simulink model "Adaptive_CT_ur10v"  (R2021b)
(part 15 of 20)

t4990 = ct{1900};
t4992 = ct{1901};
t4993 = ct{1902};
t4997 = ct{1903};
t4d = ct{1904};
t4dd = ct{1905};
t50 = ct{1906};
t5000 = ct{1907};
t5001 = ct{1908};
t5002 = ct{1909};
t5006 = ct{1910};
t501 = ct{1911};
t5010 = ct{1912};
t5011 = ct{1913};
t5012 = ct{1914};
t5013 = ct{1915};
t5014 = ct{1916};
t5018 = ct{1917};
t5019 = ct{1918};
t5020 = ct{1919};
t5022 = ct{1920};
t5025 = ct{1921};
t5026 = ct{1922};
t503 = ct{1923};
t5030 = ct{1924};
t5032 = ct{1925};
t5038 = ct{1926};
t5039 = ct{1927};
t5040 = ct{1928};
t5041 = ct{1929};
t5043 = ct{1930};
t5044 = ct{1931};
t5045 = ct{1932};
t5046 = ct{1933};
t5047 = ct{1934};
t5048 = ct{1935};
t5049 = ct{1936};
t5050 = ct{1937};
t5051 = ct{1938};
t5056 = ct{1939};
t5057 = ct{1940};
t5062 = ct{1941};
t5069 = ct{1942};
t5070 = ct{1943};
t5074 = ct{1944};
t5078 = ct{1945};
t508 = ct{1946};
t5081 = ct{1947};
t5092 = ct{1948};
t5093 = ct{1949};
t5096 = ct{1950};
t5097 = ct{1951};
t5098 = ct{1952};
t51 = ct{1953};
t5102 = ct{1954};
t5104 = ct{1955};
t5111 = ct{1956};
t5112 = ct{1957};
t5117 = ct{1958};
t5119 = ct{1959};
t5120 = ct{1960};
t5123 = ct{1961};
t5124 = ct{1962};
t5126 = ct{1963};
t5130 = ct{1964};
t5131 = ct{1965};
t5132 = ct{1966};
t5137 = ct{1967};
t5138 = ct{1968};
t514 = ct{1969};
t5144 = ct{1970};
t5148 = ct{1971};
t5149 = ct{1972};
t515 = ct{1973};
t5151 = ct{1974};
t5155 = ct{1975};
t5158 = ct{1976};
t516 = ct{1977};
t5163 = ct{1978};
t5165 = ct{1979};
t5167 = ct{1980};
t5170 = ct{1981};
t5171 = ct{1982};
t5175 = ct{1983};
t5176 = ct{1984};
t5180 = ct{1985};
t5181 = ct{1986};
t5182 = ct{1987};
t5185 = ct{1988};
t5186 = ct{1989};
t5188 = ct{1990};
t519 = ct{1991};
t5200 = ct{1992};
t5201 = ct{1993};
t5202 = ct{1994};
t5203 = ct{1995};
t5206 = ct{1996};
t5213 = ct{1997};
t5215 = ct{1998};
t5219 = ct{1999};
t5224 = ct{2000};
t5226 = ct{2001};
t523 = ct{2002};
t524 = ct{2003};
t5255 = ct{2004};
t5256 = ct{2005};
t5257 = ct{2006};
t5259 = ct{2007};
t5260 = ct{2008};
t5267 = ct{2009};
t5269 = ct{2010};
t5279 = ct{2011};
t5280 = ct{2012};
t5283 = ct{2013};
t5286 = ct{2014};
t5287 = ct{2015};
t529 = ct{2016};
t5292 = ct{2017};
t5295 = ct{2018};
t5296 = ct{2019};
t5297 = ct{2020};
t53 = ct{2021};
t530 = ct{2022};
t5305 = ct{2023};
t5306 = ct{2024};
t5315 = ct{2025};
t532 = ct{2026};
t5323 = ct{2027};
t5324 = ct{2028};
t5327 = ct{2029};
t5328 = ct{2030};
t5349 = ct{2031};
t5351 = ct{2032};
t5353 = ct{2033};
t5355 = ct{2034};
t5356 = ct{2035};
t5359 = ct{2036};
t5368 = ct{2037};
t537 = ct{2038};
t5370 = ct{2039};
t5375 = ct{2040};
t5397 = ct{2041};
t5401 = ct{2042};
t5403 = ct{2043};
t5413 = ct{2044};
t543 = ct{2045};
t5438 = ct{2046};
t544 = ct{2047};
t546 = ct{2048};
t5465 = ct{2049};
t547 = ct{2050};
t5478 = ct{2051};
t548 = ct{2052};
t5482 = ct{2053};
t55 = ct{2054};
t5503 = ct{2055};
t5505 = ct{2056};
t5514 = ct{2057};
t5515 = ct{2058};
t5517 = ct{2059};
t552 = ct{2060};
t5523 = ct{2061};
t553 = ct{2062};
t554 = ct{2063};
t56 = ct{2064};
t5619 = ct{2065};
t562 = ct{2066};
t569 = ct{2067};
t57 = ct{2068};
t570 = ct{2069};
t58 = ct{2070};
t582 = ct{2071};
t588 = ct{2072};
t589 = ct{2073};
t591 = ct{2074};
t593 = ct{2075};
t598 = ct{2076};
t5d = ct{2077};
t5dd = ct{2078};
t601 = ct{2079};
t602 = ct{2080};
t604 = ct{2081};
t608 = ct{2082};
t609 = ct{2083};
t61 = ct{2084};
t612 = ct{2085};
t614 = ct{2086};
t615 = ct{2087};
t616 = ct{2088};
t617 = ct{2089};
t623 = ct{2090};
t627 = ct{2091};
t63 = ct{2092};
t632 = ct{2093};
t634 = ct{2094};
t635 = ct{2095};
t637 = ct{2096};
t639 = ct{2097};
t641 = ct{2098};
t645 = ct{2099};
t646 = ct{2100};
t647 = ct{2101};
t648 = ct{2102};
t649 = ct{2103};
t650 = ct{2104};
t652 = ct{2105};
t653 = ct{2106};
t655 = ct{2107};
t659 = ct{2108};
t664 = ct{2109};
t670 = ct{2110};
t675 = ct{2111};
t680 = ct{2112};
t682 = ct{2113};
t687 = ct{2114};
t69 = ct{2115};
t694 = ct{2116};
t695 = ct{2117};
t696 = ct{2118};
t698 = ct{2119};
t699 = ct{2120};
t6d = ct{2121};
t6dd = ct{2122};
t703 = ct{2123};
t705 = ct{2124};
t706 = ct{2125};
t71 = ct{2126};
t711 = ct{2127};
t712 = ct{2128};
t713 = ct{2129};
t720 = ct{2130};
t721 = ct{2131};
t723 = ct{2132};
t726 = ct{2133};
t729 = ct{2134};
t731 = ct{2135};
t732 = ct{2136};
t733 = ct{2137};
t735 = ct{2138};
t736 = ct{2139};
t738 = ct{2140};
t739 = ct{2141};
t745 = ct{2142};
t746 = ct{2143};
t747 = ct{2144};
t748 = ct{2145};
t75 = ct{2146};
t752 = ct{2147};
t755 = ct{2148};
t759 = ct{2149};
t760 = ct{2150};
t761 = ct{2151};
t763 = ct{2152};
t764 = ct{2153};
t775 = ct{2154};
t776 = ct{2155};
t781 = ct{2156};
t785 = ct{2157};
t788 = ct{2158};
t789 = ct{2159};
t793 = ct{2160};
t8 = ct{2161};
t802 = ct{2162};
t806 = ct{2163};
t82 = ct{2164};
t820 = ct{2165};
t824 = ct{2166};
t828 = ct{2167};
t831 = ct{2168};
t832 = ct{2169};
t833 = ct{2170};
t838 = ct{2171};
t842 = ct{2172};
t843 = ct{2173};
t844 = ct{2174};
t846 = ct{2175};
t853 = ct{2176};
t855 = ct{2177};
t859 = ct{2178};
t861 = ct{2179};
t865 = ct{2180};
t870 = ct{2181};
t871 = ct{2182};
t873 = ct{2183};
t879 = ct{2184};
t880 = ct{2185};
t884 = ct{2186};
t885 = ct{2187};
t890 = ct{2188};
t892 = ct{2189};
t896 = ct{2190};
t897 = ct{2191};
t9 = ct{2192};
t900 = ct{2193};
t909 = ct{2194};
t910 = ct{2195};
t919 = ct{2196};
t922 = ct{2197};
t923 = ct{2198};
t927 = ct{2199};
t928 = ct{2200};
t930 = ct{2201};
t932 = ct{2202};
t937 = ct{2203};
t943 = ct{2204};
t944 = ct{2205};
t949 = ct{2206};
t952 = ct{2207};
t959 = ct{2208};
t961 = ct{2209};
t962 = ct{2210};
t963 = ct{2211};
t964 = ct{2212};
t965 = ct{2213};
t966 = ct{2214};
t969 = ct{2215};
t970 = ct{2216};
t972 = ct{2217};
t973 = ct{2218};
t981 = ct{2219};
t982 = ct{2220};
t983 = ct{2221};
t986 = ct{2222};
t989 = ct{2223};
t992 = ct{2224};
t999 = ct{2225};
t2236 = t2186./2.0;
t2237 = t2187./2.0;
t2238 = t2188./2.0;
t2239 = t2191./2.0;
t2285 = -t2269;
t2350 = t2290./2.0;
t2360 = t2310./2.0;
t2362 = -t2328;
t2466 = -t2445;
t2468 = -t2446;
t2561 = -t2545;
t2564 = t14.*t2510;
t2567 = t8.*t2514;
t2597 = -t2563;
t2601 = -t2568;
t2603 = -t2570;
t2612 = t2563./2.0;
t2616 = t2568./2.0;
t2637 = t8.*t37.*t2510;
t2643 = t14.*t37.*t2514;
t2668 = t2640./2.0;
t2669 = t2641./2.0;
t2758 = t2733.*t1dd;
t2786 = t2763.*t2d;
t2787 = t2763.*t3d;
t2788 = t2763.*t4d;
t2805 = t1392+t1748;
t2809 = t37.*t2733;
t2814 = t39.*t2733;
t2874 = -t2832;
t2887 = -t2845;
t2890 = -t2861;
t2904 = t2845./2.0;
t2906 = t2847./2.0;
t2908 = t2851./2.0;
t2909 = t1457+t1787;
t2931 = t37.*t2811;
t2958 = -t2926;
t2962 = t2930.*t1d;
t2963 = t18.*t39.*t2811;
t2973 = t2926./2.0;
t2984 = -t2957;
t2993 = -t2981;
t3084 = t3048./2.0;
t3094 = t3057.*t6d;
t3109 = t3075./2.0;
t3133 = t8.*t3089;
t3144 = -t3113;
t3164 = t3113./2.0;
t3167 = t3115./2.0;
t3184 = -t3157;
t3186 = -t3141;
t3188 = -t3142;
t3199 = t3135./2.0;
t3201 = t3138./2.0;
t3202 = t3141./2.0;
t3203 = t3142./2.0;
t3209 = -t3170;
t3210 = -t3171;
t3211 = -t3172;
t3216 = t3191.*t5d;
t3217 = -t3200;
t3218 = t3155./2.0;
t3225 = -t3206;
t3227 = t3173./2.0;
t3229 = t14.*t39.*t3089;
t3233 = t3180./2.0;
t3248 = -t3226;
t3254 = t3212./2.0;
t3269 = -t3247;
t3270 = t3249.*t1d;
t3273 = -t3252;
t3279 = -t3255;
t3280 = t3264.*(-1.0./2.0);
t3281 = t3243./2.0;
t3284 = t3247./2.0;
t3287 = t3252./2.0;
t3293 = t3255./2.0;
t3294 = -t3263;
t3297 = -t3286;
t3301 = -t3290;
t3304 = t3263./2.0;
t3309 = t3274./2.0;
t3311 = t3277./2.0;
t3314 = -t3300;
t3320 = t255.*t3089;
t3324 = t3300./2.0;
t3334 = -t3325;
t3344 = t3328.*t1dd;
t3362 = -t3350;
t3364 = t3338./2.0;
t3372 = t1978+t2036;
t3373 = -t3352;
t3379 = t39.*t3328;
t3382 = t3352./2.0;
t3385 = t37.*t3328;
t3386 = t37.*t3329;
t3389 = t3371.*t1d;
t3394 = -t3370;
t3397 = -t3374;
t3398 = t3375.*t1d;
t3402 = t3370./2.0;
t3406 = t3374./2.0;
t3410 = t3376./2.0;
t3412 = t18.*t39.*t3329;
t3419 = -t3395;
t3427 = t3392./2.0;
t3430 = t3395./2.0;
t3462 = -t3442;
t3486 = t3450.*t1d;
t3492 = -t3476;
t3497 = -t3482;
t3501 = t3476./2.0;
t3507 = t3482./2.0;
t3514 = t3489./2.0;
t3519 = t3494./2.0;
t3541 = t3512./2.0;
t3542 = -t3529;
t3561 = -t3535;
t3566 = t3533./2.0;
t3570 = t3535./2.0;
t3576 = -t3554;
t3592 = t18.*t3548;
t3594 = t18.*t3552;
t3595 = t664+t1836+t1848;
t3597 = t3552./2.0;
t3599 = t3554./2.0;
t3618 = t3572./2.0;
t3645 = -t3619;
t3646 = t3608./2.0;
t3652 = t3619./2.0;
t3654 = t3621./2.0;
t3656 = -t3633;
t3657 = t3641.*t1d;
t3658 = t3642.*t6d;
t3659 = -t3643;
t3660 = t3631./2.0;
t3663 = t3632./2.0;
t3664 = t3633./2.0;
t3672 = t3643./2.0;
t3689 = t3653./2.0;
t3691 = t3655./2.0;
t3692 = t3666.*t1d;
t3695 = t18.*t3669;
t3696 = -t3671;
t3698 = t3662./2.0;
t3700 = t3665./2.0;
t3703 = -t3679;
t3705 = t1053+t3092;
t3706 = t1054+t3093;
t3707 = t3667./2.0;
t3711 = t3671./2.0;
t3713 = t3673./2.0;
t3717 = t3679./2.0;
t3718 = t3680./2.0;
t3723 = -t3702;
t3735 = t3694./2.0;
t3742 = t3702./2.0;
t3759 = t3719./2.0;
t3773 = -t3749;
t3782 = (t8.*t3709)./2.0;
t3790 = t3749./2.0;
t3793 = -t3772;
t3797 = t14.*t39.*t3709;
t3798 = -t3788;
t3801 = t3772./2.0;
t3816 = -t3795;
t3823 = -t3802;
t3824 = t3795./2.0;
t3834 = t3802./2.0;
t3836 = -t3815;
t3844 = t3815./2.0;
t3847 = t3818./2.0;
t3856 = t3825./2.0;
t3859 = t3829./2.0;
t3862 = t2160+t2575;
t3865 = -t3841;
t3870 = (t14.*t3799)./2.0;
t3873 = t3841./2.0;
t3881 = t8.*t39.*t3799;
t3884 = t2159+t2605;
t3898 = -t3868;
t3909 = t3868./2.0;
t3911 = t255.*t3709;
t3915 = -t3882;
t3916 = -t3899;
t3925 = -t3908;
t3930 = t3882./2.0;
t3945 = -t3912;
t3951 = -t3934;
t3953 = t3904./2.0;
t3955 = -t3938;
t3961 = t3912./2.0;
t3981 = t3942./2.0;
t3985 = -t3971;
t3995 = t3964./2.0;
t3996 = t3966./2.0;
t3998 = t3969./2.0;
t4000 = -t3991;
t4013 = -t4008;
t4015 = t330.*t3799;
t4031 = t4020.*t2d;
t4032 = t4020.*t3d;
t4033 = t4020.*t4d;
t4037 = -t4022;
t4039 = t4022./2.0;
t4043 = -t4036;
t4051 = t4036./2.0;
t4060 = -t4057;
t4062 = t4054.*t1d;
t4079 = -t4070;
t4100 = t4092.*t1d;
t4104 = t18.*t4093;
t4105 = t18.*t4094;
t4106 = -t4094;
t4110 = t4093./2.0;
t4111 = t4094./2.0;
t4181 = t4161./2.0;
t4184 = t4163./2.0;
t4205 = t4197.*t1d;
t4209 = t4190./2.0;
t4210 = t4191./2.0;
t4211 = t4198.*t1d;
t4232 = t8.*t4206;
t4234 = -t4213;
t4239 = t4213./2.0;
t4240 = t4214./2.0;
t4244 = t14.*t4218;
t4247 = t4223./2.0;
t4250 = t4224./2.0;
t4259 = t4235./2.0;
t4261 = -t4242;
t4264 = -t4246;
t4265 = t4238./2.0;
t4269 = t4241./2.0;
t4270 = t4242./2.0;
t4271 = t4243./2.0;
t4272 = t4258.*t5d;
t4275 = t4246./2.0;
t4277 = t4249./2.0;
t4278 = t14.*t39.*t4206;
t4279 = t4254.*t2d;
t4280 = t4254.*t3d;
t4281 = t4254.*t4d;
t4286 = t4253./2.0;
t4291 = t4260./2.0;
t4300 = t8.*t39.*t4218;
t4306 = t4284./2.0;
t4307 = t4285./2.0;
t4308 = -t4292;
t4315 = t4292./2.0;
t4316 = t4293./2.0;
t4318 = t4295./2.0;
t4320 = t4298./2.0;
t4323 = t4303./2.0;
t4338 = t4311./2.0;
t4339 = t4319./2.0;
t4343 = t255.*t4206;
t4345 = -t4336;
t4347 = t4328./2.0;
t4350 = t4336./2.0;
t4352 = t4341.*t1d;
t4369 = t330.*t4218;
t4370 = t4360.*t1d;
t4373 = t18.*t4363;
t4374 = -t4366;
t4375 = t4358./2.0;
t4376 = t4359./2.0;
t4377 = t4363./2.0;
t4378 = t4364./2.0;
t4387 = t18.*t4364.*(-1.0./2.0);
t4390 = t4388.*t2d;
t4391 = t4388.*t3d;
t4392 = t4388.*t4d;
t4400 = -t4396;
t4401 = t2546+t3450;
t4412 = -t4407;
t4415 = t4407./2.0;
t4419 = t4411./2.0;
t4422 = t3048+t3075;
t4435 = t4423.*t2dd;
t4437 = t4423.*t3dd;
t4439 = t4423.*t4dd;
t4441 = t4420./2.0;
t4446 = -t4432;
t4455 = t4432./2.0;
t4456 = t4433./2.0;
t4462 = t14.*t4452;
t4463 = t8.*t4453;
t4465 = t4445./2.0;
t4481 = -t4476;
t4484 = t8.*t39.*t4452;
t4485 = t14.*t39.*t4453;
t4490 = t37.*t4474;
t4492 = t3155+t3158;
t4498 = t18.*t39.*t4474;
t4505 = t1682+t1722+t2002+t2015;
t4511 = t255.*t4453;
t4516 = t330.*t4452;
t4520 = t4514.*t1d;
t4521 = t4515./2.0;
t4522 = -t4517;
t4527 = t4519./2.0;
t4530 = t2187+t2534+t2566;
t4535 = -t4154.*(t745-t747);
t4545 = t4154.*(t745-t747);
t4555 = t4546.*(-1.0./2.0);
t4559 = t4546./2.0;
t4564 = -t4562;
t4567 = -t4565;
t4569 = t4565./2.0;
t4571 = (t1874.*t4154)./2.0;
t4577 = t4568./2.0;
t4586 = -t4576;
t4590 = t14.*t4578;
t4593 = t4576./2.0;
t4594 = t8.*t4575;
t4601 = -t4588;
t4603 = t8.*t4587;
t4605 = t4583./2.0;
t4609 = t4588./2.0;
t4616 = t4611.*t2d;
t4617 = t4611.*t3d;
t4618 = t4611.*t4d;
t4625 = -t4621;
t4630 = t4622.*t1d;
t4637 = -t2d.*(t3350-t3369);
t4638 = -t3d.*(t3350-t3369);
t4639 = -t4d.*(t3350-t3369);
t4644 = -t4636;
t4649 = -t4634;
t4651 = -t4646;
t4653 = t1899+t1900+t1901+t2328;
t4656 = t4634./2.0;
t4657 = t4635./2.0;
t4658 = -t4650;
t4661 = t4654.*t2d;
t4662 = t4654.*t3d;
t4663 = t4654.*t4d;
t4674 = t2270.*t4154;
t4689 = -t4685;
t4690 = -t2d.*(t3442+(t14.*(t1864-t2028))./2.0);
t4691 = -t3d.*(t3442+(t14.*(t1864-t2028))./2.0);
t4692 = -t4d.*(t3442+(t14.*(t1864-t2028))./2.0);
t4709 = -t4702;
t4711 = t4701./2.0;
t4712 = t4702./2.0;
t4726 = t4717./2.0;
t4731 = t4723./2.0;
t4733 = t2934+t4034;
t4734 = t4724./2.0;
t4735 = t37.*t4710;
t4736 = t4725./2.0;
t4740 = t2529.*t4154;
t4745 = t18.*t39.*t4710;
t4748 = t4730./2.0;
t4752 = t4741./2.0;
t4754 = t4744./2.0;
t4755 = t2918+t4056;
t4761 = -t1d.*(t2893-t4056);
t4769 = -t4427.*(t745-t747);
t4772 = t4766.*(-1.0./2.0);
t4773 = t2914+t4083;
t4774 = t201+t332+t1382+t1397+t1654+t1660+t2108;
t4782 = t4427.*(t745-t747).*(-1.0./2.0);
t4788 = -t4784;
t4793 = t14.*t4777;
t4797 = t3572+t3621;
t4816 = t8.*t39.*t4777;
t4824 = (t1874.*t4427)./2.0;
t4826 = t8.*t4810;
t4833 = -t4830;
t4839 = t14.*t39.*t4810;
t4850 = t330.*t4777;
t4857 = t255.*t4810;
t4868 = t2270.*t4427;
t4872 = t3081.*t4154;
t4877 = -t4873;
t4879 = t4154.*(t503.*1.383e-1+t731+t981+t999);
t4892 = -t4890;
t4894 = t3810+t3829;
t4897 = t2529.*t4427;
t4900 = -t4898;
t4902 = t4898./2.0;
t4913 = t2132+t2162+t2591+t2604;
t4914 = t2150+t2196+t2552+t2573;
t4916 = t3868+t3896;
t4933 = (t3404.*t4154)./2.0;
t4936 = -t4934;
t4947 = -t4942;
t4948 = -t4943;
t4962 = t2810+t3112+t3193;
t4968 = t2773+t2871+t3527;
t4969 = t3081.*t4427;
t4971 = t3734.*t4154;
t4977 = t4427.*(t503.*1.383e-1+t731+t981+t999);
t4978 = t2812+t2875+t3565;
t4983 = t3821.*t4154;
t4991 = -t4984;
t4995 = t4984./2.0;
t4996 = t2851+t3275+t3278;
t5005 = t1249+t1458+t1507+t3005+t3006;
t5016 = -t5d.*(-t2972+t3286+(t8.*t39.*(t1743-t1783))./2.0);
t5017 = t5d.*(-t2972+t3286+(t8.*t39.*(t1743-t1783))./2.0);
t5021 = t3404.*t4427;
t5028 = t5022./2.0;
t5031 = t4049.*t4154;
t5034 = -t5032;
t5037 = t1537+t2024+t2678+t3921;
t5042 = t1904+t2419+t2536+t3600;
t5053 = t37.*t5039;
t5054 = t8.*t5045;
t5055 = t14.*t5046;
t5058 = t2329+t2791+t2792+t2793;
t5061 = t18.*t39.*t5039;
t5063 = t14.*t5049;
t5064 = t8.*t5050;
t5066 = t5062.*(-1.0./2.0);
t5068 = (t3686.*t4427)./2.0;
t5071 = -t1d.*(-t1590+t2042+t3934+(t18.*t37.*(t544-t1021+t330.*(t100-t364)))./2.0);
t5076 = t3734.*t4427;
t5077 = (t4130.*t4154)./2.0;
t5079 = t1572+t2072+t2710+t3986;
t5084 = -t5078;
t5100 = t5096./2.0;
t5105 = -t5102;
t5107 = -t5d.*(-t612-t944+t1336+t2229+t2811+(t8.*t494.*(t100-t364))./2.0+(t14.*t39.*(t844-t1156))./2.0);
t5109 = t5102./2.0;
t5113 = t5d.*(-t612-t944+t1336+t2229+t2811+(t8.*t494.*(t100-t364))./2.0+(t14.*t39.*(t844-t1156))./2.0);
t5121 = t14.*t5111;
t5122 = t14.*t5112;
t5125 = t635+t1428+t1833+t1846+t2789+t2927;
t5127 = t5124.*(-1.0./2.0);
t5139 = -t5137;
t5142 = t5130./2.0;
t5143 = t5138.*t5d;
t5145 = t8.*t39.*t5111;
t5146 = t8.*t39.*t5112;
t5153 = -t5149;
t5159 = -t5155;
t5162 = t5158.*(-1.0./2.0);
t5164 = t4154.*t4333;
t5169 = -t5165;
t5173 = t5165./2.0;
t5174 = t5170.*(-1.0./2.0);
t5179 = t4049.*t4427;
t5183 = t330.*t5111;
t5184 = t330.*t5112;
t5190 = -t5188;
t5204 = t713+t1489+t1849+t1959+t2940+t3028;
t5207 = t5203.*t5d;
t5209 = t5206.*t5d;
t5214 = t4154.*t4427;
t5217 = -t5215;
t5221 = t2321+t2385+t4710;
t5222 = t2304+t2368+t4732;
t5225 = t4333.*t4427;
t5228 = t5226./2.0;
t5230 = -t6d.*(t680-t989+t1395-t2455+t3328+(t627.*(t101-t401))./2.0+(t330.*(t952-t1028))./2.0);
t5231 = t6d.*(t680-t989+t1395-t2455+t3328+(t627.*(t101-t401))./2.0+(t330.*(t952-t1028))./2.0);
t5234 = t2491+t2493+t3493+t3494;
t5235 = t2491+t2493+t3489+t3490;
t5243 = t4403+t4411;
t5261 = -t5259;
t5262 = t5259./2.0;
t5263 = -t5260;
t5266 = t5260./2.0;
t5268 = t1789+t1814+t5039;
t5271 = t5269.*t1d;
t5276 = t1478+t1707+t1724+t2898+t3179+t3213;
t5282 = t5279.*t5d;
t5284 = t5280./2.0;
t5288 = -t5286;
t5291 = t5286./2.0;
t5293 = t5287./2.0;
t5299 = t5295./2.0;
t5303 = t5296./2.0;
t5304 = t5297./2.0;
t5307 = t5305./2.0;
t5311 = t501+t2764+t2765+t2766+t4312;
t5314 = -t5306;
t5322 = t5306./2.0;
t5325 = -t6d.*(t682+t1513-t1939+t1985-t2734-t2988+(t330.*(t582+t616-t761+t18.*t37.*(t100-t364)))./2.0);
t5329 = t6d.*(t682+t1513-t1939+t1985-t2734-t2988+(t330.*(t582+t616-t761+t18.*t37.*(t100-t364)))./2.0);
t5330 = t711+t1514+t1936+t2010+t2733+t3037+t3050;
t5335 = t5328.*t2d;
t5336 = t5328.*t3d;
t5337 = t5328.*t4d;
t5345 = t1863+t1868+t5180;
t5346 = t245+t2800+t2801+t2802+t4372;
t5352 = t964+t1903+t2367+t2403+t3540+t3581;
t5357 = t5356.*(-1.0./2.0);
t5358 = t2894+t2950+t4040+t4052;
t5361 = t1004+t2004+t2366+t2475+t3651+t3699;
t5362 = -t1d.*(t2933-t4040-t4052+(t342.*(t544-t1021+t330.*(t100-t364)))./2.0);
t5363 = t1d.*(t2933-t4040-t4052+(t342.*(t544-t1021+t330.*(t100-t364)))./2.0);
t5366 = t3032+t3043+t4970;
t5369 = t14.*t5368;
t5373 = t8.*t5370;
t5374 = t8.*t39.*t5368;
Y = ft_10({t100,t1007,t101,t1015,t1016,t1017,t1021,t1026,t1028,t1031,t1035,t1036,t104,t1044,t1045,t1046,t1047,t1048,t1049,t1055,t106,t1066,t1068,t1069,t107,t1070,t1071,t1079,t108,t1080,t1081,t1082,t1083,t1084,t1085,t1086,t1087,t1093,t1094,t1096,t1097,t1098,t1106,t1108,t1109,t111,t1110,t112,t1121,t1122,t1123,t1126,t1128,t1129,t113,t1133,t1134,t1135,t1137,t1138,t1139,t1140,t1147,t1148,t1155,t1156,t1160,t1162,t1172,t1174,t1183,t1184,t1185,t1186,t1187,t1189,t1193,t1196,t12,t1203,t1208,t1209,t1210,t1211,t1222,t1224,t1225,t1226,t1227,t1230,t1236,t1237,t1238,t124,t1245,t1246,t1247,t1248,t1264,t1265,t1266,t1268,t127,t1271,t1272,t1273,t128,t1281,t1284,t1287,t1288,t1289,t1297,t1298,t13,t1302,t131,t1311,t1312,t1316,t1317,t132,t1321,t1328,t1331,t1332,t1333,t1334,t1335,t134,t1355,t1356,t1357,t1358,t136,t1368,t137,t1375,t1378,t138,t1399,t14,t1400,t1403,t1408,t1410,t1413,t1419,t1420,t1427,t1434,t1440,t1461,t1464,t1465,t1468,t1470,t1472,t1475,t1479,t1485,t1492,t1497,t1499,t15,t150,t1500,t1501,t1503,t1504,t1516,t1517,t1518,t1519,t152,t1520,t1521,t1525,t1526,t1528,t1529,t1532,t1534,t1535,t1536,t1537,t1547,t155,t156,t1569,t1571,t1574,t1578,t1579,t158,t1580,t1585,t1586,t1588,t1589,t159,t1590,t1597,t1599,t1606,t1607,t1609,t1610,t1615,t1617,t1618,t162,t163,t1636,t164,t1645,t1647,t1648,t1649,t165,t1650,t1651,t1652,t1653,t1659,t1663,t1671,t1674,t1677,t1678,t1680,t1683,t1685,t1686,t1687,t1692,t1699,t1701,t1704,t1706,t1709,t171,t1710,t1713,t1714,t1715,t173,t1733,t1736,t1738,t174,t1740,t1741,t1742,t1743,t175,t1751,t1754,t1755,t1758,t1759,t1760,t177,t1776,t1780,t1783,t1784,t1786,t1790,t1792,t1797,t1799,t18,t1800,t1803,t1807,t1813,t1815,t1816,t1818,t1827,t1829,t1832,t1835,t1837,t1838,t1840,t1844,t1848,t1849,t1862,t1864,t1866,t1867,t187,t1872,t1873,t1874,t1875,t1885,t1888,t1889,t1890,t1891,t1892,t19,t1903,t1905,t191,t1916,t1919,t1920,t1921,t1925,t1929,t1930,t1933,t1935,t1938,t1939,t1940,t1944,t1945,t1956,t1957,t1958,t1960,t1961,t1962,t1963,t1964,t1965,t1966,t1967,t1968,t1969,t1970,t1971,t1973,t1976,t1977,t1983,t1984,t1988,t199,t1992,t1993,t1995,t1996,t1999,t1d,t1dd,t200,t2001,t2005,t2009,t2012,t2013,t2018,t2021,t2022,t2026,t2028,t2031,t2033,t2044,t2053,t2054,t2059,t206,t2060,t2061,t2062,t2068,t2070,t2074,t2075,t2079,t2080,t2081,t2085,t2086,t2087,t2088,t2090,t2093,t2098,t2099,t21,t2100,t2101,t2104,t2112,t2113,t2115,t2117,t2119,t2122,t2123,t2124,t2126,t2128,t2129,t2130,t2136,t2140,t2141,t2142,t2143,t2144,t2145,t2147,t215,t2155,t2156,t2167,t2168,t2169,t2170,t2171,t2173,t2174,t2178,t2180,t2184,t2186,t2187,t2188,t2189,t219,t2190,t2193,t2198,t22,t220,t2203,t2204,t2205,t2206,t2210,t2213,t2214,t2215,t2222,t2223,t2224,t2225,t2233,t2235,t2236,t2237,t2238,t2239,t2243,t2246,t2247,t2249,t2259,t226,t2266,t2270,t2279,t2281,t2285,t2286,t2289,t229,t2290,t2292,t2293,t2294,t2295,t2296,t23,t2300,t2304,t2305,t2306,t2308,t2310,t2311,t2317,t232,t2322,t2327,t233,t2330,t2331,t2332,t2339,t2340,t2344,t2346,t2348,t2349,t2350,t2351,t2352,t2353,t2354,t2355,t2356,t2357,t2358,t2359,t2360,t2361,t2362,t2363,t2364,t2368,t2369,t2371,t2372,t2373,t2374,t2375,t2376,t2378,t2379,t2380,t2382,t2384,t2386,t2387,t2393,t2395,t2398,t2399,t24,t2400,t2401,t2402,t2405,t2406,t2407,t2409,t2412,t2414,t2416,t2421,t2427,t2428,t2430,t2431,t2433,t2434,t2438,t244,t2460,t2463,t2466,t2467,t2468,t247,t2471,t2472,t2473,t2475,t2476,t2477,t2478,t2479,t2486,t2488,t2490,t2492,t2497,t2499,t25,t2500,t2501,t2502,t2503,t2504,t2506,t2507,t2508,t2509,t2510,t2511,t2512,t2513,t2514,t2520,t2523,t2526,t2527,t2528,t2532,t2533,t2534,t2544,t2549,t255,t2550,t2557,t256,t2561,t2562,t2563,t2564,t2567,t2568,t2570,t2574,t2576,t2578,t2583,t2585,t2586,t2587,t2588,t2589,t2593,t2596,t2597,t26,t2601,t2602,t2603,t2606,t2608,t2610,t2612,t2614,t2616,t2617,t2619,t2625,t2626,t2627,t2630,t2637,t2640,t2641,t2642,t2643,t2644,t2645,t2647,t2648,t2652,t2654,t2655,t2658,t2659,t2661,t2664,t2665,t2666,t2668,t2669,t2673,t2675,t2679,t2681,t2682,t2689,t2690,t2691,t2696,t2699,t27,t2703,t2705,t2707,t2708,t2709,t2711,t2718,t2719,t2721,t2722,t2724,t2731,t2734,t2737,t2743,t2744,t2745,t2747,t2749,t2755,t2758,t2759,t2772,t2775,t2776,t2777,t2779,t2780,t2781,t2782,t2786,t2787,t2788,t2790,t2795,t2796,t2797,t2798,t2805,t2807,t2808,t2809,t2810,t2813,t2814,t2815,t2816,t2828,t2829,t2830,t2835,t2841,t2842,t2843,t2845,t2847,t2848,t2853,t2857,t2862,t2864,t2865,t2867,t2868,t2870,t2873,t2874,t2876,t2878,t2882,t2883,t2884,t2885,t2887,t2890,t2891,t2895,t2899,t29,t2900,t2901,t2902,t2904,t2906,t2908,t2909,t2915,t2925,t2929,t2931,t2935,t2936,t2937,t2940,t2946,t2947,t2951,t2953,t2954,t2956,t2958,t2959,t2961,t2962,t2963,t2966,t2967,t2968,t2970,t2971,t2972,t2973,t2982,t2983,t2984,t2985,t2988,t2989,t299,t2991,t2992,t2993,t2994,t2995,t2996,t2997,t2998,t2999,t2d,t2dd,t30,t3000,t3003,t3004,t3007,t3009,t301,t3010,t3011,t3012,t3013,t3014,t3017,t3018,t3029,t3035,t3052,t3057,t3058,t3059,t3065,t3066,t3069,t3073,t3076,t3078,t3079,t308,t3080,t3081,t3082,t3083,t3084,t3085,t3086,t3087,t3088,t3090,t3094,t3098,t3099,t31,t3100,t3101,t3104,t3106,t3107,t3108,t3109,t3112,t3115,t3120,t3123,t3124,t3125,t3126,t3129,t3130,t3133,t3135,t3136,t3137,t3138,t3139,t3140,t3143,t3144,t3146,t315,t3151,t3155,t3156,t3159,t3161,t3162,t3163,t3164,t3165,t3166,t3167,t317,t3170,t3171,t3172,t3173,t3174,t3175,t3176,t3177,t318,t3180,t3181,t3182,t3183,t3184,t3185,t3186,t3187,t3188,t319,t3192,t3195,t3196,t3197,t3199,t3201,t3202,t3203,t3204,t3205,t3209,t3210,t3211,t3212,t3214,t3215,t3216,t3217,t3218,t3219,t3220,t3221,t3225,t3227,t3228,t3229,t3230,t3231,t3232,t3233,t3234,t3236,t3237,t3239,t3240,t3241,t3243,t3244,t3246,t3248,t325,t3251,t3254,t3255,t3257,t3258,t3260,t3264,t3265,t3266,t3267,t3268,t3269,t3270,t3271,t3272,t3273,t3274,t3276,t3277,t3279,t3280,t3281,t3282,t3283,t3284,t3285,t3287,t3288,t3289,t329,t3291,t3292,t3293,t3294,t3297,t3298,t330,t3300,t3301,t3304,t3306,t3308,t3309,t3310,t3311,t3312,t3314,t3316,t3318,t3320,t3321,t3322,t3324,t3326,t3327,t3329,t333,t3330,t3331,t3332,t3334,t3335,t3338,t3339,t3340,t3344,t3348,t3349,t3350,t3351,t3354,t3355,t3358,t3359,t3360,t3362,t3364,t3365,t3369,t3370,t3372,t3373,t3374,t3376,t3377,t3378,t3379,t3380,t3381,t3382,t3383,t3384,t3385,t3386,t3387,t3388,t3389,t3390,t3391,t3392,t3394,t3395,t3397,t3398,t3399,t34,t3400,t3401,t3402,t3404,t3405,t3406,t341,t3410,t3412,t3414,t3415,t3416,t3417,t3419,t342,t3421,t3426,t3427,t3429,t343,t3430,t3431,t3432,t3439,t3440,t3442,t3445,t3452,t3456,t3457,t3458,t3459,t346,t3460,t3461,t3462,t3468,t3469,t347,t3472,t3473,t3474,t3475,t3477,t3478,t3483,t3486,t3491,t3492,t3497,t3499,t3501,t3502,t3503,t3506,t3507,t3509,t3510,t3512,t3514,t3515,t3516,t3517,t3518,t3519,t3521,t3524,t3525,t3526,t3532,t3533,t3535,t3536,t3537,t3538,t3539,t3541,t3542,t3543,t3544,t3547,t3548,t3549,t3552,t3557,t3558,t3559,t3561,t3566,t3570,t3571,t3574,t3575,t3576,t3578,t3579,t3580,t3582,t3583,t3586,t3587,t3588,t3590,t3591,t3592,t3594,t3595,t3597,t3598,t3599,t36,t3601,t3602,t3603,t3604,t3605,t3607,t3608,t3609,t3610,t3611,t3613,t3617,t3618,t3620,t3622,t3623,t3624,t3625,t3628,t3630,t3631,t3632,t3633,t3634,t3635,t3636,t3637,t3638,t3639,t364,t3640,t3643,t3645,t3646,t3647,t3648,t365,t3650,t3652,t3653,t3654,t3655,t3656,t3657,t3658,t3659,t3660,t3662,t3663,t3664,t3665,t3667,t3668,t3669,t3670,t3671,t3672,t3673,t368,t3680,t3682,t3683,t3684,t3685,t3686,t3687,t3689,t3691,t3692,t3693,t3694,t3695,t3696,t3698,t37,t3700,t3701,t3702,t3703,t3705,t3706,t3707,t3708,t3710,t3711,t3712,t3713,t3715,t3716,t3717,t3718,t3719,t3723,t3732,t3734,t3735,t3739,t3741,t3742,t3745,t3747,t3750,t3751,t3754,t3755,t3756,t3757,t3759,t3762,t3770,t3771,t3772,t3773,t3780,t3781,t3782,t3785,t3787,t3788,t3789,t3790,t3793,t3795,t3797,t3798,t38,t3800,t3801,t3804,t3805,t3807,t3808,t3809,t3812,t3816,t3817,t3818,t3819,t3821,t3822,t3823,t3824,t3825,t3826,t3832,t3833,t3834,t3836,t3838,t3839,t3840,t3843,t3844,t3847,t3848,t3856,t3858,t3859,t3861,t3862,t3863,t3865,t3866,t3867,t3870,t3872,t3873,t3874,t3875,t3880,t3881,t3882,t3883,t3885,t3886,t3887,t3888,t3889,t3890,t3892,t3894,t3898,t3899,t39,t3900,t3901,t3903,t3904,t3909,t3911,t3912,t3913,t3915,t3916,t3917,t3919,t392,t3923,t3924,t3925,t3927,t3928,t393,t3930,t3931,t3932,t3933,t3935,t3936,t3937,t3942,t3943,t3944,t3945,t3951,t3953,t3955,t3956,t3958,t3960,t3961,t3962,t3964,t3965,t3966,t3967,t3969,t3971,t3972,t3975,t3976,t3977,t3978,t3979,t3981,t3982,t3984,t3985,t3989,t3990,t3991,t3992,t3994,t3995,t3996,t3997,t3998,t3999,t3d,t3dd,t4000,t4001,t4002,t4003,t4005,t4006,t4007,t4009,t401,t4010,t4011,t4012,t4013,t4015,t4016,t4017,t402,t4022,t4023,t4025,t4026,t4027,t403,t4031,t4032,t4033,t4036,t4037,t4038,t4039,t404,t4041,t4042,t4043,t4046,t4047,t4048,t4049,t4050,t4051,t4053,t4059,t4060,t4062,t4065,t4068,t4069,t4071,t4074,t4078,t4079,t4084,t4087,t4093,t4094,t4095,t4096,t41,t4100,t4101,t4102,t4104,t4105,t4106,t4108,t4110,t4111,t4115,t4117,t4118,t4121,t4122,t4125,t4127,t4128,t4130,t4131,t4133,t4136,t4137,t4139,t4143,t4146,t4147,t4149,t4151,t4152,t4154,t4155,t4156,t4157,t4159,t4161,t4163,t4164,t4166,t4167,t4168,t4170,t4171,t4172,t4174,t4176,t4178,t418,t4181,t4182,t4183,t4184,t4185,t4186,t4187,t4188,t4189,t419,t4190,t4191,t4192,t4193,t4195,t4196,t42,t420,t4200,t4201,t4203,t4204,t4205,t4209,t4210,t4211,t4212,t4214,t4221,t4223,t4224,t4226,t4227,t4228,t4229,t4230,t4231,t4232,t4233,t4234,t4235,t4236,t4237,t4238,t4239,t4240,t4241,t4243,t4244,t4247,t4249,t425,t4250,t4251,t4252,t4253,t4255,t4256,t4259,t4260,t4261,t4264,t4265,t4266,t4267,t4269,t4270,t4271,t4272,t4275,t4277,t4278,t4279,t4280,t4281,t4282,t4283,t4284,t4285,t4286,t4290,t4291,t4292,t4293,t4295,t4296,t4298,t4299,t4300,t4301,t4303,t4304,t4306,t4307,t4308,t4309,t431,t4311,t4315,t4316,t4317,t4318,t4319,t4320,t4321,t4323,t4324,t4325,t4327,t4328,t4330,t4331,t4332,t4335,t4337,t4338,t4339,t434,t4343,t4345,t4347,t4348,t4350,t4352,t4353,t4358,t4359,t4361,t4363,t4364,t4367,t4369,t437,t4370,t4371,t4373,t4374,t4375,t4376,t4377,t4378,t4387,t4390,t4391,t4392,t4394,t4395,t4399,t4400,t4401,t4402,t4404,t4406,t4408,t441,t4410,t4411,t4412,t4413,t4415,t4419,t442,t4420,t4421,t4422,t4423,t4424,t4427,t4428,t4429,t443,t4430,t4431,t4433,t4435,t4437,t4439,t4441,t4444,t4445,t4446,t4450,t4451,t4454,t4455,t4456,t4457,t4459,t446,t4460,t4461,t4462,t4463,t4464,t4465,t4467,t4468,t4470,t4473,t4474,t4475,t4476,t4479,t4480,t4481,t4483,t4484,t4485,t4487,t4488,t4490,t4491,t4492,t4493,t4494,t4498,t4500,t4503,t4505,t4506,t4508,t4509,t4511,t4515,t4516,t4519,t4520,t4521,t4522,t4526,t4527,t4528,t453,t4530,t4531,t4532,t4533,t4534,t4537,t4538,t4539,t454,t4540,t4541,t4542,t4543,t4545,t4546,t4547,t4548,t4550,t4551,t4552,t4553,t4556,t4559,t4561,t4564,t4567,t4568,t4569,t4571,t4572,t4575,t4576,t4577,t4578,t4579,t4582,t4583,t4586,t4587,t4588,t459,t4590,t4591,t4593,t4594,t4595,t4596,t4599,t4601,t4603,t4604,t4605,t4606,t4607,t4608,t4609,t4612,t4616,t4617,t4618,t4623,t4625,t4626,t4627,t4630,t4631,t4633,t4634,t4635,t4636,t4637,t4638,t4639,t4640,t4641,t4642,t4644,t4645,t4646,t4647,t4648,t4649,t4650,t4651,t4652,t4653,t4655,t4656,t4657,t4658,t4659,t4661,t4662,t4663,t4664,t4665,t4666,t4668,t4670,t4672,t4673,t4674,t4675,t4677,t4678,t4679,t4681,t4684,t4686,t4689,t4690,t4691,t4692,t4694,t4695,t4699,t470,t4700,t4701,t4703,t4704,t4705,t4707,t4708,t4709,t4711,t4712,t4713,t4714,t4715,t4716,t4717,t4720,t4721,t4722,t4723,t4724,t4725,t4726,t4727,t4730,t4731,t4733,t4734,t4735,t4736,t4737,t4738,t4739,t4740,t4741,t4744,t4745,t4747,t4748,t4752,t4754,t4757,t4758,t4759,t4760,t4761,t4762,t4765,t4766,t4767,t4768,t4769,t4770,t4771,t4772,t4774,t4776,t4778,t478,t4780,t4782,t4783,t4784,t4785,t4786,t4788,t4792,t4793,t4794,t4795,t4796,t4797,t4798,t48,t4807,t4813,t4815,t4816,t4817,t4822,t4824,t4825,t4826,t4828,t4829,t4830,t4831,t4833,t4836,t4837,t4838,t4839,t4840,t4841,t4843,t4845,t4846,t4849,t4850,t4851,t4855,t4856,t4857,t4858,t486,t4860,t4861,t4862,t4865,t4867,t4868,t487,t4870,t4872,t4873,t4874,t4875,t4877,t4878,t4879,t488,t4881,t4883,t4887,t4888,t4889,t4890,t4891,t4892,t4894,t4895,t4896,t4897,t4900,t4902,t4913,t4914,t4915,t4916,t4917,t492,t4920,t4922,t4923,t4925,t4926,t4929,t493,t4930,t4931,t4933,t4934,t4935,t4936,t4938,t494,t4941,t4943,t4946,t4947,t4949,t495,t4950,t4951,t4952,t4953,t4954,t4955,t4956,t4957,t4958,t4959,t496,t4960,t4962,t4967,t4968,t4969,t497,t4971,t4975,t4977,t4978,t4979,t4981,t4983,t4985,t4990,t4991,t4992,t4993,t4995,t4996,t4997,t4d,t4dd,t50,t5000,t5001,t5002,t5005,t5006,t5010,t5011,t5012,t5013,t5014,t5016,t5017,t5018,t5019,t5020,t5021,t5022,t5025,t5026,t5028,t5030,t5031,t5034,t5037,t5038,t5040,t5041,t5043,t5044,t5045,t5046,t5047,t5048,t5049,t5050,t5051,t5053,t5054,t5055,t5056,t5057,t5058,t5061,t5062,t5063,t5064,t5066,t5068,t5069,t5070,t5071,t5074,t5076,t5077,t5079,t508,t5081,t5084,t5092,t5093,t5096,t5097,t5098,t51,t5100,t5102,t5104,t5105,t5109,t5113,t5117,t5119,t5120,t5121,t5122,t5123,t5124,t5125,t5126,t5127,t5130,t5131,t5132,t5139,t514,t5142,t5143,t5144,t5145,t5146,t5148,t5149,t515,t5151,t5153,t5155,t5158,t5159,t516,t5162,t5163,t5164,t5165,t5167,t5169,t5170,t5171,t5173,t5174,t5175,t5176,t5179,t5181,t5182,t5183,t5184,t5185,t5186,t519,t5190,t5200,t5201,t5202,t5207,t5209,t5213,t5214,t5217,t5219,t5222,t5224,t5225,t5226,t5228,t523,t5231,t5234,t5235,t524,t5243,t5255,t5256,t5257,t5261,t5262,t5263,t5266,t5267,t5268,t5271,t5276,t5280,t5282,t5283,t5284,t5287,t5288,t529,t5291,t5292,t5293,t5295,t5296,t5297,t5299,t53,t530,t5303,t5304,t5305,t5307,t5314,t5315,t532,t5322,t5323,t5324,t5327,t5329,t5330,t5335,t5336,t5337,t5345,t5349,t5351,t5353,t5355,t5356,t5357,t5359,t5361,t5363,t5366,t5368,t5369,t537,t5370,t5373,t5374,t5375,t5397,t5401,t5403,t5413,t543,t5438,t544,t546,t5465,t547,t5478,t548,t5482,t55,t5503,t5505,t5514,t5515,t5517,t552,t5523,t553,t554,t56,t5619,t562,t569,t57,t570,t58,t582,t588,t589,t591,t593,t598,t5d,t5dd,t601,t602,t604,t608,t609,t61,t614,t615,t616,t617,t623,t627,t63,t632,t634,t637,t639,t641,t645,t646,t647,t648,t649,t650,t652,t653,t655,t659,t670,t675,t687,t69,t694,t695,t696,t698,t699,t6d,t6dd,t703,t705,t706,t71,t711,t712,t720,t721,t723,t726,t729,t732,t733,t735,t736,t738,t739,t745,t746,t747,t748,t75,t752,t755,t759,t760,t761,t763,t764,t775,t776,t781,t785,t788,t789,t793,t8,t802,t806,t82,t820,t824,t828,t831,t832,t833,t838,t842,t843,t844,t846,t853,t855,t859,t861,t865,t870,t871,t873,t879,t880,t884,t885,t890,t892,t896,t897,t9,t900,t909,t910,t919,t922,t923,t927,t928,t930,t932,t937,t943,t949,t952,t959,t961,t962,t963,t964,t965,t966,t969,t970,t972,t973,t982,t983,t986,t992});
end
function Y = ft_10(ct)
t100 = ct{1};
t1007 = ct{2};
t101 = ct{3};
t1015 = ct{4};
t1016 = ct{5};
t1017 = ct{6};
t1021 = ct{7};
t1026 = ct{8};
t1028 = ct{9};
t1031 = ct{10};
t1035 = ct{11};
t1036 = ct{12};
t104 = ct{13};
t1044 = ct{14};
t1045 = ct{15};
t1046 = ct{16};
t1047 = ct{17};
t1048 = ct{18};
t1049 = ct{19};
t1055 = ct{20};
t106 = ct{21};
t1066 = ct{22};
t1068 = ct{23};
t1069 = ct{24};
t107 = ct{25};
t1070 = ct{26};
t1071 = ct{27};
t1079 = ct{28};
t108 = ct{29};
t1080 = ct{30};
t1081 = ct{31};
t1082 = ct{32};
t1083 = ct{33};
t1084 = ct{34};
t1085 = ct{35};
t1086 = ct{36};
t1087 = ct{37};
t1093 = ct{38};
t1094 = ct{39};
t1096 = ct{40};
t1097 = ct{41};
t1098 = ct{42};
t1106 = ct{43};
t1108 = ct{44};
t1109 = ct{45};
t111 = ct{46};
t1110 = ct{47};
t112 = ct{48};
t1121 = ct{49};
t1122 = ct{50};
t1123 = ct{51};
t1126 = ct{52};
t1128 = ct{53};
t1129 = ct{54};
t113 = ct{55};
t1133 = ct{56};
t1134 = ct{57};
t1135 = ct{58};
t1137 = ct{59};
t1138 = ct{60};
t1139 = ct{61};
t1140 = ct{62};
t1147 = ct{63};
t1148 = ct{64};
t1155 = ct{65};
t1156 = ct{66};
t1160 = ct{67};
t1162 = ct{68};
t1172 = ct{69};
t1174 = ct{70};
t1183 = ct{71};
t1184 = ct{72};
t1185 = ct{73};
t1186 = ct{74};
t1187 = ct{75};
t1189 = ct{76};
t1193 = ct{77};
t1196 = ct{78};
t12 = ct{79};
t1203 = ct{80};
t1208 = ct{81};
t1209 = ct{82};
t1210 = ct{83};
t1211 = ct{84};
t1222 = ct{85};
t1224 = ct{86};
t1225 = ct{87};
t1226 = ct{88};
t1227 = ct{89};
t1230 = ct{90};
t1236 = ct{91};
t1237 = ct{92};
t1238 = ct{93};
t124 = ct{94};
t1245 = ct{95};
t1246 = ct{96};
t1247 = ct{97};
t1248 = ct{98};
t1264 = ct{99};
t1265 = ct{100};
t1266 = ct{101};
t1268 = ct{102};
t127 = ct{103};
t1271 = ct{104};
t1272 = ct{105};
t1273 = ct{106};
t128 = ct{107};
t1281 = ct{108};
t1284 = ct{109};
t1287 = ct{110};
t1288 = ct{111};
t1289 = ct{112};
t1297 = ct{113};
t1298 = ct{114};
t13 = ct{115};
t1302 = ct{116};
t131 = ct{117};
t1311 = ct{118};
t1312 = ct{119};
t1316 = ct{120};
t1317 = ct{121};
t132 = ct{122};
t1321 = ct{123};
t1328 = ct{124};
t1331 = ct{125};
t1332 = ct{126};
t1333 = ct{127};
t1334 = ct{128};
t1335 = ct{129};
t134 = ct{130};
t1355 = ct{131};
t1356 = ct{132};
t1357 = ct{133};
t1358 = ct{134};
t136 = ct{135};
t1368 = ct{136};
t137 = ct{137};
t1375 = ct{138};
t1378 = ct{139};
t138 = ct{140};
t1399 = ct{141};
t14 = ct{142};
t1400 = ct{143};
t1403 = ct{144};
t1408 = ct{145};
t1410 = ct{146};
t1413 = ct{147};
t1419 = ct{148};
t1420 = ct{149};
t1427 = ct{150};
t1434 = ct{151};
t1440 = ct{152};
t1461 = ct{153};
t1464 = ct{154};
t1465 = ct{155};
t1468 = ct{156};
t1470 = ct{157};
t1472 = ct{158};
t1475 = ct{159};
t1479 = ct{160};
t1485 = ct{161};
t1492 = ct{162};
t1497 = ct{163};
t1499 = ct{164};
t15 = ct{165};
t150 = ct{166};
t1500 = ct{167};
t1501 = ct{168};
t1503 = ct{169};
t1504 = ct{170};
t1516 = ct{171};
t1517 = ct{172};
t1518 = ct{173};
t1519 = ct{174};
t152 = ct{175};
t1520 = ct{176};
t1521 = ct{177};
t1525 = ct{178};
t1526 = ct{179};
t1528 = ct{180};
t1529 = ct{181};
t1532 = ct{182};
t1534 = ct{183};
t1535 = ct{184};
t1536 = ct{185};
t1537 = ct{186};
t1547 = ct{187};
t155 = ct{188};
t156 = ct{189};
t1569 = ct{190};
t1571 = ct{191};
t1574 = ct{192};
t1578 = ct{193};
t1579 = ct{194};
t158 = ct{195};
t1580 = ct{196};
t1585 = ct{197};
t1586 = ct{198};
t1588 = ct{199};
t1589 = ct{200};
t159 = ct{201};
t1590 = ct{202};
t1597 = ct{203};
t1599 = ct{204};
t1606 = ct{205};
t1607 = ct{206};
t1609 = ct{207};
t1610 = ct{208};
t1615 = ct{209};
t1617 = ct{210};
t1618 = ct{211};
t162 = ct{212};
t163 = ct{213};
t1636 = ct{214};
t164 = ct{215};
t1645 = ct{216};
t1647 = ct{217};
t1648 = ct{218};
t1649 = ct{219};
t165 = ct{220};
t1650 = ct{221};
t1651 = ct{222};
t1652 = ct{223};
t1653 = ct{224};
t1659 = ct{225};
t1663 = ct{226};
t1671 = ct{227};
t1674 = ct{228};
t1677 = ct{229};
t1678 = ct{230};
t1680 = ct{231};
t1683 = ct{232};
t1685 = ct{233};
t1686 = ct{234};
t1687 = ct{235};
t1692 = ct{236};
t1699 = ct{237};
t1701 = ct{238};
t1704 = ct{239};
t1706 = ct{240};
t1709 = ct{241};
t171 = ct{242};
t1710 = ct{243};
t1713 = ct{244};
t1714 = ct{245};
t1715 = ct{246};
t173 = ct{247};
t1733 = ct{248};
t1736 = ct{249};
t1738 = ct{250};
t174 = ct{251};
t1740 = ct{252};
t1741 = ct{253};
t1742 = ct{254};
t1743 = ct{255};
t175 = ct{256};
t1751 = ct{257};
t1754 = ct{258};
t1755 = ct{259};
t1758 = ct{260};
t1759 = ct{261};
t1760 = ct{262};
t177 = ct{263};
t1776 = ct{264};
t1780 = ct{265};
t1783 = ct{266};
t1784 = ct{267};
t1786 = ct{268};
t1790 = ct{269};
t1792 = ct{270};
t1797 = ct{271};
t1799 = ct{272};
t18 = ct{273};
t1800 = ct{274};
t1803 = ct{275};
t1807 = ct{276};
t1813 = ct{277};
t1815 = ct{278};
t1816 = ct{279};
t1818 = ct{280};
t1827 = ct{281};
t1829 = ct{282};
t1832 = ct{283};
t1835 = ct{284};
t1837 = ct{285};
t1838 = ct{286};
t1840 = ct{287};
t1844 = ct{288};
t1848 = ct{289};
t1849 = ct{290};
t1862 = ct{291};
t1864 = ct{292};
t1866 = ct{293};
t1867 = ct{294};
t187 = ct{295};
t1872 = ct{296};
t1873 = ct{297};
t1874 = ct{298};
t1875 = ct{299};
t1885 = ct{300};
t1888 = ct{301};
t1889 = ct{302};
t1890 = ct{303};
t1891 = ct{304};
t1892 = ct{305};
t19 = ct{306};
t1903 = ct{307};
t1905 = ct{308};
t191 = ct{309};
t1916 = ct{310};
t1919 = ct{311};
t1920 = ct{312};
t1921 = ct{313};
t1925 = ct{314};
t1929 = ct{315};
t1930 = ct{316};
t1933 = ct{317};
t1935 = ct{318};
t1938 = ct{319};
t1939 = ct{320};
t1940 = ct{321};
t1944 = ct{322};
t1945 = ct{323};
t1956 = ct{324};
t1957 = ct{325};
t1958 = ct{326};
t1960 = ct{327};
t1961 = ct{328};
t1962 = ct{329};
t1963 = ct{330};
t1964 = ct{331};
t1965 = ct{332};
t1966 = ct{333};
t1967 = ct{334};
t1968 = ct{335};
t1969 = ct{336};
t1970 = ct{337};
t1971 = ct{338};
t1973 = ct{339};
t1976 = ct{340};
t1977 = ct{341};
t1983 = ct{342};
t1984 = ct{343};
t1988 = ct{344};
t199 = ct{345};
t1992 = ct{346};
t1993 = ct{347};
t1995 = ct{348};
t1996 = ct{349};
t1999 = ct{350};
t1d = ct{351};
t1dd = ct{352};
t200 = ct{353};
t2001 = ct{354};
t2005 = ct{355};
t2009 = ct{356};
t2012 = ct{357};
t2013 = ct{358};
t2018 = ct{359};
t2021 = ct{360};
t2022 = ct{361};
t2026 = ct{362};
t2028 = ct{363};
t2031 = ct{364};
t2033 = ct{365};
t2044 = ct{366};
t2053 = ct{367};
t2054 = ct{368};
t2059 = ct{369};
t206 = ct{370};
t2060 = ct{371};
t2061 = ct{372};
t2062 = ct{373};
t2068 = ct{374};
t2070 = ct{375};
t2074 = ct{376};
t2075 = ct{377};
t2079 = ct{378};
t2080 = ct{379};
t2081 = ct{380};
t2085 = ct{381};
t2086 = ct{382};
t2087 = ct{383};
t2088 = ct{384};
t2090 = ct{385};
t2093 = ct{386};
t2098 = ct{387};
t2099 = ct{388};
t21 = ct{389};
t2100 = ct{390};
t2101 = ct{391};
t2104 = ct{392};
t2112 = ct{393};
t2113 = ct{394};
t2115 = ct{395};
t2117 = ct{396};
t2119 = ct{397};
t2122 = ct{398};
t2123 = ct{399};
t2124 = ct{400};
t2126 = ct{401};
t2128 = ct{402};
t2129 = ct{403};
t2130 = ct{404};
t2136 = ct{405};
t2140 = ct{406};
t2141 = ct{407};
t2142 = ct{408};
t2143 = ct{409};
t2144 = ct{410};
t2145 = ct{411};
t2147 = ct{412};
t215 = ct{413};
t2155 = ct{414};
t2156 = ct{415};
t2167 = ct{416};
t2168 = ct{417};
t2169 = ct{418};
t2170 = ct{419};
t2171 = ct{420};
t2173 = ct{421};
t2174 = ct{422};
t2178 = ct{423};
t2180 = ct{424};
t2184 = ct{425};
t2186 = ct{426};
t2187 = ct{427};
t2188 = ct{428};
t2189 = ct{429};
t219 = ct{430};
t2190 = ct{431};
t2193 = ct{432};
t2198 = ct{433};
t22 = ct{434};
t220 = ct{435};
t2203 = ct{436};
t2204 = ct{437};
t2205 = ct{438};
t2206 = ct{439};
t2210 = ct{440};
t2213 = ct{441};
t2214 = ct{442};
t2215 = ct{443};
t2222 = ct{444};
t2223 = ct{445};
t2224 = ct{446};
t2225 = ct{447};
t2233 = ct{448};
t2235 = ct{449};
t2236 = ct{450};
t2237 = ct{451};
t2238 = ct{452};
t2239 = ct{453};
t2243 = ct{454};
t2246 = ct{455};
t2247 = ct{456};
t2249 = ct{457};
t2259 = ct{458};
t226 = ct{459};
t2266 = ct{460};
t2270 = ct{461};
t2279 = ct{462};
t2281 = ct{463};
t2285 = ct{464};
t2286 = ct{465};
t2289 = ct{466};
t229 = ct{467};
t2290 = ct{468};
t2292 = ct{469};
t2293 = ct{470};
t2294 = ct{471};
t2295 = ct{472};
t2296 = ct{473};
t23 = ct{474};
t2300 = ct{475};
t2304 = ct{476};
t2305 = ct{477};
t2306 = ct{478};
t2308 = ct{479};
t2310 = ct{480};
t2311 = ct{481};
t2317 = ct{482};
t232 = ct{483};
t2322 = ct{484};
t2327 = ct{485};
t233 = ct{486};
t2330 = ct{487};
t2331 = ct{488};
t2332 = ct{489};
t2339 = ct{490};
t2340 = ct{491};
t2344 = ct{492};
t2346 = ct{493};
t2348 = ct{494};
t2349 = ct{495};
t2350 = ct{496};
t2351 = ct{497};
t2352 = ct{498};
t2353 = ct{499};
t2354 = ct{500};
t2355 = ct{501};
t2356 = ct{502};
t2357 = ct{503};
t2358 = ct{504};
t2359 = ct{505};
t2360 = ct{506};
t2361 = ct{507};
t2362 = ct{508};
t2363 = ct{509};
t2364 = ct{510};
t2368 = ct{511};
t2369 = ct{512};
t2371 = ct{513};
t2372 = ct{514};
t2373 = ct{515};
t2374 = ct{516};
t2375 = ct{517};
t2376 = ct{518};
t2378 = ct{519};
t2379 = ct{520};
t2380 = ct{521};
t2382 = ct{522};
t2384 = ct{523};
t2386 = ct{524};
t2387 = ct{525};
t2393 = ct{526};
t2395 = ct{527};
t2398 = ct{528};
t2399 = ct{529};
t24 = ct{530};
t2400 = ct{531};
t2401 = ct{532};
t2402 = ct{533};
t2405 = ct{534};
t2406 = ct{535};
t2407 = ct{536};
t2409 = ct{537};
t2412 = ct{538};
t2414 = ct{539};
t2416 = ct{540};
t2421 = ct{541};
t2427 = ct{542};
t2428 = ct{543};
t2430 = ct{544};
t2431 = ct{545};
t2433 = ct{546};
t2434 = ct{547};
t2438 = ct{548};
t244 = ct{549};
t2460 = ct{550};
t2463 = ct{551};
t2466 = ct{552};
t2467 = ct{553};
t2468 = ct{554};
t247 = ct{555};
t2471 = ct{556};
t2472 = ct{557};
t2473 = ct{558};
t2475 = ct{559};
t2476 = ct{560};
t2477 = ct{561};
t2478 = ct{562};
t2479 = ct{563};
t2486 = ct{564};
t2488 = ct{565};
t2490 = ct{566};
t2492 = ct{567};
t2497 = ct{568};
t2499 = ct{569};
t25 = ct{570};
t2500 = ct{571};
t2501 = ct{572};
t2502 = ct{573};
t2503 = ct{574};
t2504 = ct{575};
t2506 = ct{576};
t2507 = ct{577};
t2508 = ct{578};
t2509 = ct{579};
t2510 = ct{580};
t2511 = ct{581};
t2512 = ct{582};
t2513 = ct{583};
t2514 = ct{584};
t2520 = ct{585};
t2523 = ct{586};
t2526 = ct{587};
t2527 = ct{588};
t2528 = ct{589};
t2532 = ct{590};
t2533 = ct{591};
t2534 = ct{592};
t2544 = ct{593};
t2549 = ct{594};
t255 = ct{595};
t2550 = ct{596};
t2557 = ct{597};
t256 = ct{598};
t2561 = ct{599};
t2562 = ct{600};
t2563 = ct{601};
t2564 = ct{602};
t2567 = ct{603};
t2568 = ct{604};
t2570 = ct{605};
t2574 = ct{606};
t2576 = ct{607};
t2578 = ct{608};
t2583 = ct{609};
t2585 = ct{610};
t2586 = ct{611};
t2587 = ct{612};
t2588 = ct{613};
t2589 = ct{614};
t2593 = ct{615};
t2596 = ct{616};
t2597 = ct{617};
t26 = ct{618};
t2601 = ct{619};
t2602 = ct{620};
t2603 = ct{621};
t2606 = ct{622};
t2608 = ct{623};
t2610 = ct{624};
t2612 = ct{625};
t2614 = ct{626};
t2616 = ct{627};
t2617 = ct{628};
t2619 = ct{629};
t2625 = ct{630};
t2626 = ct{631};
t2627 = ct{632};
t2630 = ct{633};
t2637 = ct{634};
t2640 = ct{635};
t2641 = ct{636};
t2642 = ct{637};
t2643 = ct{638};
t2644 = ct{639};
t2645 = ct{640};
t2647 = ct{641};
t2648 = ct{642};
t2652 = ct{643};
t2654 = ct{644};
t2655 = ct{645};
t2658 = ct{646};
t2659 = ct{647};
t2661 = ct{648};
t2664 = ct{649};
t2665 = ct{650};
t2666 = ct{651};
t2668 = ct{652};
t2669 = ct{653};
t2673 = ct{654};
t2675 = ct{655};
t2679 = ct{656};
t2681 = ct{657};
t2682 = ct{658};
t2689 = ct{659};
t2690 = ct{660};
t2691 = ct{661};
t2696 = ct{662};
t2699 = ct{663};
t27 = ct{664};
t2703 = ct{665};
t2705 = ct{666};
t2707 = ct{667};
t2708 = ct{668};
t2709 = ct{669};
t2711 = ct{670};
t2718 = ct{671};
t2719 = ct{672};
t2721 = ct{673};
t2722 = ct{674};
t2724 = ct{675};
t2731 = ct{676};
t2734 = ct{677};
t2737 = ct{678};
t2743 = ct{679};
t2744 = ct{680};
t2745 = ct{681};
t2747 = ct{682};
t2749 = ct{683};
t2755 = ct{684};
t2758 = ct{685};
t2759 = ct{686};
t2772 = ct{687};
t2775 = ct{688};
t2776 = ct{689};
t2777 = ct{690};
t2779 = ct{691};
t2780 = ct{692};
t2781 = ct{693};
t2782 = ct{694};
t2786 = ct{695};
t2787 = ct{696};
t2788 = ct{697};
t2790 = ct{698};
t2795 = ct{699};
t2796 = ct{700};
t2797 = ct{701};
t2798 = ct{702};
t2805 = ct{703};
t2807 = ct{704};
t2808 = ct{705};
t2809 = ct{706};
t2810 = ct{707};
t2813 = ct{708};
t2814 = ct{709};
t2815 = ct{710};
t2816 = ct{711};
t2828 = ct{712};
t2829 = ct{713};
t2830 = ct{714};
t2835 = ct{715};
t2841 = ct{716};
t2842 = ct{717};
t2843 = ct{718};
t2845 = ct{719};
t2847 = ct{720};
t2848 = ct{721};
t2853 = ct{722};
t2857 = ct{723};
t2862 = ct{724};
t2864 = ct{725};
t2865 = ct{726};
t2867 = ct{727};
t2868 = ct{728};
t2870 = ct{729};
t2873 = ct{730};
t2874 = ct{731};
t2876 = ct{732};
t2878 = ct{733};
t2882 = ct{734};
t2883 = ct{735};
t2884 = ct{736};
t2885 = ct{737};
t2887 = ct{738};
t2890 = ct{739};
t2891 = ct{740};
t2895 = ct{741};
t2899 = ct{742};
t29 = ct{743};
t2900 = ct{744};
t2901 = ct{745};
t2902 = ct{746};
t2904 = ct{747};
t2906 = ct{748};
t2908 = ct{749};
t2909 = ct{750};
t2915 = ct{751};
t2925 = ct{752};
t2929 = ct{753};
t2931 = ct{754};
t2935 = ct{755};
t2936 = ct{756};
t2937 = ct{757};
t2940 = ct{758};
t2946 = ct{759};
t2947 = ct{760};
t2951 = ct{761};
t2953 = ct{762};
t2954 = ct{763};
t2956 = ct{764};
t2958 = ct{765};
t2959 = ct{766};
t2961 = ct{767};
t2962 = ct{768};
t2963 = ct{769};
t2966 = ct{770};
t2967 = ct{771};
t2968 = ct{772};
t2970 = ct{773};
t2971 = ct{774};
t2972 = ct{775};
t2973 = ct{776};
t2982 = ct{777};
t2983 = ct{778};
t2984 = ct{779};
t2985 = ct{780};
t2988 = ct{781};
t2989 = ct{782};
t299 = ct{783};
t2991 = ct{784};
t2992 = ct{785};
t2993 = ct{786};
t2994 = ct{787};
t2995 = ct{788};
t2996 = ct{789};
t2997 = ct{790};
t2998 = ct{791};
t2999 = ct{792};
t2d = ct{793};
t2dd = ct{794};
t30 = ct{795};
t3000 = ct{796};
t3003 = ct{797};
t3004 = ct{798};
t3007 = ct{799};
t3009 = ct{800};
t301 = ct{801};
t3010 = ct{802};
t3011 = ct{803};
t3012 = ct{804};
t3013 = ct{805};
t3014 = ct{806};
t3017 = ct{807};
t3018 = ct{808};
t3029 = ct{809};
t3035 = ct{810};
t3052 = ct{811};
t3057 = ct{812};
t3058 = ct{813};
t3059 = ct{814};
t3065 = ct{815};
t3066 = ct{816};
t3069 = ct{817};
t3073 = ct{818};
t3076 = ct{819};
t3078 = ct{820};
t3079 = ct{821};
t308 = ct{822};
t3080 = ct{823};
t3081 = ct{824};
t3082 = ct{825};
t3083 = ct{826};
t3084 = ct{827};
t3085 = ct{828};
t3086 = ct{829};
t3087 = ct{830};
t3088 = ct{831};
t3090 = ct{832};
t3094 = ct{833};
t3098 = ct{834};
t3099 = ct{835};
t31 = ct{836};
t3100 = ct{837};
t3101 = ct{838};
t3104 = ct{839};
t3106 = ct{840};
t3107 = ct{841};
t3108 = ct{842};
t3109 = ct{843};
t3112 = ct{844};
t3115 = ct{845};
t3120 = ct{846};
t3123 = ct{847};
t3124 = ct{848};
t3125 = ct{849};
t3126 = ct{850};
t3129 = ct{851};
t3130 = ct{852};
t3133 = ct{853};
t3135 = ct{854};
t3136 = ct{855};
t3137 = ct{856};
t3138 = ct{857};
t3139 = ct{858};
t3140 = ct{859};
t3143 = ct{860};
t3144 = ct{861};
t3146 = ct{862};
t315 = ct{863};
t3151 = ct{864};
t3155 = ct{865};
t3156 = ct{866};
t3159 = ct{867};
t3161 = ct{868};
t3162 = ct{869};
t3163 = ct{870};
t3164 = ct{871};
t3165 = ct{872};
t3166 = ct{873};
t3167 = ct{874};
t317 = ct{875};
t3170 = ct{876};
t3171 = ct{877};
t3172 = ct{878};
t3173 = ct{879};
t3174 = ct{880};
t3175 = ct{881};
t3176 = ct{882};
t3177 = ct{883};
t318 = ct{884};
t3180 = ct{885};
t3181 = ct{886};
t3182 = ct{887};
t3183 = ct{888};
t3184 = ct{889};
t3185 = ct{890};
t3186 = ct{891};
t3187 = ct{892};
t3188 = ct{893};
t319 = ct{894};
t3192 = ct{895};
t3195 = ct{896};
t3196 = ct{897};
t3197 = ct{898};
t3199 = ct{899};
t3201 = ct{900};
t3202 = ct{901};
t3203 = ct{902};
t3204 = ct{903};
t3205 = ct{904};
t3209 = ct{905};
t3210 = ct{906};
t3211 = ct{907};
t3212 = ct{908};
t3214 = ct{909};
t3215 = ct{910};
t3216 = ct{911};
t3217 = ct{912};
t3218 = ct{913};
t3219 = ct{914};
t3220 = ct{915};
t3221 = ct{916};
t3225 = ct{917};
t3227 = ct{918};
t3228 = ct{919};
t3229 = ct{920};
t3230 = ct{921};
t3231 = ct{922};
t3232 = ct{923};
t3233 = ct{924};
t3234 = ct{925};
t3236 = ct{926};
t3237 = ct{927};
t3239 = ct{928};
t3240 = ct{929};
t3241 = ct{930};
t3243 = ct{931};
t3244 = ct{932};
t3246 = ct{933};
t3248 = ct{934};
t325 = ct{935};
t3251 = ct{936};
t3254 = ct{937};
t3255 = ct{938};
t3257 = ct{939};
t3258 = ct{940};
t3260 = ct{941};
t3264 = ct{942};
t3265 = ct{943};
t3266 = ct{944};
t3267 = ct{945};
t3268 = ct{946};
t3269 = ct{947};
t3270 = ct{948};
t3271 = ct{949};
t3272 = ct{950};
t3273 = ct{951};
t3274 = ct{952};
t3276 = ct{953};
t3277 = ct{954};
t3279 = ct{955};
t3280 = ct{956};
t3281 = ct{957};
t3282 = ct{958};
t3283 = ct{959};
t3284 = ct{960};
t3285 = ct{961};
t3287 = ct{962};
t3288 = ct{963};
t3289 = ct{964};
t329 = ct{965};
t3291 = ct{966};
t3292 = ct{967};
t3293 = ct{968};
t3294 = ct{969};
t3297 = ct{970};
t3298 = ct{971};
t330 = ct{972};
t3300 = ct{973};
t3301 = ct{974};
t3304 = ct{975};
t3306 = ct{976};
t3308 = ct{977};
t3309 = ct{978};
t3310 = ct{979};
t3311 = ct{980};
t3312 = ct{981};
t3314 = ct{982};
t3316 = ct{983};
t3318 = ct{984};
t3320 = ct{985};
t3321 = ct{986};
t3322 = ct{987};
t3324 = ct{988};
t3326 = ct{989};
t3327 = ct{990};
t3329 = ct{991};
t333 = ct{992};
t3330 = ct{993};
t3331 = ct{994};
t3332 = ct{995};
t3334 = ct{996};
t3335 = ct{997};
t3338 = ct{998};
t3339 = ct{999};
t3340 = ct{1000};
t3344 = ct{1001};
t3348 = ct{1002};
t3349 = ct{1003};
t3350 = ct{1004};
t3351 = ct{1005};
t3354 = ct{1006};
t3355 = ct{1007};
t3358 = ct{1008};
t3359 = ct{1009};
t3360 = ct{1010};
t3362 = ct{1011};
t3364 = ct{1012};
t3365 = ct{1013};
t3369 = ct{1014};
t3370 = ct{1015};
t3372 = ct{1016};
t3373 = ct{1017};
t3374 = ct{1018};
t3376 = ct{1019};
t3377 = ct{1020};
t3378 = ct{1021};
t3379 = ct{1022};
t3380 = ct{1023};
t3381 = ct{1024};
t3382 = ct{1025};
t3383 = ct{1026};
t3384 = ct{1027};
t3385 = ct{1028};
t3386 = ct{1029};
t3387 = ct{1030};
t3388 = ct{1031};
t3389 = ct{1032};
t3390 = ct{1033};
t3391 = ct{1034};
t3392 = ct{1035};
t3394 = ct{1036};
t3395 = ct{1037};
t3397 = ct{1038};
t3398 = ct{1039};
t3399 = ct{1040};
t34 = ct{1041};
t3400 = ct{1042};
t3401 = ct{1043};
t3402 = ct{1044};
t3404 = ct{1045};
t3405 = ct{1046};
t3406 = ct{1047};
t341 = ct{1048};
t3410 = ct{1049};
t3412 = ct{1050};
t3414 = ct{1051};
t3415 = ct{1052};
t3416 = ct{1053};
t3417 = ct{1054};
t3419 = ct{1055};
t342 = ct{1056};
t3421 = ct{1057};
t3426 = ct{1058};
t3427 = ct{1059};
t3429 = ct{1060};
t343 = ct{1061};
t3430 = ct{1062};
t3431 = ct{1063};
t3432 = ct{1064};
t3439 = ct{1065};
t3440 = ct{1066};
t3442 = ct{1067};
t3445 = ct{1068};
t3452 = ct{1069};
t3456 = ct{1070};
t3457 = ct{1071};
t3458 = ct{1072};
t3459 = ct{1073};
t346 = ct{1074};
t3460 = ct{1075};
t3461 = ct{1076};
t3462 = ct{1077};
t3468 = ct{1078};
t3469 = ct{1079};
t347 = ct{1080};
t3472 = ct{1081};
t3473 = ct{1082};
t3474 = ct{1083};
t3475 = ct{1084};
t3477 = ct{1085};
t3478 = ct{1086};
t3483 = ct{1087};
t3486 = ct{1088};
t3491 = ct{1089};
t3492 = ct{1090};
t3497 = ct{1091};
t3499 = ct{1092};
t3501 = ct{1093};
t3502 = ct{1094};
t3503 = ct{1095};
t3506 = ct{1096};
t3507 = ct{1097};
t3509 = ct{1098};
t3510 = ct{1099};
t3512 = ct{1100};
t3514 = ct{1101};
t3515 = ct{1102};
t3516 = ct{1103};
t3517 = ct{1104};
t3518 = ct{1105};
t3519 = ct{1106};
t3521 = ct{1107};
t3524 = ct{1108};
t3525 = ct{1109};
t3526 = ct{1110};
t3532 = ct{1111};
t3533 = ct{1112};
t3535 = ct{1113};
t3536 = ct{1114};
t3537 = ct{1115};
t3538 = ct{1116};
t3539 = ct{1117};
t3541 = ct{1118};
t3542 = ct{1119};
t3543 = ct{1120};
t3544 = ct{1121};
t3547 = ct{1122};
t3548 = ct{1123};
t3549 = ct{1124};
t3552 = ct{1125};
t3557 = ct{1126};
t3558 = ct{1127};
t3559 = ct{1128};
t3561 = ct{1129};
t3566 = ct{1130};
t3570 = ct{1131};
t3571 = ct{1132};
t3574 = ct{1133};
t3575 = ct{1134};
t3576 = ct{1135};
t3578 = ct{1136};
t3579 = ct{1137};
t3580 = ct{1138};
t3582 = ct{1139};
t3583 = ct{1140};
t3586 = ct{1141};
t3587 = ct{1142};
t3588 = ct{1143};
t3590 = ct{1144};
t3591 = ct{1145};
t3592 = ct{1146};
t3594 = ct{1147};
t3595 = ct{1148};
t3597 = ct{1149};
t3598 = ct{1150};
t3599 = ct{1151};
t36 = ct{1152};
t3601 = ct{1153};
t3602 = ct{1154};
t3603 = ct{1155};
t3604 = ct{1156};
t3605 = ct{1157};
t3607 = ct{1158};
t3608 = ct{1159};
t3609 = ct{1160};
t3610 = ct{1161};
t3611 = ct{1162};
t3613 = ct{1163};
t3617 = ct{1164};
t3618 = ct{1165};
t3620 = ct{1166};
t3622 = ct{1167};
t3623 = ct{1168};
t3624 = ct{1169};
t3625 = ct{1170};
t3628 = ct{1171};
t3630 = ct{1172};
t3631 = ct{1173};
t3632 = ct{1174};
t3633 = ct{1175};
t3634 = ct{1176};
t3635 = ct{1177};
t3636 = ct{1178};
t3637 = ct{1179};
t3638 = ct{1180};
t3639 = ct{1181};
t364 = ct{1182};
t3640 = ct{1183};
t3643 = ct{1184};
t3645 = ct{1185};
t3646 = ct{1186};
t3647 = ct{1187};
t3648 = ct{1188};
t365 = ct{1189};
t3650 = ct{1190};
t3652 = ct{1191};
t3653 = ct{1192};
t3654 = ct{1193};
t3655 = ct{1194};
t3656 = ct{1195};
t3657 = ct{1196};
t3658 = ct{1197};
t3659 = ct{1198};
t3660 = ct{1199};
t3662 = ct{1200};
t3663 = ct{1201};
t3664 = ct{1202};
t3665 = ct{1203};
t3667 = ct{1204};
t3668 = ct{1205};
t3669 = ct{1206};
t3670 = ct{1207};
t3671 = ct{1208};
t3672 = ct{1209};
t3673 = ct{1210};
t368 = ct{1211};
t3680 = ct{1212};
t3682 = ct{1213};
t3683 = ct{1214};
t3684 = ct{1215};
t3685 = ct{1216};
t3686 = ct{1217};
t3687 = ct{1218};
t3689 = ct{1219};
t3691 = ct{1220};
t3692 = ct{1221};
t3693 = ct{1222};
t3694 = ct{1223};
t3695 = ct{1224};
t3696 = ct{1225};
t3698 = ct{1226};
t37 = ct{1227};
t3700 = ct{1228};
t3701 = ct{1229};
t3702 = ct{1230};
t3703 = ct{1231};
t3705 = ct{1232};
t3706 = ct{1233};
t3707 = ct{1234};
t3708 = ct{1235};
t3710 = ct{1236};
t3711 = ct{1237};
t3712 = ct{1238};
t3713 = ct{1239};
t3715 = ct{1240};
t3716 = ct{1241};
t3717 = ct{1242};
t3718 = ct{1243};
t3719 = ct{1244};
t3723 = ct{1245};
t3732 = ct{1246};
t3734 = ct{1247};
t3735 = ct{1248};
t3739 = ct{1249};
t3741 = ct{1250};
t3742 = ct{1251};
t3745 = ct{1252};
t3747 = ct{1253};
t3750 = ct{1254};
t3751 = ct{1255};
t3754 = ct{1256};
t3755 = ct{1257};
t3756 = ct{1258};
t3757 = ct{1259};
t3759 = ct{1260};
t3762 = ct{1261};
t3770 = ct{1262};
t3771 = ct{1263};
t3772 = ct{1264};
t3773 = ct{1265};
t3780 = ct{1266};
t3781 = ct{1267};
t3782 = ct{1268};
t3785 = ct{1269};
t3787 = ct{1270};
t3788 = ct{1271};
t3789 = ct{1272};
t3790 = ct{1273};
t3793 = ct{1274};
t3795 = ct{1275};
t3797 = ct{1276};
t3798 = ct{1277};
t38 = ct{1278};
t3800 = ct{1279};
t3801 = ct{1280};
t3804 = ct{1281};
t3805 = ct{1282};
t3807 = ct{1283};
t3808 = ct{1284};
t3809 = ct{1285};
t3812 = ct{1286};
t3816 = ct{1287};
t3817 = ct{1288};
t3818 = ct{1289};
t3819 = ct{1290};
t3821 = ct{1291};
t3822 = ct{1292};
t3823 = ct{1293};
t3824 = ct{1294};
t3825 = ct{1295};
t3826 = ct{1296};
t3832 = ct{1297};
t3833 = ct{1298};
t3834 = ct{1299};
t3836 = ct{1300};
t3838 = ct{1301};
t3839 = ct{1302};
t3840 = ct{1303};
t3843 = ct{1304};
t3844 = ct{1305};
t3847 = ct{1306};
t3848 = ct{1307};
t3856 = ct{1308};
t3858 = ct{1309};
t3859 = ct{1310};
t3861 = ct{1311};
t3862 = ct{1312};
t3863 = ct{1313};
t3865 = ct{1314};
t3866 = ct{1315};
t3867 = ct{1316};
t3870 = ct{1317};
t3872 = ct{1318};
t3873 = ct{1319};
t3874 = ct{1320};
t3875 = ct{1321};
t3880 = ct{1322};
t3881 = ct{1323};
t3882 = ct{1324};
t3883 = ct{1325};
t3885 = ct{1326};
t3886 = ct{1327};
t3887 = ct{1328};
t3888 = ct{1329};
t3889 = ct{1330};
t3890 = ct{1331};
t3892 = ct{1332};
t3894 = ct{1333};
t3898 = ct{1334};
t3899 = ct{1335};
t39 = ct{1336};
t3900 = ct{1337};
t3901 = ct{1338};
t3903 = ct{1339};
t3904 = ct{1340};
t3909 = ct{1341};
t3911 = ct{1342};
t3912 = ct{1343};
t3913 = ct{1344};
t3915 = ct{1345};
t3916 = ct{1346};
t3917 = ct{1347};
t3919 = ct{1348};
t392 = ct{1349};
t3923 = ct{1350};
t3924 = ct{1351};
t3925 = ct{1352};
t3927 = ct{1353};
t3928 = ct{1354};
t393 = ct{1355};
t3930 = ct{1356};
t3931 = ct{1357};
t3932 = ct{1358};
t3933 = ct{1359};
t3935 = ct{1360};
t3936 = ct{1361};
t3937 = ct{1362};
t3942 = ct{1363};
t3943 = ct{1364};
t3944 = ct{1365};
t3945 = ct{1366};
t3951 = ct{1367};
t3953 = ct{1368};
t3955 = ct{1369};
t3956 = ct{1370};
t3958 = ct{1371};
t3960 = ct{1372};
t3961 = ct{1373};
t3962 = ct{1374};
t3964 = ct{1375};
t3965 = ct{1376};
t3966 = ct{1377};
t3967 = ct{1378};
t3969 = ct{1379};
t3971 = ct{1380};
t3972 = ct{1381};
t3975 = ct{1382};
t3976 = ct{1383};
t3977 = ct{1384};
t3978 = ct{1385};
t3979 = ct{1386};
t3981 = ct{1387};
t3982 = ct{1388};
t3984 = ct{1389};
t3985 = ct{1390};
t3989 = ct{1391};
t3990 = ct{1392};
t3991 = ct{1393};
t3992 = ct{1394};
t3994 = ct{1395};
t3995 = ct{1396};
t3996 = ct{1397};
t3997 = ct{1398};
t3998 = ct{1399};
t3999 = ct{1400};
t3d = ct{1401};
t3dd = ct{1402};
t4000 = ct{1403};
t4001 = ct{1404};
t4002 = ct{1405};
t4003 = ct{1406};
t4005 = ct{1407};
t4006 = ct{1408};
t4007 = ct{1409};
t4009 = ct{1410};
t401 = ct{1411};
t4010 = ct{1412};
t4011 = ct{1413};
t4012 = ct{1414};
t4013 = ct{1415};
t4015 = ct{1416};
t4016 = ct{1417};
t4017 = ct{1418};
t402 = ct{1419};
t4022 = ct{1420};
t4023 = ct{1421};
t4025 = ct{1422};
t4026 = ct{1423};
t4027 = ct{1424};
t403 = ct{1425};
t4031 = ct{1426};
t4032 = ct{1427};
t4033 = ct{1428};
t4036 = ct{1429};
t4037 = ct{1430};
t4038 = ct{1431};
t4039 = ct{1432};
t404 = ct{1433};
t4041 = ct{1434};
t4042 = ct{1435};
t4043 = ct{1436};
t4046 = ct{1437};
t4047 = ct{1438};
t4048 = ct{1439};
t4049 = ct{1440};
t4050 = ct{1441};
t4051 = ct{1442};
t4053 = ct{1443};
t4059 = ct{1444};
t4060 = ct{1445};
t4062 = ct{1446};
t4065 = ct{1447};
t4068 = ct{1448};
t4069 = ct{1449};
t4071 = ct{1450};
t4074 = ct{1451};
t4078 = ct{1452};
t4079 = ct{1453};
t4084 = ct{1454};
t4087 = ct{1455};
t4093 = ct{1456};
t4094 = ct{1457};
t4095 = ct{1458};
t4096 = ct{1459};
t41 = ct{1460};
t4100 = ct{1461};
t4101 = ct{1462};
t4102 = ct{1463};
t4104 = ct{1464};
t4105 = ct{1465};
t4106 = ct{1466};
t4108 = ct{1467};
t4110 = ct{1468};
t4111 = ct{1469};
t4115 = ct{1470};
t4117 = ct{1471};
t4118 = ct{1472};
t4121 = ct{1473};
t4122 = ct{1474};
t4125 = ct{1475};
t4127 = ct{1476};
t4128 = ct{1477};
t4130 = ct{1478};
t4131 = ct{1479};
t4133 = ct{1480};
t4136 = ct{1481};
t4137 = ct{1482};
t4139 = ct{1483};
t4143 = ct{1484};
t4146 = ct{1485};
t4147 = ct{1486};
t4149 = ct{1487};
t4151 = ct{1488};
t4152 = ct{1489};
t4154 = ct{1490};
t4155 = ct{1491};
t4156 = ct{1492};
t4157 = ct{1493};
t4159 = ct{1494};
t4161 = ct{1495};
t4163 = ct{1496};
t4164 = ct{1497};
t4166 = ct{1498};
t4167 = ct{1499};
t4168 = ct{1500};
t4170 = ct{1501};
t4171 = ct{1502};
t4172 = ct{1503};
t4174 = ct{1504};
t4176 = ct{1505};
t4178 = ct{1506};
t418 = ct{1507};
t4181 = ct{1508};
t4182 = ct{1509};
t4183 = ct{1510};
t4184 = ct{1511};
t4185 = ct{1512};
t4186 = ct{1513};
t4187 = ct{1514};
t4188 = ct{1515};
t4189 = ct{1516};
t419 = ct{1517};
t4190 = ct{1518};
t4191 = ct{1519};
t4192 = ct{1520};
t4193 = ct{1521};
t4195 = ct{1522};
t4196 = ct{1523};
t42 = ct{1524};
t420 = ct{1525};
t4200 = ct{1526};
t4201 = ct{1527};
t4203 = ct{1528};
t4204 = ct{1529};
t4205 = ct{1530};
t4209 = ct{1531};
t4210 = ct{1532};
t4211 = ct{1533};
t4212 = ct{1534};
t4214 = ct{1535};
t4221 = ct{1536};
t4223 = ct{1537};
t4224 = ct{1538};
t4226 = ct{1539};
t4227 = ct{1540};
t4228 = ct{1541};
t4229 = ct{1542};
t4230 = ct{1543};
t4231 = ct{1544};
t4232 = ct{1545};
t4233 = ct{1546};
t4234 = ct{1547};
t4235 = ct{1548};
t4236 = ct{1549};
t4237 = ct{1550};
t4238 = ct{1551};
t4239 = ct{1552};
t4240 = ct{1553};
t4241 = ct{1554};
t4243 = ct{1555};
t4244 = ct{1556};
t4247 = ct{1557};
t4249 = ct{1558};
t425 = ct{1559};
t4250 = ct{1560};
t4251 = ct{1561};
t4252 = ct{1562};
t4253 = ct{1563};
t4255 = ct{1564};
t4256 = ct{1565};
t4259 = ct{1566};
t4260 = ct{1567};
t4261 = ct{1568};
t4264 = ct{1569};
t4265 = ct{1570};
t4266 = ct{1571};
t4267 = ct{1572};
t4269 = ct{1573};
t4270 = ct{1574};
t4271 = ct{1575};
t4272 = ct{1576};
t4275 = ct{1577};
t4277 = ct{1578};
t4278 = ct{1579};
t4279 = ct{1580};
t4280 = ct{1581};
t4281 = ct{1582};
t4282 = ct{1583};
t4283 = ct{1584};
t4284 = ct{1585};
t4285 = ct{1586};
t4286 = ct{1587};
t4290 = ct{1588};
t4291 = ct{1589};
t4292 = ct{1590};
t4293 = ct{1591};
t4295 = ct{1592};
t4296 = ct{1593};
t4298 = ct{1594};
t4299 = ct{1595};
t4300 = ct{1596};
t4301 = ct{1597};
t4303 = ct{1598};
t4304 = ct{1599};
t4306 = ct{1600};
t4307 = ct{1601};
t4308 = ct{1602};
t4309 = ct{1603};
t431 = ct{1604};
t4311 = ct{1605};
t4315 = ct{1606};
t4316 = ct{1607};
t4317 = ct{1608};
t4318 = ct{1609};
t4319 = ct{1610};
t4320 = ct{1611};
t4321 = ct{1612};
t4323 = ct{1613};
t4324 = ct{1614};
t4325 = ct{1615};
t4327 = ct{1616};
t4328 = ct{1617};
t4330 = ct{1618};
t4331 = ct{1619};
t4332 = ct{1620};
t4335 = ct{1621};
t4337 = ct{1622};
t4338 = ct{1623};
t4339 = ct{1624};
t434 = ct{1625};
t4343 = ct{1626};
t4345 = ct{1627};
t4347 = ct{1628};
t4348 = ct{1629};
t4350 = ct{1630};
t4352 = ct{1631};
t4353 = ct{1632};
t4358 = ct{1633};
t4359 = ct{1634};
t4361 = ct{1635};
t4363 = ct{1636};
t4364 = ct{1637};
t4367 = ct{1638};
t4369 = ct{1639};
t437 = ct{1640};
t4370 = ct{1641};
t4371 = ct{1642};
t4373 = ct{1643};
t4374 = ct{1644};
t4375 = ct{1645};
t4376 = ct{1646};
t4377 = ct{1647};
t4378 = ct{1648};
t4387 = ct{1649};
t4390 = ct{1650};
t4391 = ct{1651};
t4392 = ct{1652};
t4394 = ct{1653};
t4395 = ct{1654};
t4399 = ct{1655};
t4400 = ct{1656};
t4401 = ct{1657};
t4402 = ct{1658};
t4404 = ct{1659};
t4406 = ct{1660};
t4408 = ct{1661};
t441 = ct{1662};
t4410 = ct{1663};
t4411 = ct{1664};
t4412 = ct{1665};
t4413 = ct{1666};
t4415 = ct{1667};
t4419 = ct{1668};
t442 = ct{1669};
t4420 = ct{1670};
t4421 = ct{1671};
t4422 = ct{1672};
t4423 = ct{1673};
t4424 = ct{1674};
t4427 = ct{1675};
t4428 = ct{1676};
t4429 = ct{1677};
t443 = ct{1678};
t4430 = ct{1679};
t4431 = ct{1680};
t4433 = ct{1681};
t4435 = ct{1682};
t4437 = ct{1683};
t4439 = ct{1684};
t4441 = ct{1685};
t4444 = ct{1686};
t4445 = ct{1687};
t4446 = ct{1688};
t4450 = ct{1689};
t4451 = ct{1690};
t4454 = ct{1691};
t4455 = ct{1692};
t4456 = ct{1693};
t4457 = ct{1694};
t4459 = ct{1695};
t446 = ct{1696};
t4460 = ct{1697};
t4461 = ct{1698};
t4462 = ct{1699};
t4463 = ct{1700};
t4464 = ct{1701};
t4465 = ct{1702};
t4467 = ct{1703};
t4468 = ct{1704};
t4470 = ct{1705};
t4473 = ct{1706};
t4474 = ct{1707};
t4475 = ct{1708};
t4476 = ct{1709};
t4479 = ct{1710};
t4480 = ct{1711};
t4481 = ct{1712};
t4483 = ct{1713};
t4484 = ct{1714};
t4485 = ct{1715};
t4487 = ct{1716};
t4488 = ct{1717};
t4490 = ct{1718};
t4491 = ct{1719};
t4492 = ct{1720};
t4493 = ct{1721};
t4494 = ct{1722};
t4498 = ct{1723};
t4500 = ct{1724};
t4503 = ct{1725};
t4505 = ct{1726};
t4506 = ct{1727};
t4508 = ct{1728};
t4509 = ct{1729};
t4511 = ct{1730};
t4515 = ct{1731};
t4516 = ct{1732};
t4519 = ct{1733};
t4520 = ct{1734};
t4521 = ct{1735};
t4522 = ct{1736};
t4526 = ct{1737};
t4527 = ct{1738};
t4528 = ct{1739};
t453 = ct{1740};
t4530 = ct{1741};
t4531 = ct{1742};
t4532 = ct{1743};
t4533 = ct{1744};
t4534 = ct{1745};
t4537 = ct{1746};
t4538 = ct{1747};
t4539 = ct{1748};
t454 = ct{1749};
t4540 = ct{1750};
t4541 = ct{1751};
t4542 = ct{1752};
t4543 = ct{1753};
t4545 = ct{1754};
t4546 = ct{1755};
t4547 = ct{1756};
t4548 = ct{1757};
t4550 = ct{1758};
t4551 = ct{1759};
t4552 = ct{1760};
t4553 = ct{1761};
t4556 = ct{1762};
t4559 = ct{1763};
t4561 = ct{1764};
t4564 = ct{1765};
t4567 = ct{1766};
t4568 = ct{1767};
t4569 = ct{1768};
t4571 = ct{1769};
t4572 = ct{1770};
t4575 = ct{1771};
t4576 = ct{1772};
t4577 = ct{1773};
t4578 = ct{1774};
t4579 = ct{1775};
t4582 = ct{1776};
t4583 = ct{1777};
t4586 = ct{1778};
t4587 = ct{1779};
t4588 = ct{1780};
t459 = ct{1781};
t4590 = ct{1782};
t4591 = ct{1783};
t4593 = ct{1784};
t4594 = ct{1785};
t4595 = ct{1786};
t4596 = ct{1787};
t4599 = ct{1788};
t4601 = ct{1789};
t4603 = ct{1790};
t4604 = ct{1791};
t4605 = ct{1792};
t4606 = ct{1793};
t4607 = ct{1794};
t4608 = ct{1795};
t4609 = ct{1796};
t4612 = ct{1797};
t4616 = ct{1798};
t4617 = ct{1799};
t4618 = ct{1800};
t4623 = ct{1801};
t4625 = ct{1802};
t4626 = ct{1803};
t4627 = ct{1804};
t4630 = ct{1805};
t4631 = ct{1806};
t4633 = ct{1807};
t4634 = ct{1808};
t4635 = ct{1809};
t4636 = ct{1810};
t4637 = ct{1811};
t4638 = ct{1812};
t4639 = ct{1813};
t4640 = ct{1814};
t4641 = ct{1815};
t4642 = ct{1816};
t4644 = ct{1817};
t4645 = ct{1818};
t4646 = ct{1819};
t4647 = ct{1820};
t4648 = ct{1821};
t4649 = ct{1822};
t4650 = ct{1823};
t4651 = ct{1824};
t4652 = ct{1825};
t4653 = ct{1826};
t4655 = ct{1827};
t4656 = ct{1828};
t4657 = ct{1829};
t4658 = ct{1830};
t4659 = ct{1831};
t4661 = ct{1832};
t4662 = ct{1833};
t4663 = ct{1834};
t4664 = ct{1835};
t4665 = ct{1836};
t4666 = ct{1837};
t4668 = ct{1838};
t4670 = ct{1839};
t4672 = ct{1840};
t4673 = ct{1841};
t4674 = ct{1842};
t4675 = ct{1843};
t4677 = ct{1844};
t4678 = ct{1845};
t4679 = ct{1846};
t4681 = ct{1847};
t4684 = ct{1848};
t4686 = ct{1849};
t4689 = ct{1850};
t4690 = ct{1851};
t4691 = ct{1852};
t4692 = ct{1853};
t4694 = ct{1854};
t4695 = ct{1855};
t4699 = ct{1856};
t470 = ct{1857};
t4700 = ct{1858};
t4701 = ct{1859};
t4703 = ct{1860};
t4704 = ct{1861};
t4705 = ct{1862};
t4707 = ct{1863};
t4708 = ct{1864};
t4709 = ct{1865};
t4711 = ct{1866};
t4712 = ct{1867};
t4713 = ct{1868};
t4714 = ct{1869};
t4715 = ct{1870};
t4716 = ct{1871};
t4717 = ct{1872};
t4720 = ct{1873};
t4721 = ct{1874};
t4722 = ct{1875};
t4723 = ct{1876};
t4724 = ct{1877};
t4725 = ct{1878};
t4726 = ct{1879};
t4727 = ct{1880};
t4730 = ct{1881};
t4731 = ct{1882};
t4733 = ct{1883};
t4734 = ct{1884};
t4735 = ct{1885};
t4736 = ct{1886};
t4737 = ct{1887};
t4738 = ct{1888};
t4739 = ct{1889};
t4740 = ct{1890};
t4741 = ct{1891};
t4744 = ct{1892};
t4745 = ct{1893};
t4747 = ct{1894};
t4748 = ct{1895};
t4752 = ct{1896};
t4754 = ct{1897};
t4757 = ct{1898};
t4758 = ct{1899};
t4759 = ct{1900};
t4760 = ct{1901};
t4761 = ct{1902};
t4762 = ct{1903};
t4765 = ct{1904};
t4766 = ct{1905};
t4767 = ct{1906};
t4768 = ct{1907};
t4769 = ct{1908};
t4770 = ct{1909};
t4771 = ct{1910};
t4772 = ct{1911};
t4774 = ct{1912};
t4776 = ct{1913};
t4778 = ct{1914};
t478 = ct{1915};
t4780 = ct{1916};
t4782 = ct{1917};
t4783 = ct{1918};
t4784 = ct{1919};
t4785 = ct{1920};
t4786 = ct{1921};
t4788 = ct{1922};
t4792 = ct{1923};
t4793 = ct{1924};
t4794 = ct{1925};
t4795 = ct{1926};
t4796 = ct{1927};
t4797 = ct{1928};
t4798 = ct{1929};
t48 = ct{1930};
t4807 = ct{1931};
t4813 = ct{1932};
t4815 = ct{1933};
t4816 = ct{1934};
t4817 = ct{1935};
t4822 = ct{1936};
t4824 = ct{1937};
t4825 = ct{1938};
t4826 = ct{1939};
t4828 = ct{1940};
t4829 = ct{1941};
t4830 = ct{1942};
t4831 = ct{1943};
t4833 = ct{1944};
t4836 = ct{1945};
t4837 = ct{1946};
t4838 = ct{1947};
t4839 = ct{1948};
t4840 = ct{1949};
t4841 = ct{1950};
t4843 = ct{1951};
t4845 = ct{1952};
t4846 = ct{1953};
t4849 = ct{1954};
t4850 = ct{1955};
t4851 = ct{1956};
t4855 = ct{1957};
t4856 = ct{1958};
t4857 = ct{1959};
t4858 = ct{1960};
t486 = ct{1961};
t4860 = ct{1962};
t4861 = ct{1963};
t4862 = ct{1964};
t4865 = ct{1965};
t4867 = ct{1966};
t4868 = ct{1967};
t487 = ct{1968};
t4870 = ct{1969};
t4872 = ct{1970};
t4873 = ct{1971};
t4874 = ct{1972};
t4875 = ct{1973};
t4877 = ct{1974};
t4878 = ct{1975};
t4879 = ct{1976};
t488 = ct{1977};
t4881 = ct{1978};
t4883 = ct{1979};
t4887 = ct{1980};
t4888 = ct{1981};
t4889 = ct{1982};
t4890 = ct{1983};
t4891 = ct{1984};
t4892 = ct{1985};
t4894 = ct{1986};
t4895 = ct{1987};
t4896 = ct{1988};
t4897 = ct{1989};
t4900 = ct{1990};
t4902 = ct{1991};
t4913 = ct{1992};
t4914 = ct{1993};
t4915 = ct{1994};
t4916 = ct{1995};
t4917 = ct{1996};
t492 = ct{1997};
t4920 = ct{1998};
t4922 = ct{1999};
t4923 = ct{2000};
t4925 = ct{2001};
t4926 = ct{2002};
t4929 = ct{2003};
t493 = ct{2004};
t4930 = ct{2005};
t4931 = ct{2006};
t4933 = ct{2007};
t4934 = ct{2008};
t4935 = ct{2009};
t4936 = ct{2010};
t4938 = ct{2011};
t494 = ct{2012};
t4941 = ct{2013};
t4943 = ct{2014};
t4946 = ct{2015};
t4947 = ct{2016};
t4949 = ct{2017};
t495 = ct{2018};
t4950 = ct{2019};
t4951 = ct{2020};
t4952 = ct{2021};
t4953 = ct{2022};
t4954 = ct{2023};
t4955 = ct{2024};
t4956 = ct{2025};
t4957 = ct{2026};
t4958 = ct{2027};
t4959 = ct{2028};
t496 = ct{2029};
t4960 = ct{2030};
t4962 = ct{2031};
t4967 = ct{2032};
t4968 = ct{2033};
t4969 = ct{2034};
t497 = ct{2035};
t4971 = ct{2036};
t4975 = ct{2037};
t4977 = ct{2038};
t4978 = ct{2039};
t4979 = ct{2040};
t4981 = ct{2041};
t4983 = ct{2042};
t4985 = ct{2043};
t4990 = ct{2044};
t4991 = ct{2045};
t4992 = ct{2046};
t4993 = ct{2047};
t4995 = ct{2048};
t4996 = ct{2049};
t4997 = ct{2050};
t4d = ct{2051};
t4dd = ct{2052};
t50 = ct{2053};
t5000 = ct{2054};
t5001 = ct{2055};
t5002 = ct{2056};
t5005 = ct{2057};
t5006 = ct{2058};
t5010 = ct{2059};
t5011 = ct{2060};
t5012 = ct{2061};
t5013 = ct{2062};
t5014 = ct{2063};
t5016 = ct{2064};
t5017 = ct{2065};
t5018 = ct{2066};
t5019 = ct{2067};
t5020 = ct{2068};
t5021 = ct{2069};
t5022 = ct{2070};
t5025 = ct{2071};
t5026 = ct{2072};
t5028 = ct{2073};
t5030 = ct{2074};
t5031 = ct{2075};
t5034 = ct{2076};
t5037 = ct{2077};
t5038 = ct{2078};
t5040 = ct{2079};
t5041 = ct{2080};
t5043 = ct{2081};
t5044 = ct{2082};
t5045 = ct{2083};
t5046 = ct{2084};
t5047 = ct{2085};
t5048 = ct{2086};
t5049 = ct{2087};
t5050 = ct{2088};
t5051 = ct{2089};
t5053 = ct{2090};
t5054 = ct{2091};
t5055 = ct{2092};
t5056 = ct{2093};
t5057 = ct{2094};
t5058 = ct{2095};
t5061 = ct{2096};
t5062 = ct{2097};
t5063 = ct{2098};
t5064 = ct{2099};
t5066 = ct{2100};
t5068 = ct{2101};
t5069 = ct{2102};
t5070 = ct{2103};
t5071 = ct{2104};
t5074 = ct{2105};
t5076 = ct{2106};
t5077 = ct{2107};
t5079 = ct{2108};
t508 = ct{2109};
t5081 = ct{2110};
t5084 = ct{2111};
t5092 = ct{2112};
t5093 = ct{2113};
t5096 = ct{2114};
t5097 = ct{2115};
t5098 = ct{2116};
t51 = ct{2117};
t5100 = ct{2118};
t5102 = ct{2119};
t5104 = ct{2120};
t5105 = ct{2121};
t5109 = ct{2122};
t5113 = ct{2123};
t5117 = ct{2124};
t5119 = ct{2125};
t5120 = ct{2126};
t5121 = ct{2127};
t5122 = ct{2128};
t5123 = ct{2129};
t5124 = ct{2130};
t5125 = ct{2131};
t5126 = ct{2132};
t5127 = ct{2133};
t5130 = ct{2134};
t5131 = ct{2135};
t5132 = ct{2136};
t5139 = ct{2137};
t514 = ct{2138};
t5142 = ct{2139};
t5143 = ct{2140};
t5144 = ct{2141};
t5145 = ct{2142};
t5146 = ct{2143};
t5148 = ct{2144};
t5149 = ct{2145};
t515 = ct{2146};
t5151 = ct{2147};
t5153 = ct{2148};
t5155 = ct{2149};
t5158 = ct{2150};
t5159 = ct{2151};
t516 = ct{2152};
t5162 = ct{2153};
t5163 = ct{2154};
t5164 = ct{2155};
t5165 = ct{2156};
t5167 = ct{2157};
t5169 = ct{2158};
t5170 = ct{2159};
t5171 = ct{2160};
t5173 = ct{2161};
t5174 = ct{2162};
t5175 = ct{2163};
t5176 = ct{2164};
t5179 = ct{2165};
t5181 = ct{2166};
t5182 = ct{2167};
t5183 = ct{2168};
t5184 = ct{2169};
t5185 = ct{2170};
t5186 = ct{2171};
t519 = ct{2172};
t5190 = ct{2173};
t5200 = ct{2174};
t5201 = ct{2175};
t5202 = ct{2176};
t5207 = ct{2177};
t5209 = ct{2178};
t5213 = ct{2179};
t5214 = ct{2180};
t5217 = ct{2181};
t5219 = ct{2182};
t5222 = ct{2183};
t5224 = ct{2184};
t5225 = ct{2185};
t5226 = ct{2186};
t5228 = ct{2187};
t523 = ct{2188};
t5231 = ct{2189};
t5234 = ct{2190};
t5235 = ct{2191};
t524 = ct{2192};
t5243 = ct{2193};
t5255 = ct{2194};
t5256 = ct{2195};
t5257 = ct{2196};
t5261 = ct{2197};
t5262 = ct{2198};
t5263 = ct{2199};
t5266 = ct{2200};
t5267 = ct{2201};
t5268 = ct{2202};
t5271 = ct{2203};
t5276 = ct{2204};
t5280 = ct{2205};
t5282 = ct{2206};
t5283 = ct{2207};
t5284 = ct{2208};
t5287 = ct{2209};
t5288 = ct{2210};
t529 = ct{2211};
t5291 = ct{2212};
t5292 = ct{2213};
t5293 = ct{2214};
t5295 = ct{2215};
t5296 = ct{2216};
t5297 = ct{2217};
t5299 = ct{2218};
t53 = ct{2219};
t530 = ct{2220};
t5303 = ct{2221};
t5304 = ct{2222};
t5305 = ct{2223};
t5307 = ct{2224};
t5314 = ct{2225};
t5315 = ct{2226};
t532 = ct{2227};
t5322 = ct{2228};
t5323 = ct{2229};
t5324 = ct{2230};
t5327 = ct{2231};
t5329 = ct{2232};
t5330 = ct{2233};
t5335 = ct{2234};
t5336 = ct{2235};
t5337 = ct{2236};
t5345 = ct{2237};
t5349 = ct{2238};
t5351 = ct{2239};
t5353 = ct{2240};
t5355 = ct{2241};
t5356 = ct{2242};
t5357 = ct{2243};
t5359 = ct{2244};
t5361 = ct{2245};
t5363 = ct{2246};
t5366 = ct{2247};
t5368 = ct{2248};
t5369 = ct{2249};
t537 = ct{2250};
t5370 = ct{2251};
t5373 = ct{2252};
t5374 = ct{2253};
t5375 = ct{2254};
t5397 = ct{2255};
t5401 = ct{2256};
t5403 = ct{2257};
t5413 = ct{2258};
t543 = ct{2259};
t5438 = ct{2260};
t544 = ct{2261};
t546 = ct{2262};
t5465 = ct{2263};
t547 = ct{2264};
t5478 = ct{2265};
t548 = ct{2266};
t5482 = ct{2267};
t55 = ct{2268};
t5503 = ct{2269};
t5505 = ct{2270};
t5514 = ct{2271};
t5515 = ct{2272};
t5517 = ct{2273};
t552 = ct{2274};
t5523 = ct{2275};
t553 = ct{2276};
t554 = ct{2277};
t56 = ct{2278};
t5619 = ct{2279};
t562 = ct{2280};
t569 = ct{2281};
t57 = ct{2282};
t570 = ct{2283};
t58 = ct{2284};
t582 = ct{2285};
t588 = ct{2286};
t589 = ct{2287};
t591 = ct{2288};
t593 = ct{2289};
t598 = ct{2290};
t5d = ct{2291};
t5dd = ct{2292};
t601 = ct{2293};
t602 = ct{2294};
t604 = ct{2295};
t608 = ct{2296};
t609 = ct{2297};
t61 = ct{2298};
t614 = ct{2299};
t615 = ct{2300};
t616 = ct{2301};
t617 = ct{2302};
t623 = ct{2303};
t627 = ct{2304};
t63 = ct{2305};
t632 = ct{2306};
t634 = ct{2307};
t637 = ct{2308};
t639 = ct{2309};
t641 = ct{2310};
t645 = ct{2311};
t646 = ct{2312};
t647 = ct{2313};
t648 = ct{2314};
t649 = ct{2315};
t650 = ct{2316};
t652 = ct{2317};
t653 = ct{2318};
t655 = ct{2319};
t659 = ct{2320};
t670 = ct{2321};
t675 = ct{2322};
t687 = ct{2323};
t69 = ct{2324};
t694 = ct{2325};
t695 = ct{2326};
t696 = ct{2327};
t698 = ct{2328};
t699 = ct{2329};
t6d = ct{2330};
t6dd = ct{2331};
t703 = ct{2332};
t705 = ct{2333};
t706 = ct{2334};
t71 = ct{2335};
t711 = ct{2336};
t712 = ct{2337};
t720 = ct{2338};
t721 = ct{2339};
t723 = ct{2340};
t726 = ct{2341};
t729 = ct{2342};
t732 = ct{2343};
t733 = ct{2344};
t735 = ct{2345};
t736 = ct{2346};
t738 = ct{2347};
t739 = ct{2348};
t745 = ct{2349};
t746 = ct{2350};
t747 = ct{2351};
t748 = ct{2352};
t75 = ct{2353};
t752 = ct{2354};
t755 = ct{2355};
t759 = ct{2356};
t760 = ct{2357};
t761 = ct{2358};
t763 = ct{2359};
t764 = ct{2360};
t775 = ct{2361};
t776 = ct{2362};
t781 = ct{2363};
t785 = ct{2364};
t788 = ct{2365};
t789 = ct{2366};
t793 = ct{2367};
t8 = ct{2368};
t802 = ct{2369};
t806 = ct{2370};
t82 = ct{2371};
t820 = ct{2372};
t824 = ct{2373};
t828 = ct{2374};
t831 = ct{2375};
t832 = ct{2376};
t833 = ct{2377};
t838 = ct{2378};
t842 = ct{2379};
t843 = ct{2380};
t844 = ct{2381};
t846 = ct{2382};
t853 = ct{2383};
t855 = ct{2384};
t859 = ct{2385};
t861 = ct{2386};
t865 = ct{2387};
t870 = ct{2388};
t871 = ct{2389};
t873 = ct{2390};
t879 = ct{2391};
t880 = ct{2392};
t884 = ct{2393};
t885 = ct{2394};
t890 = ct{2395};
t892 = ct{2396};
t896 = ct{2397};
t897 = ct{2398};
t9 = ct{2399};
t900 = ct{2400};
t909 = ct{2401};
t910 = ct{2402};
t919 = ct{2403};
t922 = ct{2404};
t923 = ct{2405};
t927 = ct{2406};
t928 = ct{2407};
t930 = ct{2408};
t932 = ct{2409};
t937 = ct{2410};
t943 = ct{2411};
t949 = ct{2412};
t952 = ct{2413};
t959 = ct{2414};
t961 = ct{2415};
t962 = ct{2416};
t963 = ct{2417};
t964 = ct{2418};
t965 = ct{2419};
t966 = ct{2420};
t969 = ct{2421};
t970 = ct{2422};
t972 = ct{2423};
t973 = ct{2424};
t982 = ct{2425};
t983 = ct{2426};
t986 = ct{2427};
t992 = ct{2428};
t5381 = t14.*t39.*t5370;
t5384 = t330.*t5368;
t5385 = t255.*t5370;
t5429 = t1035+t2018+t2433+t2486+t3329+t3693+t3715;
t5430 = -t6d.*(t986-t2018+t2421+t2475./2.0-t3329+t3684-t3715);
t5431 = t6d.*(t986-t2018+t2421+t2475./2.0-t3329+t3684-t3715);
t5436 = t2322+t2386+t5353;
t5447 = t992+t2005+t2384+t2477+t3547+t3605+t4255;
t5453 = t2112+t3524+t3525+t3526+t4896;
t5475 = t1686+t1966+t1970+t3267+t3268+t3392+t3650+t3667;
t5480 = -t5478;
t5481 = t3120+t3708+t4227+t4228+t4229;
t5621 = -t5d.*(-t2696+t2865-t2935-t3212+t3244-t4550+t4636+t4650+(t14.*t37.*t2233.*(t101-t401))./2.0);
t5622 = t5d.*(-t2696+t2865-t2935-t3212+t3244-t4550+t4636+t4650+(t14.*t37.*t2233.*(t101-t401))./2.0);
t5623 = t4133+t4147+t4361+t4747+t4759+t4828;
t5629 = -t6d.*(t4367+t4760+t4768+t4830+(t8.*t2140.*(t873-t2434))./2.0+(t14.*t2140.*(t910-t2473))./2.0);
t5685 = t4473+t4778+t4949+t4955+t4979+t4997;
t5687 = -t6d.*(t4476+t4784+t4954+t4960+t4992+t5000);
t5720 = -t5d.*(-t3648+t3899-t3933-t4046-t4285+t4292+t5149+t5155+(t37.*(-t1800+t2379+t2497+t18.*t39.*(-t495-t548+t650+t659+t739+t14.*t37.*(t101-t401))))./2.0);
t5721 = t5d.*(-t3648+t3899-t3933-t4046-t4285+t4292+t5149+t5155+(t37.*(-t1800+t2379+t2497+t18.*t39.*(-t495-t548+t650+t659+t739+t14.*t37.*(t101-t401))))./2.0);
t2251 = -t2214;
t2252 = -t2237;
t2253 = -t2238;
t2255 = -t2239;
t2275 = t2214./2.0;
t2598 = -t2564;
t2600 = -t2567;
t2613 = t2564./2.0;
t2615 = t2567./2.0;
t2657 = -t2637;
t2660 = -t2643;
t2667 = t2637./2.0;
t2670 = t2643./2.0;
t2834 = t2805.*t1d;
t2844 = t18.*t2809;
t2846 = t12.*t2814;
t2850 = t18.*t2814;
t2869 = t2809./2.0;
t2872 = t2814./2.0;
t2923 = -t2904;
t2939 = t2909.*t1d;
t2980 = t2931./2.0;
t2986 = -t2973;
t2990 = -t2962;
t3001 = t2963./2.0;
t3119 = -t3094;
t3190 = -t3164;
t3198 = t3133./2.0;
t3222 = -t3202;
t3223 = -t3203;
t3245 = -t3216;
t3261 = t3229./2.0;
t3262 = -t3254;
t3295 = -t3284;
t3296 = -t3270;
t3299 = -t3287;
t3303 = -t3293;
t3315 = -t3309;
t3317 = -t3311;
t3333 = -t3324;
t3337 = -t3320;
t3346 = t3320./2.0;
t3361 = -t3344;
t3393 = t3372.*t1d;
t3396 = -t3382;
t3408 = t18.*t3385;
t3409 = t12.*t3379;
t3411 = t18.*t3379;
t3413 = t3379./2.0;
t3418 = -t3402;
t3420 = -t3398;
t3423 = t3385./2.0;
t3424 = t3386./2.0;
t3437 = -t3412;
t3449 = t3412./2.0;
t3505 = -t3486;
t3511 = -t3501;
t3550 = -t3541;
t3585 = -t3570;
t3616 = -t3592;
t3629 = t3592./2.0;
t3661 = -t3652;
t3676 = -t3663;
t3677 = -t3664;
t3681 = -t3658;
t3714 = -t3698;
t3725 = t3705.*t2d;
t3726 = t3706.*t2d;
t3727 = t3705.*t3d;
t3728 = t3706.*t3d;
t3729 = t3705.*t4d;
t3730 = t3706.*t4d;
t3731 = -t3718;
t3736 = t3695./2.0;
t3740 = t2266+t2285;
t3748 = -t3735;
t3794 = -t3790;
t3814 = -t3801;
t3820 = -t3797;
t3831 = t3797./2.0;
t3837 = -t3824;
t3855 = -t3844;
t3869 = -t3856;
t3879 = -t3870;
t3891 = -t3873;
t3902 = t8.*t3862;
t3914 = -t3881;
t3926 = -t3909;
t3929 = t3881./2.0;
t3947 = -t3930;
t3957 = t3911./2.0;
t3973 = -t3961;
t3988 = -t3981;
t4021 = -t4015;
t4029 = t4015./2.0;
t4044 = -t4039;
t4061 = t2563+t2564;
t4063 = t2567+t2568;
t4114 = -t4100;
t4116 = -t4111;
t4119 = t4104./2.0;
t4120 = t4105./2.0;
t4219 = -t4205;
t4245 = -t4232;
t4248 = -t4239;
t4257 = t4232./2.0;
t4262 = -t4244;
t4274 = t4244./2.0;
t4276 = -t4265;
t4287 = -t4270;
t4288 = -t4271;
t4297 = -t4272;
t4305 = t4278./2.0;
t4310 = -t4300;
t4313 = -t4306;
t4314 = -t4307;
t4322 = t4300./2.0;
t4340 = -t4338;
t4344 = -t4339;
t4354 = -t4343;
t4365 = t4343./2.0;
t4368 = -t4352;
t4380 = -t4369;
t4382 = -t4378;
t4383 = t4369./2.0;
t4384 = t4373./2.0;
t4385 = t18.*t4378;
t4405 = t4401.*t1d;
t4417 = -t4415;
t4434 = t4422.*t2dd;
t4436 = t4422.*t3dd;
t4438 = t4422.*t4dd;
t4447 = -t4435;
t4448 = -t4437;
t4449 = -t4439;
t4477 = t4462./2.0;
t4478 = t4463./2.0;
t4489 = -t4485;
t4495 = t4484./2.0;
t4496 = t4485./2.0;
t4501 = t4490./2.0;
t4504 = t4498./2.0;
t4510 = t4505.*t1d;
t4518 = t4511./2.0;
t4523 = t4516./2.0;
t4524 = -t4521;
t4525 = -t4520;
t4544 = t4530.*t5dd;
t4554 = t4545.*(-1.0./2.0);
t4558 = t4545./2.0;
t4570 = -t4569;
t4610 = t4590./2.0;
t4614 = t4594./2.0;
t4619 = t4603./2.0;
t4628 = t3362+t3369;
t4660 = -t4656;
t4680 = -t4674;
t4682 = t3417+t3462;
t4687 = t1956+t1957+t1958+t2362;
t4718 = -t4711;
t4729 = -t4726;
t4742 = -t4736;
t4743 = t4733.*t1d;
t4746 = -t4735;
t4750 = t4735./2.0;
t4751 = t4740./2.0;
t4756 = t4745./2.0;
t4781 = t4774.*t5d;
t4803 = -t4793;
t4804 = t4797.*t2dd;
t4805 = t4797.*t3dd;
t4806 = t4797.*t4dd;
t4811 = t4793./2.0;
t4832 = t4816./2.0;
t4835 = t4826./2.0;
t4844 = t4839./2.0;
t4852 = -t4850;
t4854 = t4850./2.0;
t4864 = t4857./2.0;
t4876 = -t4872;
t4880 = t4879./2.0;
t4882 = t3782+t3807;
t4899 = -t4897;
t4901 = t4897./2.0;
t4906 = -t4902;
t4918 = t14.*t4913;
t4919 = t8.*t4914;
t4961 = t2809+t3115+t3186;
t4964 = t4962.*t5dd;
t4972 = t4968.*t2d;
t4973 = t4968.*t3d;
t4974 = t4968.*t4d;
t4976 = t4971./2.0;
t4980 = -t4977;
t4982 = t4977./2.0;
t4987 = t4978.*t2d;
t4988 = t4978.*t3d;
t4989 = t4978.*t4d;
t4994 = t4983./2.0;
t4998 = t4996.*t6dd;
t5007 = t5005.*t2d;
t5008 = t5005.*t3d;
t5009 = t5005.*t4d;
t5015 = t2972+t3285+t3297;
t5023 = t1872+t1933+t4500;
t5024 = -t5021;
t5027 = t5021./2.0;
t5033 = -t5031;
t5060 = t1590+t2062+t2711+t3951;
t5067 = t5053./2.0;
t5072 = t5054./2.0;
t5073 = t5055./2.0;
t5082 = t5061./2.0;
t5083 = -t5077;
t5085 = t5063./2.0;
t5086 = t5064./2.0;
t5087 = -t5076;
t5088 = t5079.*t1d;
t5090 = t5076./2.0;
t5101 = -t5100;
t5110 = -t5109;
t5128 = -t5121;
t5129 = -t5122;
t5134 = t5121./2.0;
t5135 = t5122./2.0;
t5147 = t4190+t4234;
t5152 = -t5143;
t5154 = -t5145;
t5156 = t5145./2.0;
t5157 = t5146./2.0;
t5168 = -t5164;
t5172 = t5164./2.0;
t5178 = -t5173;
t5187 = t4243+t4264;
t5189 = t4241+t4261;
t5194 = t5183./2.0;
t5195 = t5184./2.0;
t5216 = -t5214;
t5218 = t3385+t3656+t3680;
t5227 = t5225./2.0;
t5237 = t5234.*t2d;
t5238 = t5234.*t3d;
t5239 = t5234.*t4d;
t5240 = t5235.*t2d;
t5241 = t5235.*t3d;
t5242 = t5235.*t4d;
t5244 = t1160+t5209;
t5245 = t1162+t5207;
t5246 = -t2d.*(t1109-t5209);
t5247 = -t3d.*(t1109-t5209);
t5248 = -t4d.*(t1109-t5209);
t5249 = -t2d.*(t1110-t5207);
t5250 = -t3d.*(t1110-t5207);
t5251 = -t4d.*(t1110-t5207);
t5252 = t2d.*(t1110-t5207);
t5253 = t3d.*(t1110-t5207);
t5254 = t4d.*(t1110-t5207);
t5264 = -t5262;
t5265 = t1790+t1813+t5037;
t5272 = -t5d.*(t2237-t2586+t2588-t3155+t14.*(t1743-t1783));
t5277 = t5276.*t6d;
t5285 = -t5282;
t5294 = -t5291;
t5298 = t3503+t3542+t4474;
t5308 = t1048+t1108+t1237+t1238+t1403+t1472+t3518+t3519;
t5309 = t1047+t1106+t1230+t1236+t1400+t1475+t3514+t3515;
t5310 = -t5307;
t5313 = t712+t1526+t1939+t2009+t2734+t2988+t3059;
t5316 = -t2d.*(t1046+t1185+t1189+t1434-t3519+t158.*t789+t515.*t789+(t8.*(t1609-t2416))./2.0);
t5317 = -t3d.*(t1046+t1185+t1189+t1434-t3519+t158.*t789+t515.*t789+(t8.*(t1609-t2416))./2.0);
t5318 = -t4d.*(t1046+t1185+t1189+t1434-t3519+t158.*t789+t515.*t789+(t8.*(t1609-t2416))./2.0);
t5319 = -t2d.*(t1045+t1183+t1184+t1440-t3514+t155.*t788+t508.*t788+(t14.*(t1597-t2409))./2.0);
t5320 = -t3d.*(t1045+t1183+t1184+t1440-t3514+t155.*t788+t508.*t788+(t14.*(t1597-t2409))./2.0);
t5321 = -t4d.*(t1045+t1183+t1184+t1440-t3514+t155.*t788+t508.*t788+(t14.*(t1597-t2409))./2.0);
t5338 = t5330.*t6d;
t5342 = t247+t2786+t2787+t2788+t4374;
t5343 = t2340+t2344+t5034;
t5360 = t2081+t2087+t5217;
t5364 = t3348+t3354+t4877;
t5365 = t634+t1479+t1885+t1938+t2835+t2959+t3994;
t5371 = t5369./2.0;
t5376 = -t5373;
t5377 = -t5374;
t5378 = t5373./2.0;
t5379 = t5374./2.0;
t5382 = -t5381;
t5383 = t5381./2.0;
t5386 = t5384./2.0;
t5388 = -t5385;
t5389 = t5385./2.0;
t5398 = t1760+t2013+t2031+t3427+t3682+t3707;
t5406 = t4059+t4069+t4868;
t5410 = t3388+t3391+t5179;
t5418 = t2908+t3310+t3312+t3898+t3924;
t5426 = t4387+t4483+t4488;
t5435 = t3248+t3586+t3587+t3588+t3787;
t5437 = t4096+t4102+t4969;
t5439 = t2544+t2561+t4701+t4709;
t5448 = t5447.*t5d;
t5449 = t3199+t3228+t4606+t4607;
t5454 = t5453.*t5d;
t5458 = t1645+t1919+t1921+t3218+t3220+t3376+t3533+t3559;
t5459 = t1586+t1867+t1967+t3218+t3220+t3394+t3539+t3561;
t5460 = -t2d.*(-t1586-t1867+t1920-t3218+t3370+t3535+(t14.*(t1743-t1783))./2.0+t14.*t39.*(t1609-t2416));
t5461 = -t3d.*(-t1586-t1867+t1920-t3218+t3370+t3535+(t14.*(t1743-t1783))./2.0+t14.*t39.*(t1609-t2416));
t5462 = -t4d.*(-t1586-t1867+t1920-t3218+t3370+t3535+(t14.*(t1743-t1783))./2.0+t14.*t39.*(t1609-t2416));
t5466 = t2088+t2317+t2332+t3133+t3173+t3265+t3406+t3430;
t5467 = t1685+t1964+t1993+t3410+t3566+t3583+t4530;
t5470 = -t5d.*(-t1647-t1945+t1992-t2187+t2533-t2534+t3402+t3570+(t14.*t39.*(t1609-t2416))./2.0);
t5473 = t5d.*(-t1647-t1945+t1992-t2187+t2533-t2534+t3402+t3570+(t14.*t39.*(t1609-t2416))./2.0);
t5483 = t3618+t3654+t4780+t4786;
t5494 = t4390+t4391+t4392+t4522;
t5504 = -t6d.*(t2098+t2330./2.0+t2351+t3264./2.0-t3507+t3541-t4797);
t5506 = t2143+t2331+t2373+t3304+t3599+t3610+t4797;
t5551 = t2870+t3161+t3225+t5054+t5063;
t5556 = -t2d.*(-t2021+t2249+t3374+t3395+t4569-t4577+t37.*(t1580+t2001)+t8.*t37.*t1503.*(t100-t364));
t5557 = -t3d.*(-t2021+t2249+t3374+t3395+t4569-t4577+t37.*(t1580+t2001)+t8.*t37.*t1503.*(t100-t364));
t5558 = -t4d.*(-t2021+t2249+t3374+t3395+t4569-t4577+t37.*(t1580+t2001)+t8.*t37.*t1503.*(t100-t364));
t5559 = t2060+t2247+t2294+t3243+t3474+t3492+t4612+t4625;
t5572 = t4259+t4277+t5120+t5123;
t5583 = t2053+t2293+t2330+t3264+t3497+t3512+t4794+t4796;
t5597 = t3798+t4470+t4737+t4738+t4739;
t5601 = t2906+t3301+t3334+t4065+t4375+t4376+t4894;
t5610 = t2958+t3219+t3221+t3246+t3269+t4583+t4723+t4724;
t5611 = t2664+t2843+t2868+t3953+t3979+t4531+t4631+t4645;
t5617 = -t5d.*(-t2188+t2587+t2589+t2973+t3284-t4605-t4731-t4734+(t8.*t37.*(t1743-t1783))./2.0);
t5618 = t5d.*(-t2188+t2587+t2589+t2973+t3284-t4605-t4731-t4734+(t8.*t37.*(t1743-t1783))./2.0);
t5620 = t2696+t2883+t2925+t2935+t3212+t3266+t4550+t4644+t4658;
t5625 = -t2d.*(t3652-t3691-t5369+t5373);
t5626 = -t3d.*(t3652-t3691-t5369+t5373);
t5627 = -t4d.*(t3652-t3691-t5369+t5373);
t5628 = t4146+t4157+t4371+t4757+t4765+t4833;
t5638 = -t6d.*(t2675+t2885-t3385+t3633-t3680-t4527+t4656-t4657+(t892.*t2198)./2.0);
t5668 = t832+t4616+t4617+t4618+t5113+t5224;
t5675 = t2992+t3123+t3163+t4406+t4419+t4745+t4843+t4845;
t5686 = t4481+t4788+t4952+t4959+t4990+t5002;
t5691 = t3696+t3838+t3859+t3942+t3984+t5053+t5146+t5170;
t5696 = t3695+t3925+t3956+t3966+t3999+t5061+t5184+t5200;
t5711 = t3611+t3883+t3887+t4748+t4754+t5047+t5144+t5151;
t5714 = -t5d.*(-t3597+t3930+t4022-t4278+t4300+t5109+(t37.*(t1873+t2355+t2471+t3579))./2.0+(t8.*t39.*(t1862+t2375+t330.*(-t496-t547+t615+t623+t755+t8.*t37.*(t100-t364))+t2124.*(t100-t364)))./2.0+(t14.*t37.*(t2068-t2488))./2.0);
t5718 = t5d.*(-t3597+t3930+t4022-t4278+t4300+t5109+(t37.*(t1873+t2355+t2471+t3579))./2.0+(t8.*t39.*(t1862+t2375+t330.*(-t496-t547+t615+t623+t755+t8.*t37.*(t100-t364))+t2124.*(t100-t364)))./2.0+(t14.*t37.*(t2068-t2488))./2.0);
t5719 = t3648+t3916+t3933+t4046+t4285+t4308+t5056+t5153+t5159;
t5773 = t4104+t4238+t4284+t5263+t5303+t5304+t5305+t5314;
t5787 = t5480+t5503+t5514+t5517;
t2301 = -t2275;
t2676 = -t2667;
t2683 = -t2670;
t2886 = -t2844;
t2888 = -t2850;
t2903 = t2844./2.0;
t2905 = t2846./2.0;
t2907 = t2850./2.0;
t3353 = -t3346;
t3425 = -t3413;
t3434 = -t3408;
t3435 = -t3409;
t3436 = -t3411;
t3438 = -t3423;
t3446 = t3408./2.0;
t3447 = t3409./2.0;
t3448 = t3411./2.0;
t3644 = -t3629;
t3775 = t3740.*t2d;
t3776 = t3740.*t3d;
t3777 = t3740.*t4d;
t3842 = -t3831;
t3946 = -t3929;
t3952 = t3902./2.0;
t4035 = -t4029;
t4123 = -t4119;
t4124 = -t4120;
t4263 = -t4257;
t4289 = -t4274;
t4329 = -t4322;
t4497 = -t4495;
t4502 = -t4501;
t4507 = -t4504;
t4557 = -t4544;
t4696 = t4687.*t2d;
t4697 = t4687.*t3d;
t4698 = t4687.*t4d;
t4753 = -t4743;
t4791 = -t4781;
t4808 = t1079+t1208+t1210+t2597+t2598;
t4809 = t1080+t1209+t1211+t2600+t2601;
t4814 = -t4811;
t4818 = -t4804;
t4819 = -t4805;
t4820 = -t4806;
t4834 = -t4832;
t4847 = -t4844;
t4866 = -t4864;
t4884 = t4882.*t2d;
t4885 = t4882.*t3d;
t4886 = t4882.*t4d;
t4904 = t3819+t3879;
t4905 = -t4901;
t4927 = t4918./2.0;
t4928 = t4919./2.0;
t4963 = t4961.*t5dd;
t4966 = -t4964;
t4986 = -t4982;
t5004 = -t4998;
t5029 = -t5027;
t5075 = -t5067;
t5080 = -t5072;
t5089 = -t5085;
t5094 = -t5090;
t5095 = -t5088;
t5160 = -t5156;
t5161 = -t5157;
t5177 = -t5172;
t5191 = t5187.*t2d;
t5192 = t5187.*t3d;
t5193 = t5187.*t4d;
t5196 = t5189.*t2d;
t5197 = t5189.*t3d;
t5198 = t5189.*t4d;
t5199 = -t5194;
t5220 = t5218.*t5dd;
t5270 = t2252+t2586+t2602+t4492;
t5273 = t2253+t2626+t2627+t3156+t3159;
t5300 = t5298.*t2d;
t5301 = t5298.*t3d;
t5302 = t5298.*t4d;
t5326 = t1147+t1224+t1226+t4269+t4287;
t5331 = t1148+t1225+t1227+t4275+t4288;
t5344 = t5342.*t1d;
t5367 = t5365.*t5d;
t5380 = -t5378;
t5387 = t3426+t5245;
t5393 = -t5389;
t5399 = t5398.*t6d;
t5402 = t4159+t4172+t4680;
t5404 = t2236+t2255+t2350+t2360+t2492+t2528+t2585+t2596;
t5408 = t3683+t3685+t5033;
t5411 = t3681+t5342;
t5416 = t2980+t3261+t3299+t3902+t3935;
t5419 = t2993+t3262+t3282+t3904+t3937;
t5422 = t5418.*t6d;
t5427 = -t6d.*(t4385-t4488+(t330.*(t2578.*(t100-t364)+t609.*(t544-t1021+t330.*(t100-t364))))./2.0);
t5428 = t6d.*(t4385-t4488+(t330.*(t2578.*(t100-t364)+t609.*(t544-t1021+t330.*(t100-t364))))./2.0);
t5432 = t3245+t3536+t3537+t3538+t3787;
t5433 = t3509+t3510+t5216;
t5434 = t4226+t4233+t4876;
t5440 = t5439.*t2d;
t5441 = t5439.*t3d;
t5442 = t5439.*t4d;
t5443 = t3198+t3227+t4567+t4568;
t5450 = t5449.*t2d;
t5451 = t5449.*t3d;
t5452 = t5449.*t4d;
t5455 = -t5454;
t5468 = t1647+t1945+t2012+t3418+t3571+t3585+t4530;
t5469 = t5467.*t5d;
t5471 = t5466.*t5d;
t5477 = t2104+t2289+t2352+t3135+t3174+t3281+t3491+t3511;
t5484 = t5483.*t2d;
t5485 = t5483.*t3d;
t5486 = t5483.*t4d;
t5487 = t3618+t3654+t4803+t4826;
t5491 = t3119+t3805+t4279+t4280+t4281;
t5492 = t1196+t1408+t1588+t1589+t1671+t1683+t2251+t2652+t2673+t2864+t3052+t3065;
t5498 = t3449+t3834+t3869+t4412+t4420;
t5502 = t2115+t2349+t2364+t3280+t3507+t3550+t4797;
t5507 = t5506.*t6d;
t5508 = t3423+t3677+t3718+t4590+t4603;
t5511 = -t5d.*(t3423+t3677+t3718-t4594+t14.*(t3377.*(t100-t364)+t13.*t330.*(t544-t1021+t330.*(t100-t364))));
t5525 = t2126+t2460+t2549+t3003+t3364+t3365+t5147;
t5529 = t3085+t3108+t5124+t5128;
t5533 = t2186+t2215+t2290+t2310+t2532+t2562+t4712+t4718;
t5534 = t3084+t3109+t5129+t5158;
t5542 = t2430+t2615+t2616+t2641+t2657+t4161+t4293+t4295;
t5543 = t2431+t2612+t2613+t2640+t2660+t4163+t4298+t4303;
t5550 = t2869+t3167+t3222+t5055+t5064;
t5552 = t5551.*t5d;
t5555 = t2021+t2246+t2295+t3215+t3397+t3419+t4570+t4577;
t5560 = t5559.*t2d;
t5561 = t5559.*t3d;
t5562 = t5559.*t4d;
Y = ft_11({t100,t1007,t101,t1015,t1016,t1017,t1021,t1026,t1028,t1031,t1036,t104,t1044,t1045,t1046,t1049,t1055,t106,t1066,t1068,t1069,t107,t1070,t1071,t108,t1081,t1082,t1083,t1084,t1085,t1086,t1087,t1093,t1094,t1096,t1097,t1098,t111,t112,t1121,t1122,t1123,t1126,t1128,t1129,t113,t1133,t1134,t1135,t1137,t1138,t1139,t1140,t1155,t1156,t1172,t1174,t1183,t1184,t1185,t1186,t1187,t1189,t1193,t12,t1203,t1222,t124,t1245,t1246,t1247,t1248,t1264,t1265,t1266,t1268,t127,t1271,t1272,t1273,t128,t1281,t1284,t1287,t1288,t1289,t1297,t1298,t13,t1302,t131,t1311,t1312,t1316,t1317,t132,t1321,t1328,t1331,t1332,t1333,t1334,t1335,t134,t1355,t1356,t1357,t1358,t136,t1368,t137,t1375,t1378,t138,t1399,t14,t1410,t1413,t1419,t1420,t1427,t1434,t1440,t1461,t1464,t1465,t1468,t1470,t1485,t1492,t1497,t1499,t15,t150,t1500,t1501,t1503,t1504,t1516,t1517,t1518,t1519,t152,t1520,t1521,t1525,t1528,t1529,t1532,t1534,t1535,t1536,t1537,t1547,t155,t156,t1569,t1571,t1574,t1578,t1579,t158,t1580,t1585,t1586,t159,t1597,t1599,t1606,t1607,t1609,t1610,t1615,t1617,t1618,t162,t163,t1636,t164,t1648,t1649,t165,t1650,t1651,t1652,t1653,t1659,t1663,t1674,t1677,t1678,t1680,t1687,t1692,t1699,t1701,t1704,t1706,t1709,t171,t1710,t1713,t1714,t1715,t173,t1733,t1736,t1738,t174,t1740,t1741,t1742,t1743,t175,t1751,t1754,t1755,t1758,t1759,t177,t1776,t1780,t1783,t1784,t1786,t1792,t1797,t1799,t18,t1800,t1803,t1807,t1815,t1816,t1818,t1827,t1829,t1832,t1835,t1837,t1838,t1840,t1844,t1848,t1849,t1862,t1864,t1866,t1867,t187,t1873,t1874,t1875,t1888,t1889,t1890,t1891,t1892,t19,t1903,t1905,t191,t1916,t1919,t1920,t1921,t1925,t1929,t1930,t1935,t1940,t1944,t1960,t1961,t1962,t1963,t1965,t1968,t1969,t1971,t1973,t1976,t1977,t1983,t1984,t1988,t199,t1995,t1996,t1999,t1d,t1dd,t200,t2001,t2021,t2022,t2026,t2028,t2033,t2044,t2054,t2059,t206,t2061,t2068,t2070,t2074,t2075,t2079,t2080,t2085,t2086,t2090,t2093,t2098,t2099,t21,t2100,t2101,t2113,t2117,t2119,t2122,t2123,t2124,t2128,t2129,t2130,t2136,t2140,t2141,t2142,t2144,t2145,t2147,t215,t2155,t2156,t2167,t2168,t2169,t2170,t2171,t2173,t2174,t2178,t2180,t2184,t2188,t2189,t219,t2190,t2193,t2198,t22,t220,t2203,t2204,t2205,t2206,t2210,t2213,t2222,t2223,t2224,t2225,t2233,t2235,t2243,t2249,t2259,t226,t2270,t2279,t2281,t2286,t229,t2292,t2296,t23,t2300,t2301,t2304,t2305,t2306,t2308,t2311,t232,t2327,t233,t2330,t2339,t2346,t2348,t2351,t2353,t2354,t2355,t2356,t2357,t2358,t2359,t2361,t2363,t2368,t2369,t2371,t2372,t2374,t2375,t2376,t2378,t2379,t2380,t2382,t2387,t2393,t2395,t2398,t2399,t24,t2400,t2401,t2402,t2405,t2406,t2407,t2409,t2412,t2414,t2416,t2427,t2428,t2434,t2438,t244,t2463,t2466,t2467,t2468,t2471,t2472,t2473,t2476,t2478,t2479,t2488,t2490,t2497,t2499,t25,t2500,t2501,t2502,t2503,t2504,t2506,t2507,t2508,t2509,t2510,t2511,t2512,t2513,t2514,t2520,t2523,t2526,t2527,t255,t2550,t2557,t256,t2570,t2574,t2576,t2578,t2583,t2593,t26,t2603,t2606,t2608,t2610,t2614,t2617,t2619,t2625,t2630,t2642,t2644,t2645,t2647,t2648,t2654,t2655,t2658,t2659,t2661,t2664,t2665,t2666,t2668,t2669,t2675,t2676,t2679,t2681,t2682,t2683,t2689,t2690,t2691,t2699,t27,t2703,t2705,t2707,t2708,t2709,t2718,t2719,t2721,t2722,t2724,t2731,t2737,t2743,t2744,t2745,t2747,t2749,t2755,t2758,t2759,t2772,t2775,t2776,t2777,t2779,t2780,t2781,t2782,t2790,t2795,t2796,t2797,t2798,t2807,t2808,t2810,t2813,t2814,t2815,t2816,t2828,t2829,t2830,t2834,t2841,t2842,t2845,t2846,t2847,t2848,t2850,t2853,t2857,t2862,t2867,t2872,t2873,t2874,t2876,t2878,t2882,t2884,t2885,t2886,t2887,t2888,t2890,t2891,t2895,t2899,t29,t2900,t2901,t2902,t2903,t2905,t2907,t2915,t2923,t2929,t2931,t2936,t2937,t2939,t2940,t2946,t2947,t2951,t2953,t2954,t2956,t2958,t2961,t2962,t2963,t2966,t2967,t2968,t2970,t2971,t2973,t2982,t2983,t2984,t2985,t2986,t2989,t299,t2990,t2991,t2994,t2995,t2996,t2997,t2998,t2999,t2d,t2dd,t30,t3000,t3001,t3004,t3007,t3009,t301,t3010,t3011,t3012,t3013,t3014,t3017,t3018,t3029,t3035,t3057,t3058,t3066,t3069,t3073,t3076,t3078,t3079,t308,t3080,t3081,t3082,t3083,t3086,t3087,t3088,t3090,t3098,t3099,t31,t3100,t3101,t3104,t3106,t3107,t3112,t3124,t3125,t3126,t3129,t3130,t3136,t3137,t3138,t3139,t3140,t3143,t3144,t3146,t315,t3151,t3162,t3165,t3166,t317,t3170,t3171,t3172,t3175,t3176,t3177,t318,t3180,t3181,t3182,t3183,t3184,t3185,t3187,t3188,t319,t3190,t3192,t3195,t3196,t3197,t3201,t3204,t3205,t3209,t3210,t3211,t3214,t3217,t3218,t3220,t3223,t3229,t3230,t3231,t3232,t3233,t3234,t3236,t3237,t3239,t3240,t3241,t325,t3251,t3255,t3257,t3258,t3260,t3264,t3270,t3271,t3272,t3273,t3274,t3276,t3277,t3279,t3283,t3288,t3289,t329,t3291,t3292,t3293,t3294,t3295,t3296,t3298,t330,t3300,t3303,t3306,t3308,t3314,t3315,t3316,t3317,t3318,t3321,t3322,t3324,t3326,t3327,t333,t3330,t3331,t3332,t3333,t3335,t3337,t3338,t3339,t3340,t3348,t3349,t3350,t3351,t3353,t3355,t3358,t3359,t3360,t3361,t3369,t3370,t3373,t3374,t3376,t3377,t3378,t3379,t3380,t3381,t3383,t3384,t3385,t3386,t3387,t3389,t3390,t3393,t3395,t3396,t3398,t3399,t34,t3400,t3401,t3404,t3405,t3408,t341,t3411,t3413,t3414,t3415,t3416,t342,t3420,t3421,t3424,t3425,t3429,t343,t3431,t3432,t3434,t3435,t3436,t3437,t3438,t3439,t3440,t3442,t3445,t3446,t3447,t3448,t3452,t3456,t3457,t3458,t3459,t346,t3460,t3461,t3468,t3469,t347,t3472,t3473,t3475,t3477,t3478,t3483,t3486,t3499,t3502,t3505,t3506,t3507,t3514,t3516,t3517,t3519,t3521,t3532,t3533,t3535,t3541,t3543,t3544,t3548,t3549,t3552,t3557,t3558,t3559,t3574,t3575,t3576,t3578,t3579,t3580,t3582,t3590,t3591,t3592,t3594,t3595,t3597,t3598,t36,t3601,t3602,t3603,t3604,t3607,t3608,t3609,t3611,t3613,t3616,t3617,t3620,t3622,t3623,t3624,t3625,t3628,t3629,t3630,t3631,t3632,t3633,t3634,t3635,t3636,t3637,t3638,t3639,t364,t3640,t3643,t3644,t3645,t3646,t3647,t3648,t365,t3652,t3653,t3655,t3657,t3659,t3660,t3661,t3662,t3663,t3664,t3665,t3668,t3669,t3670,t3671,t3672,t3673,t3676,t368,t3680,t3686,t3687,t3689,t3691,t3692,t3694,t37,t3700,t3701,t3702,t3703,t3710,t3711,t3712,t3713,t3714,t3716,t3717,t3719,t3723,t3725,t3726,t3727,t3728,t3729,t3730,t3731,t3732,t3734,t3735,t3736,t3739,t3741,t3742,t3745,t3747,t3748,t3750,t3751,t3754,t3755,t3756,t3757,t3759,t3762,t3770,t3771,t3772,t3773,t3775,t3776,t3777,t3780,t3781,t3785,t3788,t3789,t3793,t3794,t3795,t38,t3800,t3801,t3804,t3808,t3809,t3812,t3814,t3816,t3817,t3818,t3820,t3821,t3822,t3823,t3824,t3825,t3826,t3832,t3833,t3836,t3837,t3839,t3840,t3842,t3843,t3847,t3848,t3855,t3858,t3861,t3862,t3863,t3865,t3866,t3867,t3872,t3874,t3875,t3880,t3882,t3885,t3886,t3888,t3889,t3890,t3891,t3892,t3894,t39,t3900,t3901,t3903,t3911,t3912,t3913,t3914,t3915,t3917,t3919,t392,t3923,t3926,t3927,t3928,t393,t3931,t3932,t3936,t3943,t3944,t3945,t3946,t3947,t3952,t3953,t3955,t3957,t3958,t3960,t3961,t3962,t3964,t3965,t3967,t3969,t3971,t3972,t3973,t3975,t3976,t3977,t3978,t3979,t3982,t3985,t3988,t3989,t3990,t3991,t3992,t3995,t3996,t3997,t3998,t3d,t3dd,t4000,t4001,t4002,t4003,t4005,t4006,t4007,t4009,t401,t4010,t4011,t4012,t4013,t4015,t4016,t4017,t402,t4021,t4023,t4025,t4026,t4027,t403,t4031,t4032,t4033,t4035,t4036,t4037,t4038,t404,t4041,t4042,t4043,t4044,t4047,t4048,t4049,t4050,t4051,t4053,t4060,t4061,t4062,t4063,t4068,t4071,t4074,t4078,t4079,t4084,t4087,t4093,t4094,t4095,t41,t4100,t4101,t4105,t4106,t4108,t4110,t4111,t4114,t4115,t4116,t4117,t4118,t4121,t4122,t4123,t4124,t4125,t4127,t4128,t4130,t4131,t4133,t4136,t4137,t4139,t4143,t4146,t4147,t4149,t4151,t4152,t4154,t4155,t4156,t4157,t4164,t4166,t4167,t4168,t4170,t4171,t4174,t4176,t4178,t418,t4181,t4182,t4183,t4184,t4185,t4186,t4187,t4188,t4189,t419,t4191,t4192,t4193,t4195,t4196,t42,t420,t4200,t4201,t4203,t4204,t4209,t4210,t4211,t4212,t4214,t4219,t4221,t4223,t4224,t4230,t4231,t4235,t4236,t4237,t4239,t4240,t4245,t4247,t4248,t4249,t425,t4250,t4251,t4252,t4253,t4256,t4257,t4260,t4262,t4263,t4266,t4267,t4272,t4274,t4276,t4278,t4282,t4283,t4286,t4289,t4290,t4291,t4296,t4297,t4299,t4301,t4304,t4305,t4309,t431,t4310,t4311,t4313,t4314,t4315,t4316,t4317,t4318,t4319,t4320,t4321,t4323,t4324,t4325,t4327,t4328,t4329,t4330,t4331,t4332,t4335,t4337,t434,t4340,t4343,t4344,t4345,t4347,t4348,t4350,t4353,t4354,t4358,t4359,t4361,t4363,t4364,t4365,t4367,t4368,t4369,t437,t4370,t4371,t4373,t4377,t4380,t4382,t4383,t4384,t4394,t4395,t4399,t4400,t4402,t4404,t4405,t4406,t4408,t441,t4410,t4411,t4413,t4417,t4419,t442,t4421,t4422,t4423,t4424,t4427,t4428,t4429,t443,t4430,t4431,t4433,t4434,t4436,t4438,t4441,t4444,t4445,t4446,t4447,t4448,t4449,t4450,t4451,t4454,t4455,t4456,t4457,t4459,t446,t4460,t4461,t4462,t4463,t4464,t4465,t4467,t4468,t4475,t4476,t4477,t4478,t4479,t4480,t4484,t4487,t4489,t4490,t4491,t4492,t4493,t4494,t4496,t4497,t4498,t4501,t4502,t4503,t4506,t4507,t4508,t4509,t4510,t4511,t4515,t4516,t4518,t4519,t4520,t4523,t4524,t4525,t4526,t4527,t4528,t453,t4531,t4532,t4533,t4534,t4537,t4538,t4539,t454,t4540,t4541,t4542,t4543,t4545,t4546,t4547,t4548,t4551,t4552,t4553,t4556,t4557,t4558,t4559,t4561,t4564,t4569,t4571,t4572,t4575,t4576,t4577,t4578,t4579,t4582,t4586,t4587,t4588,t459,t4591,t4593,t4594,t4595,t4596,t4599,t4601,t4604,t4605,t4608,t4609,t4610,t4614,t4619,t4623,t4626,t4627,t4630,t4631,t4633,t4634,t4635,t4637,t4638,t4639,t4640,t4641,t4642,t4645,t4646,t4647,t4648,t4649,t4651,t4652,t4653,t4655,t4656,t4657,t4659,t4660,t4661,t4662,t4663,t4664,t4665,t4666,t4668,t4670,t4672,t4673,t4674,t4675,t4677,t4678,t4679,t4681,t4684,t4686,t4689,t4690,t4691,t4692,t4694,t4695,t4696,t4697,t4698,t4699,t470,t4700,t4703,t4704,t4705,t4707,t4708,t4713,t4714,t4715,t4716,t4717,t4720,t4721,t4722,t4725,t4726,t4727,t4729,t4730,t4731,t4734,t4735,t4736,t4740,t4741,t4742,t4744,t4746,t4747,t4750,t4751,t4752,t4753,t4756,t4757,t4758,t4759,t4760,t4761,t4762,t4765,t4766,t4767,t4768,t4769,t4770,t4771,t4772,t4776,t478,t4782,t4783,t4784,t4785,t4791,t4792,t4795,t4797,t4798,t48,t4807,t4808,t4809,t4813,t4814,t4815,t4816,t4817,t4818,t4819,t4820,t4822,t4824,t4825,t4829,t4830,t4831,t4833,t4834,t4835,t4836,t4837,t4838,t4839,t4840,t4841,t4846,t4847,t4849,t4850,t4851,t4852,t4854,t4855,t4856,t4857,t4858,t486,t4860,t4861,t4862,t4865,t4866,t4867,t4868,t487,t4870,t4873,t4874,t4875,t4878,t4879,t488,t4880,t4881,t4883,t4884,t4885,t4886,t4887,t4888,t4889,t4890,t4891,t4892,t4894,t4895,t4899,t4900,t4901,t4902,t4904,t4905,t4906,t4913,t4914,t4915,t4916,t4917,t4918,t4919,t492,t4920,t4922,t4923,t4925,t4926,t4927,t4928,t4929,t493,t4930,t4931,t4933,t4934,t4935,t4936,t4938,t494,t4941,t4943,t4946,t4947,t495,t4950,t4951,t4953,t4954,t4956,t4957,t4958,t496,t4960,t4961,t4962,t4963,t4966,t4967,t497,t4971,t4972,t4973,t4974,t4975,t4976,t4977,t4981,t4982,t4983,t4985,t4986,t4987,t4988,t4989,t4991,t4992,t4993,t4994,t4995,t4996,t4d,t4dd,t50,t5000,t5001,t5004,t5006,t5007,t5008,t5009,t5010,t5011,t5012,t5013,t5014,t5016,t5017,t5018,t5019,t5020,t5022,t5024,t5025,t5026,t5027,t5028,t5029,t5030,t5038,t5040,t5041,t5043,t5044,t5045,t5046,t5048,t5049,t5050,t5051,t5057,t5058,t5062,t5066,t5068,t5069,t5070,t5071,t5072,t5073,t5074,t5075,t5076,t5077,t508,t5080,t5081,t5082,t5083,t5084,t5085,t5086,t5088,t5089,t5090,t5092,t5093,t5095,t5096,t5097,t5098,t51,t5101,t5102,t5104,t5105,t5110,t5117,t5119,t5125,t5126,t5127,t5130,t5131,t5132,t5134,t5135,t5139,t514,t5142,t5145,t5147,t5148,t515,t5152,t5154,t5156,t5158,t516,t5160,t5161,t5162,t5163,t5164,t5165,t5167,t5168,t5169,t5171,t5172,t5173,t5174,t5175,t5176,t5177,t5178,t5181,t5182,t5183,t5185,t5186,t519,t5190,t5191,t5192,t5193,t5194,t5195,t5196,t5197,t5198,t5199,t5201,t5202,t5213,t5218,t5219,t5220,t5222,t5225,t5226,t5227,t5228,t523,t5231,t5237,t5238,t5239,t524,t5240,t5241,t5242,t5243,t5246,t5247,t5248,t5252,t5253,t5254,t5255,t5256,t5257,t5261,t5264,t5265,t5266,t5267,t5268,t5271,t5272,t5273,t5277,t5280,t5283,t5284,t5285,t5287,t5288,t529,t5292,t5293,t5294,t5295,t5296,t5297,t5299,t53,t530,t5300,t5301,t5302,t5310,t5315,t5316,t5317,t5318,t5319,t532,t5320,t5321,t5322,t5323,t5324,t5326,t5327,t5329,t5331,t5335,t5336,t5337,t5338,t5343,t5344,t5345,t5349,t5351,t5355,t5356,t5357,t5359,t5360,t5361,t5363,t5366,t5367,t5369,t537,t5371,t5373,t5375,t5376,t5377,t5378,t5379,t5380,t5382,t5383,t5384,t5386,t5387,t5388,t5393,t5397,t5399,t5401,t5403,t5404,t5408,t5410,t5411,t5413,t5416,t5419,t5422,t5427,t5428,t543,t5431,t5432,t5433,t5434,t5435,t5437,t5438,t544,t5440,t5441,t5442,t5443,t5448,t5450,t5451,t5452,t5455,t546,t5465,t5469,t547,t5470,t5471,t5473,t5475,t5477,t548,t5481,t5482,t5484,t5485,t5486,t5487,t5491,t5492,t5494,t5498,t55,t5504,t5505,t5507,t5508,t5511,t5515,t552,t5523,t5525,t5529,t553,t5533,t5534,t554,t5542,t5543,t5550,t5552,t5556,t5557,t5558,t5560,t5561,t5562,t5572,t5583,t56,t5601,t5610,t5618,t5619,t562,t5622,t5625,t5626,t5627,t5629,t5638,t5668,t5675,t5685,t5686,t5687,t569,t5691,t5696,t57,t570,t5711,t5718,t5721,t5773,t5787,t58,t582,t588,t589,t591,t593,t598,t5d,t5dd,t601,t602,t604,t608,t609,t61,t614,t615,t616,t617,t623,t627,t63,t632,t637,t639,t641,t645,t646,t647,t648,t649,t650,t652,t653,t655,t659,t670,t675,t687,t69,t694,t695,t696,t698,t699,t6d,t6dd,t703,t705,t706,t71,t711,t720,t721,t723,t726,t729,t732,t733,t735,t736,t738,t739,t745,t746,t747,t748,t75,t752,t755,t759,t760,t761,t763,t764,t775,t776,t781,t785,t788,t789,t793,t8,t802,t806,t82,t820,t824,t828,t831,t833,t838,t842,t843,t844,t846,t853,t855,t859,t861,t865,t870,t871,t873,t879,t880,t884,t885,t890,t892,t896,t897,t9,t900,t909,t910,t919,t922,t923,t927,t928,t930,t932,t937,t943,t949,t952,t959,t961,t962,t963,t964,t965,t966,t969,t970,t972,t973,t982,t983});
end
function Y = ft_11(ct)
t100 = ct{1};
t1007 = ct{2};
t101 = ct{3};
t1015 = ct{4};
t1016 = ct{5};
t1017 = ct{6};
t1021 = ct{7};
t1026 = ct{8};
t1028 = ct{9};
t1031 = ct{10};
t1036 = ct{11};
t104 = ct{12};
t1044 = ct{13};
t1045 = ct{14};
t1046 = ct{15};
t1049 = ct{16};
t1055 = ct{17};
t106 = ct{18};
t1066 = ct{19};
t1068 = ct{20};
t1069 = ct{21};
t107 = ct{22};
t1070 = ct{23};
t1071 = ct{24};
t108 = ct{25};
t1081 = ct{26};
t1082 = ct{27};
t1083 = ct{28};
t1084 = ct{29};
t1085 = ct{30};
t1086 = ct{31};
t1087 = ct{32};
t1093 = ct{33};
t1094 = ct{34};
t1096 = ct{35};
t1097 = ct{36};
t1098 = ct{37};
t111 = ct{38};
t112 = ct{39};
t1121 = ct{40};
t1122 = ct{41};
t1123 = ct{42};
t1126 = ct{43};
t1128 = ct{44};
t1129 = ct{45};
t113 = ct{46};
t1133 = ct{47};
t1134 = ct{48};
t1135 = ct{49};
t1137 = ct{50};
t1138 = ct{51};
t1139 = ct{52};
t1140 = ct{53};
t1155 = ct{54};
t1156 = ct{55};
t1172 = ct{56};
t1174 = ct{57};
t1183 = ct{58};
t1184 = ct{59};
t1185 = ct{60};
t1186 = ct{61};
t1187 = ct{62};
t1189 = ct{63};
t1193 = ct{64};
t12 = ct{65};
t1203 = ct{66};
t1222 = ct{67};
t124 = ct{68};
t1245 = ct{69};
t1246 = ct{70};
t1247 = ct{71};
t1248 = ct{72};
t1264 = ct{73};
t1265 = ct{74};
t1266 = ct{75};
t1268 = ct{76};
t127 = ct{77};
t1271 = ct{78};
t1272 = ct{79};
t1273 = ct{80};
t128 = ct{81};
t1281 = ct{82};
t1284 = ct{83};
t1287 = ct{84};
t1288 = ct{85};
t1289 = ct{86};
t1297 = ct{87};
t1298 = ct{88};
t13 = ct{89};
t1302 = ct{90};
t131 = ct{91};
t1311 = ct{92};
t1312 = ct{93};
t1316 = ct{94};
t1317 = ct{95};
t132 = ct{96};
t1321 = ct{97};
t1328 = ct{98};
t1331 = ct{99};
t1332 = ct{100};
t1333 = ct{101};
t1334 = ct{102};
t1335 = ct{103};
t134 = ct{104};
t1355 = ct{105};
t1356 = ct{106};
t1357 = ct{107};
t1358 = ct{108};
t136 = ct{109};
t1368 = ct{110};
t137 = ct{111};
t1375 = ct{112};
t1378 = ct{113};
t138 = ct{114};
t1399 = ct{115};
t14 = ct{116};
t1410 = ct{117};
t1413 = ct{118};
t1419 = ct{119};
t1420 = ct{120};
t1427 = ct{121};
t1434 = ct{122};
t1440 = ct{123};
t1461 = ct{124};
t1464 = ct{125};
t1465 = ct{126};
t1468 = ct{127};
t1470 = ct{128};
t1485 = ct{129};
t1492 = ct{130};
t1497 = ct{131};
t1499 = ct{132};
t15 = ct{133};
t150 = ct{134};
t1500 = ct{135};
t1501 = ct{136};
t1503 = ct{137};
t1504 = ct{138};
t1516 = ct{139};
t1517 = ct{140};
t1518 = ct{141};
t1519 = ct{142};
t152 = ct{143};
t1520 = ct{144};
t1521 = ct{145};
t1525 = ct{146};
t1528 = ct{147};
t1529 = ct{148};
t1532 = ct{149};
t1534 = ct{150};
t1535 = ct{151};
t1536 = ct{152};
t1537 = ct{153};
t1547 = ct{154};
t155 = ct{155};
t156 = ct{156};
t1569 = ct{157};
t1571 = ct{158};
t1574 = ct{159};
t1578 = ct{160};
t1579 = ct{161};
t158 = ct{162};
t1580 = ct{163};
t1585 = ct{164};
t1586 = ct{165};
t159 = ct{166};
t1597 = ct{167};
t1599 = ct{168};
t1606 = ct{169};
t1607 = ct{170};
t1609 = ct{171};
t1610 = ct{172};
t1615 = ct{173};
t1617 = ct{174};
t1618 = ct{175};
t162 = ct{176};
t163 = ct{177};
t1636 = ct{178};
t164 = ct{179};
t1648 = ct{180};
t1649 = ct{181};
t165 = ct{182};
t1650 = ct{183};
t1651 = ct{184};
t1652 = ct{185};
t1653 = ct{186};
t1659 = ct{187};
t1663 = ct{188};
t1674 = ct{189};
t1677 = ct{190};
t1678 = ct{191};
t1680 = ct{192};
t1687 = ct{193};
t1692 = ct{194};
t1699 = ct{195};
t1701 = ct{196};
t1704 = ct{197};
t1706 = ct{198};
t1709 = ct{199};
t171 = ct{200};
t1710 = ct{201};
t1713 = ct{202};
t1714 = ct{203};
t1715 = ct{204};
t173 = ct{205};
t1733 = ct{206};
t1736 = ct{207};
t1738 = ct{208};
t174 = ct{209};
t1740 = ct{210};
t1741 = ct{211};
t1742 = ct{212};
t1743 = ct{213};
t175 = ct{214};
t1751 = ct{215};
t1754 = ct{216};
t1755 = ct{217};
t1758 = ct{218};
t1759 = ct{219};
t177 = ct{220};
t1776 = ct{221};
t1780 = ct{222};
t1783 = ct{223};
t1784 = ct{224};
t1786 = ct{225};
t1792 = ct{226};
t1797 = ct{227};
t1799 = ct{228};
t18 = ct{229};
t1800 = ct{230};
t1803 = ct{231};
t1807 = ct{232};
t1815 = ct{233};
t1816 = ct{234};
t1818 = ct{235};
t1827 = ct{236};
t1829 = ct{237};
t1832 = ct{238};
t1835 = ct{239};
t1837 = ct{240};
t1838 = ct{241};
t1840 = ct{242};
t1844 = ct{243};
t1848 = ct{244};
t1849 = ct{245};
t1862 = ct{246};
t1864 = ct{247};
t1866 = ct{248};
t1867 = ct{249};
t187 = ct{250};
t1873 = ct{251};
t1874 = ct{252};
t1875 = ct{253};
t1888 = ct{254};
t1889 = ct{255};
t1890 = ct{256};
t1891 = ct{257};
t1892 = ct{258};
t19 = ct{259};
t1903 = ct{260};
t1905 = ct{261};
t191 = ct{262};
t1916 = ct{263};
t1919 = ct{264};
t1920 = ct{265};
t1921 = ct{266};
t1925 = ct{267};
t1929 = ct{268};
t1930 = ct{269};
t1935 = ct{270};
t1940 = ct{271};
t1944 = ct{272};
t1960 = ct{273};
t1961 = ct{274};
t1962 = ct{275};
t1963 = ct{276};
t1965 = ct{277};
t1968 = ct{278};
t1969 = ct{279};
t1971 = ct{280};
t1973 = ct{281};
t1976 = ct{282};
t1977 = ct{283};
t1983 = ct{284};
t1984 = ct{285};
t1988 = ct{286};
t199 = ct{287};
t1995 = ct{288};
t1996 = ct{289};
t1999 = ct{290};
t1d = ct{291};
t1dd = ct{292};
t200 = ct{293};
t2001 = ct{294};
t2021 = ct{295};
t2022 = ct{296};
t2026 = ct{297};
t2028 = ct{298};
t2033 = ct{299};
t2044 = ct{300};
t2054 = ct{301};
t2059 = ct{302};
t206 = ct{303};
t2061 = ct{304};
t2068 = ct{305};
t2070 = ct{306};
t2074 = ct{307};
t2075 = ct{308};
t2079 = ct{309};
t2080 = ct{310};
t2085 = ct{311};
t2086 = ct{312};
t2090 = ct{313};
t2093 = ct{314};
t2098 = ct{315};
t2099 = ct{316};
t21 = ct{317};
t2100 = ct{318};
t2101 = ct{319};
t2113 = ct{320};
t2117 = ct{321};
t2119 = ct{322};
t2122 = ct{323};
t2123 = ct{324};
t2124 = ct{325};
t2128 = ct{326};
t2129 = ct{327};
t2130 = ct{328};
t2136 = ct{329};
t2140 = ct{330};
t2141 = ct{331};
t2142 = ct{332};
t2144 = ct{333};
t2145 = ct{334};
t2147 = ct{335};
t215 = ct{336};
t2155 = ct{337};
t2156 = ct{338};
t2167 = ct{339};
t2168 = ct{340};
t2169 = ct{341};
t2170 = ct{342};
t2171 = ct{343};
t2173 = ct{344};
t2174 = ct{345};
t2178 = ct{346};
t2180 = ct{347};
t2184 = ct{348};
t2188 = ct{349};
t2189 = ct{350};
t219 = ct{351};
t2190 = ct{352};
t2193 = ct{353};
t2198 = ct{354};
t22 = ct{355};
t220 = ct{356};
t2203 = ct{357};
t2204 = ct{358};
t2205 = ct{359};
t2206 = ct{360};
t2210 = ct{361};
t2213 = ct{362};
t2222 = ct{363};
t2223 = ct{364};
t2224 = ct{365};
t2225 = ct{366};
t2233 = ct{367};
t2235 = ct{368};
t2243 = ct{369};
t2249 = ct{370};
t2259 = ct{371};
t226 = ct{372};
t2270 = ct{373};
t2279 = ct{374};
t2281 = ct{375};
t2286 = ct{376};
t229 = ct{377};
t2292 = ct{378};
t2296 = ct{379};
t23 = ct{380};
t2300 = ct{381};
t2301 = ct{382};
t2304 = ct{383};
t2305 = ct{384};
t2306 = ct{385};
t2308 = ct{386};
t2311 = ct{387};
t232 = ct{388};
t2327 = ct{389};
t233 = ct{390};
t2330 = ct{391};
t2339 = ct{392};
t2346 = ct{393};
t2348 = ct{394};
t2351 = ct{395};
t2353 = ct{396};
t2354 = ct{397};
t2355 = ct{398};
t2356 = ct{399};
t2357 = ct{400};
t2358 = ct{401};
t2359 = ct{402};
t2361 = ct{403};
t2363 = ct{404};
t2368 = ct{405};
t2369 = ct{406};
t2371 = ct{407};
t2372 = ct{408};
t2374 = ct{409};
t2375 = ct{410};
t2376 = ct{411};
t2378 = ct{412};
t2379 = ct{413};
t2380 = ct{414};
t2382 = ct{415};
t2387 = ct{416};
t2393 = ct{417};
t2395 = ct{418};
t2398 = ct{419};
t2399 = ct{420};
t24 = ct{421};
t2400 = ct{422};
t2401 = ct{423};
t2402 = ct{424};
t2405 = ct{425};
t2406 = ct{426};
t2407 = ct{427};
t2409 = ct{428};
t2412 = ct{429};
t2414 = ct{430};
t2416 = ct{431};
t2427 = ct{432};
t2428 = ct{433};
t2434 = ct{434};
t2438 = ct{435};
t244 = ct{436};
t2463 = ct{437};
t2466 = ct{438};
t2467 = ct{439};
t2468 = ct{440};
t2471 = ct{441};
t2472 = ct{442};
t2473 = ct{443};
t2476 = ct{444};
t2478 = ct{445};
t2479 = ct{446};
t2488 = ct{447};
t2490 = ct{448};
t2497 = ct{449};
t2499 = ct{450};
t25 = ct{451};
t2500 = ct{452};
t2501 = ct{453};
t2502 = ct{454};
t2503 = ct{455};
t2504 = ct{456};
t2506 = ct{457};
t2507 = ct{458};
t2508 = ct{459};
t2509 = ct{460};
t2510 = ct{461};
t2511 = ct{462};
t2512 = ct{463};
t2513 = ct{464};
t2514 = ct{465};
t2520 = ct{466};
t2523 = ct{467};
t2526 = ct{468};
t2527 = ct{469};
t255 = ct{470};
t2550 = ct{471};
t2557 = ct{472};
t256 = ct{473};
t2570 = ct{474};
t2574 = ct{475};
t2576 = ct{476};
t2578 = ct{477};
t2583 = ct{478};
t2593 = ct{479};
t26 = ct{480};
t2603 = ct{481};
t2606 = ct{482};
t2608 = ct{483};
t2610 = ct{484};
t2614 = ct{485};
t2617 = ct{486};
t2619 = ct{487};
t2625 = ct{488};
t2630 = ct{489};
t2642 = ct{490};
t2644 = ct{491};
t2645 = ct{492};
t2647 = ct{493};
t2648 = ct{494};
t2654 = ct{495};
t2655 = ct{496};
t2658 = ct{497};
t2659 = ct{498};
t2661 = ct{499};
t2664 = ct{500};
t2665 = ct{501};
t2666 = ct{502};
t2668 = ct{503};
t2669 = ct{504};
t2675 = ct{505};
t2676 = ct{506};
t2679 = ct{507};
t2681 = ct{508};
t2682 = ct{509};
t2683 = ct{510};
t2689 = ct{511};
t2690 = ct{512};
t2691 = ct{513};
t2699 = ct{514};
t27 = ct{515};
t2703 = ct{516};
t2705 = ct{517};
t2707 = ct{518};
t2708 = ct{519};
t2709 = ct{520};
t2718 = ct{521};
t2719 = ct{522};
t2721 = ct{523};
t2722 = ct{524};
t2724 = ct{525};
t2731 = ct{526};
t2737 = ct{527};
t2743 = ct{528};
t2744 = ct{529};
t2745 = ct{530};
t2747 = ct{531};
t2749 = ct{532};
t2755 = ct{533};
t2758 = ct{534};
t2759 = ct{535};
t2772 = ct{536};
t2775 = ct{537};
t2776 = ct{538};
t2777 = ct{539};
t2779 = ct{540};
t2780 = ct{541};
t2781 = ct{542};
t2782 = ct{543};
t2790 = ct{544};
t2795 = ct{545};
t2796 = ct{546};
t2797 = ct{547};
t2798 = ct{548};
t2807 = ct{549};
t2808 = ct{550};
t2810 = ct{551};
t2813 = ct{552};
t2814 = ct{553};
t2815 = ct{554};
t2816 = ct{555};
t2828 = ct{556};
t2829 = ct{557};
t2830 = ct{558};
t2834 = ct{559};
t2841 = ct{560};
t2842 = ct{561};
t2845 = ct{562};
t2846 = ct{563};
t2847 = ct{564};
t2848 = ct{565};
t2850 = ct{566};
t2853 = ct{567};
t2857 = ct{568};
t2862 = ct{569};
t2867 = ct{570};
t2872 = ct{571};
t2873 = ct{572};
t2874 = ct{573};
t2876 = ct{574};
t2878 = ct{575};
t2882 = ct{576};
t2884 = ct{577};
t2885 = ct{578};
t2886 = ct{579};
t2887 = ct{580};
t2888 = ct{581};
t2890 = ct{582};
t2891 = ct{583};
t2895 = ct{584};
t2899 = ct{585};
t29 = ct{586};
t2900 = ct{587};
t2901 = ct{588};
t2902 = ct{589};
t2903 = ct{590};
t2905 = ct{591};
t2907 = ct{592};
t2915 = ct{593};
t2923 = ct{594};
t2929 = ct{595};
t2931 = ct{596};
t2936 = ct{597};
t2937 = ct{598};
t2939 = ct{599};
t2940 = ct{600};
t2946 = ct{601};
t2947 = ct{602};
t2951 = ct{603};
t2953 = ct{604};
t2954 = ct{605};
t2956 = ct{606};
t2958 = ct{607};
t2961 = ct{608};
t2962 = ct{609};
t2963 = ct{610};
t2966 = ct{611};
t2967 = ct{612};
t2968 = ct{613};
t2970 = ct{614};
t2971 = ct{615};
t2973 = ct{616};
t2982 = ct{617};
t2983 = ct{618};
t2984 = ct{619};
t2985 = ct{620};
t2986 = ct{621};
t2989 = ct{622};
t299 = ct{623};
t2990 = ct{624};
t2991 = ct{625};
t2994 = ct{626};
t2995 = ct{627};
t2996 = ct{628};
t2997 = ct{629};
t2998 = ct{630};
t2999 = ct{631};
t2d = ct{632};
t2dd = ct{633};
t30 = ct{634};
t3000 = ct{635};
t3001 = ct{636};
t3004 = ct{637};
t3007 = ct{638};
t3009 = ct{639};
t301 = ct{640};
t3010 = ct{641};
t3011 = ct{642};
t3012 = ct{643};
t3013 = ct{644};
t3014 = ct{645};
t3017 = ct{646};
t3018 = ct{647};
t3029 = ct{648};
t3035 = ct{649};
t3057 = ct{650};
t3058 = ct{651};
t3066 = ct{652};
t3069 = ct{653};
t3073 = ct{654};
t3076 = ct{655};
t3078 = ct{656};
t3079 = ct{657};
t308 = ct{658};
t3080 = ct{659};
t3081 = ct{660};
t3082 = ct{661};
t3083 = ct{662};
t3086 = ct{663};
t3087 = ct{664};
t3088 = ct{665};
t3090 = ct{666};
t3098 = ct{667};
t3099 = ct{668};
t31 = ct{669};
t3100 = ct{670};
t3101 = ct{671};
t3104 = ct{672};
t3106 = ct{673};
t3107 = ct{674};
t3112 = ct{675};
t3124 = ct{676};
t3125 = ct{677};
t3126 = ct{678};
t3129 = ct{679};
t3130 = ct{680};
t3136 = ct{681};
t3137 = ct{682};
t3138 = ct{683};
t3139 = ct{684};
t3140 = ct{685};
t3143 = ct{686};
t3144 = ct{687};
t3146 = ct{688};
t315 = ct{689};
t3151 = ct{690};
t3162 = ct{691};
t3165 = ct{692};
t3166 = ct{693};
t317 = ct{694};
t3170 = ct{695};
t3171 = ct{696};
t3172 = ct{697};
t3175 = ct{698};
t3176 = ct{699};
t3177 = ct{700};
t318 = ct{701};
t3180 = ct{702};
t3181 = ct{703};
t3182 = ct{704};
t3183 = ct{705};
t3184 = ct{706};
t3185 = ct{707};
t3187 = ct{708};
t3188 = ct{709};
t319 = ct{710};
t3190 = ct{711};
t3192 = ct{712};
t3195 = ct{713};
t3196 = ct{714};
t3197 = ct{715};
t3201 = ct{716};
t3204 = ct{717};
t3205 = ct{718};
t3209 = ct{719};
t3210 = ct{720};
t3211 = ct{721};
t3214 = ct{722};
t3217 = ct{723};
t3218 = ct{724};
t3220 = ct{725};
t3223 = ct{726};
t3229 = ct{727};
t3230 = ct{728};
t3231 = ct{729};
t3232 = ct{730};
t3233 = ct{731};
t3234 = ct{732};
t3236 = ct{733};
t3237 = ct{734};
t3239 = ct{735};
t3240 = ct{736};
t3241 = ct{737};
t325 = ct{738};
t3251 = ct{739};
t3255 = ct{740};
t3257 = ct{741};
t3258 = ct{742};
t3260 = ct{743};
t3264 = ct{744};
t3270 = ct{745};
t3271 = ct{746};
t3272 = ct{747};
t3273 = ct{748};
t3274 = ct{749};
t3276 = ct{750};
t3277 = ct{751};
t3279 = ct{752};
t3283 = ct{753};
t3288 = ct{754};
t3289 = ct{755};
t329 = ct{756};
t3291 = ct{757};
t3292 = ct{758};
t3293 = ct{759};
t3294 = ct{760};
t3295 = ct{761};
t3296 = ct{762};
t3298 = ct{763};
t330 = ct{764};
t3300 = ct{765};
t3303 = ct{766};
t3306 = ct{767};
t3308 = ct{768};
t3314 = ct{769};
t3315 = ct{770};
t3316 = ct{771};
t3317 = ct{772};
t3318 = ct{773};
t3321 = ct{774};
t3322 = ct{775};
t3324 = ct{776};
t3326 = ct{777};
t3327 = ct{778};
t333 = ct{779};
t3330 = ct{780};
t3331 = ct{781};
t3332 = ct{782};
t3333 = ct{783};
t3335 = ct{784};
t3337 = ct{785};
t3338 = ct{786};
t3339 = ct{787};
t3340 = ct{788};
t3348 = ct{789};
t3349 = ct{790};
t3350 = ct{791};
t3351 = ct{792};
t3353 = ct{793};
t3355 = ct{794};
t3358 = ct{795};
t3359 = ct{796};
t3360 = ct{797};
t3361 = ct{798};
t3369 = ct{799};
t3370 = ct{800};
t3373 = ct{801};
t3374 = ct{802};
t3376 = ct{803};
t3377 = ct{804};
t3378 = ct{805};
t3379 = ct{806};
t3380 = ct{807};
t3381 = ct{808};
t3383 = ct{809};
t3384 = ct{810};
t3385 = ct{811};
t3386 = ct{812};
t3387 = ct{813};
t3389 = ct{814};
t3390 = ct{815};
t3393 = ct{816};
t3395 = ct{817};
t3396 = ct{818};
t3398 = ct{819};
t3399 = ct{820};
t34 = ct{821};
t3400 = ct{822};
t3401 = ct{823};
t3404 = ct{824};
t3405 = ct{825};
t3408 = ct{826};
t341 = ct{827};
t3411 = ct{828};
t3413 = ct{829};
t3414 = ct{830};
t3415 = ct{831};
t3416 = ct{832};
t342 = ct{833};
t3420 = ct{834};
t3421 = ct{835};
t3424 = ct{836};
t3425 = ct{837};
t3429 = ct{838};
t343 = ct{839};
t3431 = ct{840};
t3432 = ct{841};
t3434 = ct{842};
t3435 = ct{843};
t3436 = ct{844};
t3437 = ct{845};
t3438 = ct{846};
t3439 = ct{847};
t3440 = ct{848};
t3442 = ct{849};
t3445 = ct{850};
t3446 = ct{851};
t3447 = ct{852};
t3448 = ct{853};
t3452 = ct{854};
t3456 = ct{855};
t3457 = ct{856};
t3458 = ct{857};
t3459 = ct{858};
t346 = ct{859};
t3460 = ct{860};
t3461 = ct{861};
t3468 = ct{862};
t3469 = ct{863};
t347 = ct{864};
t3472 = ct{865};
t3473 = ct{866};
t3475 = ct{867};
t3477 = ct{868};
t3478 = ct{869};
t3483 = ct{870};
t3486 = ct{871};
t3499 = ct{872};
t3502 = ct{873};
t3505 = ct{874};
t3506 = ct{875};
t3507 = ct{876};
t3514 = ct{877};
t3516 = ct{878};
t3517 = ct{879};
t3519 = ct{880};
t3521 = ct{881};
t3532 = ct{882};
t3533 = ct{883};
t3535 = ct{884};
t3541 = ct{885};
t3543 = ct{886};
t3544 = ct{887};
t3548 = ct{888};
t3549 = ct{889};
t3552 = ct{890};
t3557 = ct{891};
t3558 = ct{892};
t3559 = ct{893};
t3574 = ct{894};
t3575 = ct{895};
t3576 = ct{896};
t3578 = ct{897};
t3579 = ct{898};
t3580 = ct{899};
t3582 = ct{900};
t3590 = ct{901};
t3591 = ct{902};
t3592 = ct{903};
t3594 = ct{904};
t3595 = ct{905};
t3597 = ct{906};
t3598 = ct{907};
t36 = ct{908};
t3601 = ct{909};
t3602 = ct{910};
t3603 = ct{911};
t3604 = ct{912};
t3607 = ct{913};
t3608 = ct{914};
t3609 = ct{915};
t3611 = ct{916};
t3613 = ct{917};
t3616 = ct{918};
t3617 = ct{919};
t3620 = ct{920};
t3622 = ct{921};
t3623 = ct{922};
t3624 = ct{923};
t3625 = ct{924};
t3628 = ct{925};
t3629 = ct{926};
t3630 = ct{927};
t3631 = ct{928};
t3632 = ct{929};
t3633 = ct{930};
t3634 = ct{931};
t3635 = ct{932};
t3636 = ct{933};
t3637 = ct{934};
t3638 = ct{935};
t3639 = ct{936};
t364 = ct{937};
t3640 = ct{938};
t3643 = ct{939};
t3644 = ct{940};
t3645 = ct{941};
t3646 = ct{942};
t3647 = ct{943};
t3648 = ct{944};
t365 = ct{945};
t3652 = ct{946};
t3653 = ct{947};
t3655 = ct{948};
t3657 = ct{949};
t3659 = ct{950};
t3660 = ct{951};
t3661 = ct{952};
t3662 = ct{953};
t3663 = ct{954};
t3664 = ct{955};
t3665 = ct{956};
t3668 = ct{957};
t3669 = ct{958};
t3670 = ct{959};
t3671 = ct{960};
t3672 = ct{961};
t3673 = ct{962};
t3676 = ct{963};
t368 = ct{964};
t3680 = ct{965};
t3686 = ct{966};
t3687 = ct{967};
t3689 = ct{968};
t3691 = ct{969};
t3692 = ct{970};
t3694 = ct{971};
t37 = ct{972};
t3700 = ct{973};
t3701 = ct{974};
t3702 = ct{975};
t3703 = ct{976};
t3710 = ct{977};
t3711 = ct{978};
t3712 = ct{979};
t3713 = ct{980};
t3714 = ct{981};
t3716 = ct{982};
t3717 = ct{983};
t3719 = ct{984};
t3723 = ct{985};
t3725 = ct{986};
t3726 = ct{987};
t3727 = ct{988};
t3728 = ct{989};
t3729 = ct{990};
t3730 = ct{991};
t3731 = ct{992};
t3732 = ct{993};
t3734 = ct{994};
t3735 = ct{995};
t3736 = ct{996};
t3739 = ct{997};
t3741 = ct{998};
t3742 = ct{999};
t3745 = ct{1000};
t3747 = ct{1001};
t3748 = ct{1002};
t3750 = ct{1003};
t3751 = ct{1004};
t3754 = ct{1005};
t3755 = ct{1006};
t3756 = ct{1007};
t3757 = ct{1008};
t3759 = ct{1009};
t3762 = ct{1010};
t3770 = ct{1011};
t3771 = ct{1012};
t3772 = ct{1013};
t3773 = ct{1014};
t3775 = ct{1015};
t3776 = ct{1016};
t3777 = ct{1017};
t3780 = ct{1018};
t3781 = ct{1019};
t3785 = ct{1020};
t3788 = ct{1021};
t3789 = ct{1022};
t3793 = ct{1023};
t3794 = ct{1024};
t3795 = ct{1025};
t38 = ct{1026};
t3800 = ct{1027};
t3801 = ct{1028};
t3804 = ct{1029};
t3808 = ct{1030};
t3809 = ct{1031};
t3812 = ct{1032};
t3814 = ct{1033};
t3816 = ct{1034};
t3817 = ct{1035};
t3818 = ct{1036};
t3820 = ct{1037};
t3821 = ct{1038};
t3822 = ct{1039};
t3823 = ct{1040};
t3824 = ct{1041};
t3825 = ct{1042};
t3826 = ct{1043};
t3832 = ct{1044};
t3833 = ct{1045};
t3836 = ct{1046};
t3837 = ct{1047};
t3839 = ct{1048};
t3840 = ct{1049};
t3842 = ct{1050};
t3843 = ct{1051};
t3847 = ct{1052};
t3848 = ct{1053};
t3855 = ct{1054};
t3858 = ct{1055};
t3861 = ct{1056};
t3862 = ct{1057};
t3863 = ct{1058};
t3865 = ct{1059};
t3866 = ct{1060};
t3867 = ct{1061};
t3872 = ct{1062};
t3874 = ct{1063};
t3875 = ct{1064};
t3880 = ct{1065};
t3882 = ct{1066};
t3885 = ct{1067};
t3886 = ct{1068};
t3888 = ct{1069};
t3889 = ct{1070};
t3890 = ct{1071};
t3891 = ct{1072};
t3892 = ct{1073};
t3894 = ct{1074};
t39 = ct{1075};
t3900 = ct{1076};
t3901 = ct{1077};
t3903 = ct{1078};
t3911 = ct{1079};
t3912 = ct{1080};
t3913 = ct{1081};
t3914 = ct{1082};
t3915 = ct{1083};
t3917 = ct{1084};
t3919 = ct{1085};
t392 = ct{1086};
t3923 = ct{1087};
t3926 = ct{1088};
t3927 = ct{1089};
t3928 = ct{1090};
t393 = ct{1091};
t3931 = ct{1092};
t3932 = ct{1093};
t3936 = ct{1094};
t3943 = ct{1095};
t3944 = ct{1096};
t3945 = ct{1097};
t3946 = ct{1098};
t3947 = ct{1099};
t3952 = ct{1100};
t3953 = ct{1101};
t3955 = ct{1102};
t3957 = ct{1103};
t3958 = ct{1104};
t3960 = ct{1105};
t3961 = ct{1106};
t3962 = ct{1107};
t3964 = ct{1108};
t3965 = ct{1109};
t3967 = ct{1110};
t3969 = ct{1111};
t3971 = ct{1112};
t3972 = ct{1113};
t3973 = ct{1114};
t3975 = ct{1115};
t3976 = ct{1116};
t3977 = ct{1117};
t3978 = ct{1118};
t3979 = ct{1119};
t3982 = ct{1120};
t3985 = ct{1121};
t3988 = ct{1122};
t3989 = ct{1123};
t3990 = ct{1124};
t3991 = ct{1125};
t3992 = ct{1126};
t3995 = ct{1127};
t3996 = ct{1128};
t3997 = ct{1129};
t3998 = ct{1130};
t3d = ct{1131};
t3dd = ct{1132};
t4000 = ct{1133};
t4001 = ct{1134};
t4002 = ct{1135};
t4003 = ct{1136};
t4005 = ct{1137};
t4006 = ct{1138};
t4007 = ct{1139};
t4009 = ct{1140};
t401 = ct{1141};
t4010 = ct{1142};
t4011 = ct{1143};
t4012 = ct{1144};
t4013 = ct{1145};
t4015 = ct{1146};
t4016 = ct{1147};
t4017 = ct{1148};
t402 = ct{1149};
t4021 = ct{1150};
t4023 = ct{1151};
t4025 = ct{1152};
t4026 = ct{1153};
t4027 = ct{1154};
t403 = ct{1155};
t4031 = ct{1156};
t4032 = ct{1157};
t4033 = ct{1158};
t4035 = ct{1159};
t4036 = ct{1160};
t4037 = ct{1161};
t4038 = ct{1162};
t404 = ct{1163};
t4041 = ct{1164};
t4042 = ct{1165};
t4043 = ct{1166};
t4044 = ct{1167};
t4047 = ct{1168};
t4048 = ct{1169};
t4049 = ct{1170};
t4050 = ct{1171};
t4051 = ct{1172};
t4053 = ct{1173};
t4060 = ct{1174};
t4061 = ct{1175};
t4062 = ct{1176};
t4063 = ct{1177};
t4068 = ct{1178};
t4071 = ct{1179};
t4074 = ct{1180};
t4078 = ct{1181};
t4079 = ct{1182};
t4084 = ct{1183};
t4087 = ct{1184};
t4093 = ct{1185};
t4094 = ct{1186};
t4095 = ct{1187};
t41 = ct{1188};
t4100 = ct{1189};
t4101 = ct{1190};
t4105 = ct{1191};
t4106 = ct{1192};
t4108 = ct{1193};
t4110 = ct{1194};
t4111 = ct{1195};
t4114 = ct{1196};
t4115 = ct{1197};
t4116 = ct{1198};
t4117 = ct{1199};
t4118 = ct{1200};
t4121 = ct{1201};
t4122 = ct{1202};
t4123 = ct{1203};
t4124 = ct{1204};
t4125 = ct{1205};
t4127 = ct{1206};
t4128 = ct{1207};
t4130 = ct{1208};
t4131 = ct{1209};
t4133 = ct{1210};
t4136 = ct{1211};
t4137 = ct{1212};
t4139 = ct{1213};
t4143 = ct{1214};
t4146 = ct{1215};
t4147 = ct{1216};
t4149 = ct{1217};
t4151 = ct{1218};
t4152 = ct{1219};
t4154 = ct{1220};
t4155 = ct{1221};
t4156 = ct{1222};
t4157 = ct{1223};
t4164 = ct{1224};
t4166 = ct{1225};
t4167 = ct{1226};
t4168 = ct{1227};
t4170 = ct{1228};
t4171 = ct{1229};
t4174 = ct{1230};
t4176 = ct{1231};
t4178 = ct{1232};
t418 = ct{1233};
t4181 = ct{1234};
t4182 = ct{1235};
t4183 = ct{1236};
t4184 = ct{1237};
t4185 = ct{1238};
t4186 = ct{1239};
t4187 = ct{1240};
t4188 = ct{1241};
t4189 = ct{1242};
t419 = ct{1243};
t4191 = ct{1244};
t4192 = ct{1245};
t4193 = ct{1246};
t4195 = ct{1247};
t4196 = ct{1248};
t42 = ct{1249};
t420 = ct{1250};
t4200 = ct{1251};
t4201 = ct{1252};
t4203 = ct{1253};
t4204 = ct{1254};
t4209 = ct{1255};
t4210 = ct{1256};
t4211 = ct{1257};
t4212 = ct{1258};
t4214 = ct{1259};
t4219 = ct{1260};
t4221 = ct{1261};
t4223 = ct{1262};
t4224 = ct{1263};
t4230 = ct{1264};
t4231 = ct{1265};
t4235 = ct{1266};
t4236 = ct{1267};
t4237 = ct{1268};
t4239 = ct{1269};
t4240 = ct{1270};
t4245 = ct{1271};
t4247 = ct{1272};
t4248 = ct{1273};
t4249 = ct{1274};
t425 = ct{1275};
t4250 = ct{1276};
t4251 = ct{1277};
t4252 = ct{1278};
t4253 = ct{1279};
t4256 = ct{1280};
t4257 = ct{1281};
t4260 = ct{1282};
t4262 = ct{1283};
t4263 = ct{1284};
t4266 = ct{1285};
t4267 = ct{1286};
t4272 = ct{1287};
t4274 = ct{1288};
t4276 = ct{1289};
t4278 = ct{1290};
t4282 = ct{1291};
t4283 = ct{1292};
t4286 = ct{1293};
t4289 = ct{1294};
t4290 = ct{1295};
t4291 = ct{1296};
t4296 = ct{1297};
t4297 = ct{1298};
t4299 = ct{1299};
t4301 = ct{1300};
t4304 = ct{1301};
t4305 = ct{1302};
t4309 = ct{1303};
t431 = ct{1304};
t4310 = ct{1305};
t4311 = ct{1306};
t4313 = ct{1307};
t4314 = ct{1308};
t4315 = ct{1309};
t4316 = ct{1310};
t4317 = ct{1311};
t4318 = ct{1312};
t4319 = ct{1313};
t4320 = ct{1314};
t4321 = ct{1315};
t4323 = ct{1316};
t4324 = ct{1317};
t4325 = ct{1318};
t4327 = ct{1319};
t4328 = ct{1320};
t4329 = ct{1321};
t4330 = ct{1322};
t4331 = ct{1323};
t4332 = ct{1324};
t4335 = ct{1325};
t4337 = ct{1326};
t434 = ct{1327};
t4340 = ct{1328};
t4343 = ct{1329};
t4344 = ct{1330};
t4345 = ct{1331};
t4347 = ct{1332};
t4348 = ct{1333};
t4350 = ct{1334};
t4353 = ct{1335};
t4354 = ct{1336};
t4358 = ct{1337};
t4359 = ct{1338};
t4361 = ct{1339};
t4363 = ct{1340};
t4364 = ct{1341};
t4365 = ct{1342};
t4367 = ct{1343};
t4368 = ct{1344};
t4369 = ct{1345};
t437 = ct{1346};
t4370 = ct{1347};
t4371 = ct{1348};
t4373 = ct{1349};
t4377 = ct{1350};
t4380 = ct{1351};
t4382 = ct{1352};
t4383 = ct{1353};
t4384 = ct{1354};
t4394 = ct{1355};
t4395 = ct{1356};
t4399 = ct{1357};
t4400 = ct{1358};
t4402 = ct{1359};
t4404 = ct{1360};
t4405 = ct{1361};
t4406 = ct{1362};
t4408 = ct{1363};
t441 = ct{1364};
t4410 = ct{1365};
t4411 = ct{1366};
t4413 = ct{1367};
t4417 = ct{1368};
t4419 = ct{1369};
t442 = ct{1370};
t4421 = ct{1371};
t4422 = ct{1372};
t4423 = ct{1373};
t4424 = ct{1374};
t4427 = ct{1375};
t4428 = ct{1376};
t4429 = ct{1377};
t443 = ct{1378};
t4430 = ct{1379};
t4431 = ct{1380};
t4433 = ct{1381};
t4434 = ct{1382};
t4436 = ct{1383};
t4438 = ct{1384};
t4441 = ct{1385};
t4444 = ct{1386};
t4445 = ct{1387};
t4446 = ct{1388};
t4447 = ct{1389};
t4448 = ct{1390};
t4449 = ct{1391};
t4450 = ct{1392};
t4451 = ct{1393};
t4454 = ct{1394};
t4455 = ct{1395};
t4456 = ct{1396};
t4457 = ct{1397};
t4459 = ct{1398};
t446 = ct{1399};
t4460 = ct{1400};
t4461 = ct{1401};
t4462 = ct{1402};
t4463 = ct{1403};
t4464 = ct{1404};
t4465 = ct{1405};
t4467 = ct{1406};
t4468 = ct{1407};
t4475 = ct{1408};
t4476 = ct{1409};
t4477 = ct{1410};
t4478 = ct{1411};
t4479 = ct{1412};
t4480 = ct{1413};
t4484 = ct{1414};
t4487 = ct{1415};
t4489 = ct{1416};
t4490 = ct{1417};
t4491 = ct{1418};
t4492 = ct{1419};
t4493 = ct{1420};
t4494 = ct{1421};
t4496 = ct{1422};
t4497 = ct{1423};
t4498 = ct{1424};
t4501 = ct{1425};
t4502 = ct{1426};
t4503 = ct{1427};
t4506 = ct{1428};
t4507 = ct{1429};
t4508 = ct{1430};
t4509 = ct{1431};
t4510 = ct{1432};
t4511 = ct{1433};
t4515 = ct{1434};
t4516 = ct{1435};
t4518 = ct{1436};
t4519 = ct{1437};
t4520 = ct{1438};
t4523 = ct{1439};
t4524 = ct{1440};
t4525 = ct{1441};
t4526 = ct{1442};
t4527 = ct{1443};
t4528 = ct{1444};
t453 = ct{1445};
t4531 = ct{1446};
t4532 = ct{1447};
t4533 = ct{1448};
t4534 = ct{1449};
t4537 = ct{1450};
t4538 = ct{1451};
t4539 = ct{1452};
t454 = ct{1453};
t4540 = ct{1454};
t4541 = ct{1455};
t4542 = ct{1456};
t4543 = ct{1457};
t4545 = ct{1458};
t4546 = ct{1459};
t4547 = ct{1460};
t4548 = ct{1461};
t4551 = ct{1462};
t4552 = ct{1463};
t4553 = ct{1464};
t4556 = ct{1465};
t4557 = ct{1466};
t4558 = ct{1467};
t4559 = ct{1468};
t4561 = ct{1469};
t4564 = ct{1470};
t4569 = ct{1471};
t4571 = ct{1472};
t4572 = ct{1473};
t4575 = ct{1474};
t4576 = ct{1475};
t4577 = ct{1476};
t4578 = ct{1477};
t4579 = ct{1478};
t4582 = ct{1479};
t4586 = ct{1480};
t4587 = ct{1481};
t4588 = ct{1482};
t459 = ct{1483};
t4591 = ct{1484};
t4593 = ct{1485};
t4594 = ct{1486};
t4595 = ct{1487};
t4596 = ct{1488};
t4599 = ct{1489};
t4601 = ct{1490};
t4604 = ct{1491};
t4605 = ct{1492};
t4608 = ct{1493};
t4609 = ct{1494};
t4610 = ct{1495};
t4614 = ct{1496};
t4619 = ct{1497};
t4623 = ct{1498};
t4626 = ct{1499};
t4627 = ct{1500};
t4630 = ct{1501};
t4631 = ct{1502};
t4633 = ct{1503};
t4634 = ct{1504};
t4635 = ct{1505};
t4637 = ct{1506};
t4638 = ct{1507};
t4639 = ct{1508};
t4640 = ct{1509};
t4641 = ct{1510};
t4642 = ct{1511};
t4645 = ct{1512};
t4646 = ct{1513};
t4647 = ct{1514};
t4648 = ct{1515};
t4649 = ct{1516};
t4651 = ct{1517};
t4652 = ct{1518};
t4653 = ct{1519};
t4655 = ct{1520};
t4656 = ct{1521};
t4657 = ct{1522};
t4659 = ct{1523};
t4660 = ct{1524};
t4661 = ct{1525};
t4662 = ct{1526};
t4663 = ct{1527};
t4664 = ct{1528};
t4665 = ct{1529};
t4666 = ct{1530};
t4668 = ct{1531};
t4670 = ct{1532};
t4672 = ct{1533};
t4673 = ct{1534};
t4674 = ct{1535};
t4675 = ct{1536};
t4677 = ct{1537};
t4678 = ct{1538};
t4679 = ct{1539};
t4681 = ct{1540};
t4684 = ct{1541};
t4686 = ct{1542};
t4689 = ct{1543};
t4690 = ct{1544};
t4691 = ct{1545};
t4692 = ct{1546};
t4694 = ct{1547};
t4695 = ct{1548};
t4696 = ct{1549};
t4697 = ct{1550};
t4698 = ct{1551};
t4699 = ct{1552};
t470 = ct{1553};
t4700 = ct{1554};
t4703 = ct{1555};
t4704 = ct{1556};
t4705 = ct{1557};
t4707 = ct{1558};
t4708 = ct{1559};
t4713 = ct{1560};
t4714 = ct{1561};
t4715 = ct{1562};
t4716 = ct{1563};
t4717 = ct{1564};
t4720 = ct{1565};
t4721 = ct{1566};
t4722 = ct{1567};
t4725 = ct{1568};
t4726 = ct{1569};
t4727 = ct{1570};
t4729 = ct{1571};
t4730 = ct{1572};
t4731 = ct{1573};
t4734 = ct{1574};
t4735 = ct{1575};
t4736 = ct{1576};
t4740 = ct{1577};
t4741 = ct{1578};
t4742 = ct{1579};
t4744 = ct{1580};
t4746 = ct{1581};
t4747 = ct{1582};
t4750 = ct{1583};
t4751 = ct{1584};
t4752 = ct{1585};
t4753 = ct{1586};
t4756 = ct{1587};
t4757 = ct{1588};
t4758 = ct{1589};
t4759 = ct{1590};
t4760 = ct{1591};
t4761 = ct{1592};
t4762 = ct{1593};
t4765 = ct{1594};
t4766 = ct{1595};
t4767 = ct{1596};
t4768 = ct{1597};
t4769 = ct{1598};
t4770 = ct{1599};
t4771 = ct{1600};
t4772 = ct{1601};
t4776 = ct{1602};
t478 = ct{1603};
t4782 = ct{1604};
t4783 = ct{1605};
t4784 = ct{1606};
t4785 = ct{1607};
t4791 = ct{1608};
t4792 = ct{1609};
t4795 = ct{1610};
t4797 = ct{1611};
t4798 = ct{1612};
t48 = ct{1613};
t4807 = ct{1614};
t4808 = ct{1615};
t4809 = ct{1616};
t4813 = ct{1617};
t4814 = ct{1618};
t4815 = ct{1619};
t4816 = ct{1620};
t4817 = ct{1621};
t4818 = ct{1622};
t4819 = ct{1623};
t4820 = ct{1624};
t4822 = ct{1625};
t4824 = ct{1626};
t4825 = ct{1627};
t4829 = ct{1628};
t4830 = ct{1629};
t4831 = ct{1630};
t4833 = ct{1631};
t4834 = ct{1632};
t4835 = ct{1633};
t4836 = ct{1634};
t4837 = ct{1635};
t4838 = ct{1636};
t4839 = ct{1637};
t4840 = ct{1638};
t4841 = ct{1639};
t4846 = ct{1640};
t4847 = ct{1641};
t4849 = ct{1642};
t4850 = ct{1643};
t4851 = ct{1644};
t4852 = ct{1645};
t4854 = ct{1646};
t4855 = ct{1647};
t4856 = ct{1648};
t4857 = ct{1649};
t4858 = ct{1650};
t486 = ct{1651};
t4860 = ct{1652};
t4861 = ct{1653};
t4862 = ct{1654};
t4865 = ct{1655};
t4866 = ct{1656};
t4867 = ct{1657};
t4868 = ct{1658};
t487 = ct{1659};
t4870 = ct{1660};
t4873 = ct{1661};
t4874 = ct{1662};
t4875 = ct{1663};
t4878 = ct{1664};
t4879 = ct{1665};
t488 = ct{1666};
t4880 = ct{1667};
t4881 = ct{1668};
t4883 = ct{1669};
t4884 = ct{1670};
t4885 = ct{1671};
t4886 = ct{1672};
t4887 = ct{1673};
t4888 = ct{1674};
t4889 = ct{1675};
t4890 = ct{1676};
t4891 = ct{1677};
t4892 = ct{1678};
t4894 = ct{1679};
t4895 = ct{1680};
t4899 = ct{1681};
t4900 = ct{1682};
t4901 = ct{1683};
t4902 = ct{1684};
t4904 = ct{1685};
t4905 = ct{1686};
t4906 = ct{1687};
t4913 = ct{1688};
t4914 = ct{1689};
t4915 = ct{1690};
t4916 = ct{1691};
t4917 = ct{1692};
t4918 = ct{1693};
t4919 = ct{1694};
t492 = ct{1695};
t4920 = ct{1696};
t4922 = ct{1697};
t4923 = ct{1698};
t4925 = ct{1699};
t4926 = ct{1700};
t4927 = ct{1701};
t4928 = ct{1702};
t4929 = ct{1703};
t493 = ct{1704};
t4930 = ct{1705};
t4931 = ct{1706};
t4933 = ct{1707};
t4934 = ct{1708};
t4935 = ct{1709};
t4936 = ct{1710};
t4938 = ct{1711};
t494 = ct{1712};
t4941 = ct{1713};
t4943 = ct{1714};
t4946 = ct{1715};
t4947 = ct{1716};
t495 = ct{1717};
t4950 = ct{1718};
t4951 = ct{1719};
t4953 = ct{1720};
t4954 = ct{1721};
t4956 = ct{1722};
t4957 = ct{1723};
t4958 = ct{1724};
t496 = ct{1725};
t4960 = ct{1726};
t4961 = ct{1727};
t4962 = ct{1728};
t4963 = ct{1729};
t4966 = ct{1730};
t4967 = ct{1731};
t497 = ct{1732};
t4971 = ct{1733};
t4972 = ct{1734};
t4973 = ct{1735};
t4974 = ct{1736};
t4975 = ct{1737};
t4976 = ct{1738};
t4977 = ct{1739};
t4981 = ct{1740};
t4982 = ct{1741};
t4983 = ct{1742};
t4985 = ct{1743};
t4986 = ct{1744};
t4987 = ct{1745};
t4988 = ct{1746};
t4989 = ct{1747};
t4991 = ct{1748};
t4992 = ct{1749};
t4993 = ct{1750};
t4994 = ct{1751};
t4995 = ct{1752};
t4996 = ct{1753};
t4d = ct{1754};
t4dd = ct{1755};
t50 = ct{1756};
t5000 = ct{1757};
t5001 = ct{1758};
t5004 = ct{1759};
t5006 = ct{1760};
t5007 = ct{1761};
t5008 = ct{1762};
t5009 = ct{1763};
t5010 = ct{1764};
t5011 = ct{1765};
t5012 = ct{1766};
t5013 = ct{1767};
t5014 = ct{1768};
t5016 = ct{1769};
t5017 = ct{1770};
t5018 = ct{1771};
t5019 = ct{1772};
t5020 = ct{1773};
t5022 = ct{1774};
t5024 = ct{1775};
t5025 = ct{1776};
t5026 = ct{1777};
t5027 = ct{1778};
t5028 = ct{1779};
t5029 = ct{1780};
t5030 = ct{1781};
t5038 = ct{1782};
t5040 = ct{1783};
t5041 = ct{1784};
t5043 = ct{1785};
t5044 = ct{1786};
t5045 = ct{1787};
t5046 = ct{1788};
t5048 = ct{1789};
t5049 = ct{1790};
t5050 = ct{1791};
t5051 = ct{1792};
t5057 = ct{1793};
t5058 = ct{1794};
t5062 = ct{1795};
t5066 = ct{1796};
t5068 = ct{1797};
t5069 = ct{1798};
t5070 = ct{1799};
t5071 = ct{1800};
t5072 = ct{1801};
t5073 = ct{1802};
t5074 = ct{1803};
t5075 = ct{1804};
t5076 = ct{1805};
t5077 = ct{1806};
t508 = ct{1807};
t5080 = ct{1808};
t5081 = ct{1809};
t5082 = ct{1810};
t5083 = ct{1811};
t5084 = ct{1812};
t5085 = ct{1813};
t5086 = ct{1814};
t5088 = ct{1815};
t5089 = ct{1816};
t5090 = ct{1817};
t5092 = ct{1818};
t5093 = ct{1819};
t5095 = ct{1820};
t5096 = ct{1821};
t5097 = ct{1822};
t5098 = ct{1823};
t51 = ct{1824};
t5101 = ct{1825};
t5102 = ct{1826};
t5104 = ct{1827};
t5105 = ct{1828};
t5110 = ct{1829};
t5117 = ct{1830};
t5119 = ct{1831};
t5125 = ct{1832};
t5126 = ct{1833};
t5127 = ct{1834};
t5130 = ct{1835};
t5131 = ct{1836};
t5132 = ct{1837};
t5134 = ct{1838};
t5135 = ct{1839};
t5139 = ct{1840};
t514 = ct{1841};
t5142 = ct{1842};
t5145 = ct{1843};
t5147 = ct{1844};
t5148 = ct{1845};
t515 = ct{1846};
t5152 = ct{1847};
t5154 = ct{1848};
t5156 = ct{1849};
t5158 = ct{1850};
t516 = ct{1851};
t5160 = ct{1852};
t5161 = ct{1853};
t5162 = ct{1854};
t5163 = ct{1855};
t5164 = ct{1856};
t5165 = ct{1857};
t5167 = ct{1858};
t5168 = ct{1859};
t5169 = ct{1860};
t5171 = ct{1861};
t5172 = ct{1862};
t5173 = ct{1863};
t5174 = ct{1864};
t5175 = ct{1865};
t5176 = ct{1866};
t5177 = ct{1867};
t5178 = ct{1868};
t5181 = ct{1869};
t5182 = ct{1870};
t5183 = ct{1871};
t5185 = ct{1872};
t5186 = ct{1873};
t519 = ct{1874};
t5190 = ct{1875};
t5191 = ct{1876};
t5192 = ct{1877};
t5193 = ct{1878};
t5194 = ct{1879};
t5195 = ct{1880};
t5196 = ct{1881};
t5197 = ct{1882};
t5198 = ct{1883};
t5199 = ct{1884};
t5201 = ct{1885};
t5202 = ct{1886};
t5213 = ct{1887};
t5218 = ct{1888};
t5219 = ct{1889};
t5220 = ct{1890};
t5222 = ct{1891};
t5225 = ct{1892};
t5226 = ct{1893};
t5227 = ct{1894};
t5228 = ct{1895};
t523 = ct{1896};
t5231 = ct{1897};
t5237 = ct{1898};
t5238 = ct{1899};
t5239 = ct{1900};
t524 = ct{1901};
t5240 = ct{1902};
t5241 = ct{1903};
t5242 = ct{1904};
t5243 = ct{1905};
t5246 = ct{1906};
t5247 = ct{1907};
t5248 = ct{1908};
t5252 = ct{1909};
t5253 = ct{1910};
t5254 = ct{1911};
t5255 = ct{1912};
t5256 = ct{1913};
t5257 = ct{1914};
t5261 = ct{1915};
t5264 = ct{1916};
t5265 = ct{1917};
t5266 = ct{1918};
t5267 = ct{1919};
t5268 = ct{1920};
t5271 = ct{1921};
t5272 = ct{1922};
t5273 = ct{1923};
t5277 = ct{1924};
t5280 = ct{1925};
t5283 = ct{1926};
t5284 = ct{1927};
t5285 = ct{1928};
t5287 = ct{1929};
t5288 = ct{1930};
t529 = ct{1931};
t5292 = ct{1932};
t5293 = ct{1933};
t5294 = ct{1934};
t5295 = ct{1935};
t5296 = ct{1936};
t5297 = ct{1937};
t5299 = ct{1938};
t53 = ct{1939};
t530 = ct{1940};
t5300 = ct{1941};
t5301 = ct{1942};
t5302 = ct{1943};
t5310 = ct{1944};
t5315 = ct{1945};
t5316 = ct{1946};
t5317 = ct{1947};
t5318 = ct{1948};
t5319 = ct{1949};
t532 = ct{1950};
t5320 = ct{1951};
t5321 = ct{1952};
t5322 = ct{1953};
t5323 = ct{1954};
t5324 = ct{1955};
t5326 = ct{1956};
t5327 = ct{1957};
t5329 = ct{1958};
t5331 = ct{1959};
t5335 = ct{1960};
t5336 = ct{1961};
t5337 = ct{1962};
t5338 = ct{1963};
t5343 = ct{1964};
t5344 = ct{1965};
t5345 = ct{1966};
t5349 = ct{1967};
t5351 = ct{1968};
t5355 = ct{1969};
t5356 = ct{1970};
t5357 = ct{1971};
t5359 = ct{1972};
t5360 = ct{1973};
t5361 = ct{1974};
t5363 = ct{1975};
t5366 = ct{1976};
t5367 = ct{1977};
t5369 = ct{1978};
t537 = ct{1979};
t5371 = ct{1980};
t5373 = ct{1981};
t5375 = ct{1982};
t5376 = ct{1983};
t5377 = ct{1984};
t5378 = ct{1985};
t5379 = ct{1986};
t5380 = ct{1987};
t5382 = ct{1988};
t5383 = ct{1989};
t5384 = ct{1990};
t5386 = ct{1991};
t5387 = ct{1992};
t5388 = ct{1993};
t5393 = ct{1994};
t5397 = ct{1995};
t5399 = ct{1996};
t5401 = ct{1997};
t5403 = ct{1998};
t5404 = ct{1999};
t5408 = ct{2000};
t5410 = ct{2001};
t5411 = ct{2002};
t5413 = ct{2003};
t5416 = ct{2004};
t5419 = ct{2005};
t5422 = ct{2006};
t5427 = ct{2007};
t5428 = ct{2008};
t543 = ct{2009};
t5431 = ct{2010};
t5432 = ct{2011};
t5433 = ct{2012};
t5434 = ct{2013};
t5435 = ct{2014};
t5437 = ct{2015};
t5438 = ct{2016};
t544 = ct{2017};
t5440 = ct{2018};
t5441 = ct{2019};
t5442 = ct{2020};
t5443 = ct{2021};
t5448 = ct{2022};
t5450 = ct{2023};
t5451 = ct{2024};
t5452 = ct{2025};
t5455 = ct{2026};
t546 = ct{2027};
t5465 = ct{2028};
t5469 = ct{2029};
t547 = ct{2030};
t5470 = ct{2031};
t5471 = ct{2032};
t5473 = ct{2033};
t5475 = ct{2034};
t5477 = ct{2035};
t548 = ct{2036};
t5481 = ct{2037};
t5482 = ct{2038};
t5484 = ct{2039};
t5485 = ct{2040};
t5486 = ct{2041};
t5487 = ct{2042};
t5491 = ct{2043};
t5492 = ct{2044};
t5494 = ct{2045};
t5498 = ct{2046};
t55 = ct{2047};
t5504 = ct{2048};
t5505 = ct{2049};
t5507 = ct{2050};
t5508 = ct{2051};
t5511 = ct{2052};
t5515 = ct{2053};
t552 = ct{2054};
t5523 = ct{2055};
t5525 = ct{2056};
t5529 = ct{2057};
t553 = ct{2058};
t5533 = ct{2059};
t5534 = ct{2060};
t554 = ct{2061};
t5542 = ct{2062};
t5543 = ct{2063};
t5550 = ct{2064};
t5552 = ct{2065};
t5556 = ct{2066};
t5557 = ct{2067};
t5558 = ct{2068};
t5560 = ct{2069};
t5561 = ct{2070};
t5562 = ct{2071};
t5572 = ct{2072};
t5583 = ct{2073};
t56 = ct{2074};
t5601 = ct{2075};
t5610 = ct{2076};
t5618 = ct{2077};
t5619 = ct{2078};
t562 = ct{2079};
t5622 = ct{2080};
t5625 = ct{2081};
t5626 = ct{2082};
t5627 = ct{2083};
t5629 = ct{2084};
t5638 = ct{2085};
t5668 = ct{2086};
t5675 = ct{2087};
t5685 = ct{2088};
t5686 = ct{2089};
t5687 = ct{2090};
t569 = ct{2091};
t5691 = ct{2092};
t5696 = ct{2093};
t57 = ct{2094};
t570 = ct{2095};
t5711 = ct{2096};
t5718 = ct{2097};
t5721 = ct{2098};
t5773 = ct{2099};
t5787 = ct{2100};
t58 = ct{2101};
t582 = ct{2102};
t588 = ct{2103};
t589 = ct{2104};
t591 = ct{2105};
t593 = ct{2106};
t598 = ct{2107};
t5d = ct{2108};
t5dd = ct{2109};
t601 = ct{2110};
t602 = ct{2111};
t604 = ct{2112};
t608 = ct{2113};
t609 = ct{2114};
t61 = ct{2115};
t614 = ct{2116};
t615 = ct{2117};
t616 = ct{2118};
t617 = ct{2119};
t623 = ct{2120};
t627 = ct{2121};
t63 = ct{2122};
t632 = ct{2123};
t637 = ct{2124};
t639 = ct{2125};
t641 = ct{2126};
t645 = ct{2127};
t646 = ct{2128};
t647 = ct{2129};
t648 = ct{2130};
t649 = ct{2131};
t650 = ct{2132};
t652 = ct{2133};
t653 = ct{2134};
t655 = ct{2135};
t659 = ct{2136};
t670 = ct{2137};
t675 = ct{2138};
t687 = ct{2139};
t69 = ct{2140};
t694 = ct{2141};
t695 = ct{2142};
t696 = ct{2143};
t698 = ct{2144};
t699 = ct{2145};
t6d = ct{2146};
t6dd = ct{2147};
t703 = ct{2148};
t705 = ct{2149};
t706 = ct{2150};
t71 = ct{2151};
t711 = ct{2152};
t720 = ct{2153};
t721 = ct{2154};
t723 = ct{2155};
t726 = ct{2156};
t729 = ct{2157};
t732 = ct{2158};
t733 = ct{2159};
t735 = ct{2160};
t736 = ct{2161};
t738 = ct{2162};
t739 = ct{2163};
t745 = ct{2164};
t746 = ct{2165};
t747 = ct{2166};
t748 = ct{2167};
t75 = ct{2168};
t752 = ct{2169};
t755 = ct{2170};
t759 = ct{2171};
t760 = ct{2172};
t761 = ct{2173};
t763 = ct{2174};
t764 = ct{2175};
t775 = ct{2176};
t776 = ct{2177};
t781 = ct{2178};
t785 = ct{2179};
t788 = ct{2180};
t789 = ct{2181};
t793 = ct{2182};
t8 = ct{2183};
t802 = ct{2184};
t806 = ct{2185};
t82 = ct{2186};
t820 = ct{2187};
t824 = ct{2188};
t828 = ct{2189};
t831 = ct{2190};
t833 = ct{2191};
t838 = ct{2192};
t842 = ct{2193};
t843 = ct{2194};
t844 = ct{2195};
t846 = ct{2196};
t853 = ct{2197};
t855 = ct{2198};
t859 = ct{2199};
t861 = ct{2200};
t865 = ct{2201};
t870 = ct{2202};
t871 = ct{2203};
t873 = ct{2204};
t879 = ct{2205};
t880 = ct{2206};
t884 = ct{2207};
t885 = ct{2208};
t890 = ct{2209};
t892 = ct{2210};
t896 = ct{2211};
t897 = ct{2212};
t9 = ct{2213};
t900 = ct{2214};
t909 = ct{2215};
t910 = ct{2216};
t919 = ct{2217};
t922 = ct{2218};
t923 = ct{2219};
t927 = ct{2220};
t928 = ct{2221};
t930 = ct{2222};
t932 = ct{2223};
t937 = ct{2224};
t943 = ct{2225};
t949 = ct{2226};
t952 = ct{2227};
t959 = ct{2228};
t961 = ct{2229};
t962 = ct{2230};
t963 = ct{2231};
t964 = ct{2232};
t965 = ct{2233};
t966 = ct{2234};
t969 = ct{2235};
t970 = ct{2236};
t972 = ct{2237};
t973 = ct{2238};
t982 = ct{2239};
t983 = ct{2240};
t5565 = t4060+t4314+t4315+t4730+t4744;
t5569 = -t2d.*(t4257+t4274-t5096+t14.*(t1862+t2375+t330.*(-t496-t547+t615+t623+t755+t8.*t37.*(t100-t364))+t2124.*(t100-t364)));
t5570 = -t3d.*(t4257+t4274-t5096+t14.*(t1862+t2375+t330.*(-t496-t547+t615+t623+t755+t8.*t37.*(t100-t364))+t2124.*(t100-t364)));
